simulink library "outp"  (R2021b)
settings: Solver=VariableStepAuto  StartTime=0.0  StopTime=10.0  RelTol=1e-3
undefined symbols (not defined in the file or in its folder): ENUM_PMMMODE_CHARGE, ENUM_PMMMODE_IDLE, ENUM_PMMMODE_INITIALIZE, ENUM_PMMMODE_POWERDOWN, ENUM_PMMMODE_SLEEP, Left, outp, slcm, TRUE
libraries: FVT_lib x1004, hcu_lib x4, simulink x1
(part 2 of 10)

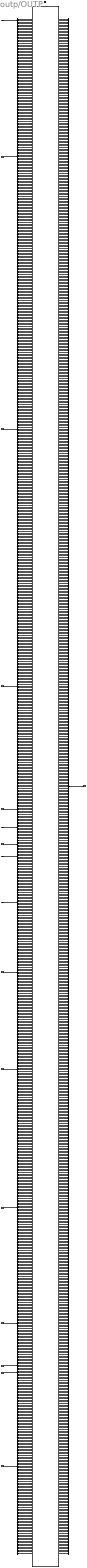
== system outp/OUTP ==
  BACC_outputs : Inport  OutDataTypeStr=Bus: BACC_outputs
  BAPM_outputs : Inport  Port=2  OutDataTypeStr=Bus: BAPM_outputs
  BBCM_outputs : Inport  Port=3  OutDataTypeStr=Bus: BBCM_outputs
  BDDM_outputs : Inport  Port=4  OutDataTypeStr=Bus: BDDM_outputs
  BDHP_outputs : Inport  Port=5  OutDataTypeStr=Bus: BDHP_outputs
  BDKC_outputs : Inport  Port=6  OutDataTypeStr=Bus: BDKC_outputs
  BDSC_outputs : Inport  Port=7  OutDataTypeStr=Bus: BDSC_outputs
  BNMM_outputs : Inport  Port=8  OutDataTypeStr=Bus: BNMM_outputs
  BPMM_outputs : Inport  Port=9  OutDataTypeStr=Bus: BPMM_outputs
  BSYS_outputs : Inport  Port=10  OutDataTypeStr=Bus: BSYS_outputs
  BTHC_outputs : Inport  Port=11  OutDataTypeStr=Bus: BTHC_outputs
  BTPM_outputs : Inport  Port=12  OutDataTypeStr=Bus: BTPM_outputs
  BTQD_outputs : Inport  Port=13  OutDataTypeStr=Bus: BTQD_outputs
  BTQR_outputs : Inport  Port=14  OutDataTypeStr=Bus: BTQR_outputs
  BV2L_outputs : Inport  Port=15  OutDataTypeStr=Bus: BV2L_outputs
  BVMC_outputs : Inport  Port=16  OutDataTypeStr=Bus: BVMC_outputs
  trig_OUTP : TriggerPort  TriggerType=function-call  VariantControl=(inherit)
  bus_creator : BusCreator  Inputs=1004
  bus_selector1 : BusSelector  OutputSignals=VACC_HVTHCMSysAvail_enum,VACC_LVBattVoltSta_enum,VACC_VehHVPwrAvail4THCM_W
  bus_selector10 : BusSelector  OutputSignals=VSYS_HWVer1_cnt,VSYS_HWVer2_cnt,VSYS_HWVer3_cnt,VSYS_CarModel1_cnt,VSYS_CarModel2_cnt,VSYS_CarModel3_cnt,VSYS_ECU1_cnt,VSYS_ECU2_cnt,VSYS_Major1_cnt,VSYS_Major2_cnt,VSYS_Minor1_cnt,VSYS_Minor2_cnt,VSYS_Patch1_cnt,VSYS_Patch2_cnt,VSYS_Country1_cnt,VSYS_Country2_cnt,VSYS_Variation_cnt,VSYS_Dash1_cnt,VSYS_Change1_cnt,VSYS_Change2_cnt,VSYS_Dash2_cnt,VSYS_SHA1_cnt,VSYS_SHA2_cnt,VSYS_SHA3_cnt,VSYS_SHA4_cnt,VSYS_SHA5_cnt,VSYS_SHA6_cnt,VSYS_SHA7_cnt,VSYS_SHA8_cnt,VSYS_NvWriteReqRisingEdge_flg,VSYS_FdcSlpReqRisingEdge_flg,VSYS_FdcSlpTime_sec,VSYS_PmicBootReason_enum,VSYS_WisrBootReason_raw32,VSYS_AcoreRebootCmdACK_flg,VSYS_CurrentNmState_enum,VSYS_ECUGen1_cnt,VSYS_ECUGen2_cnt,VSYS_PmicBootPath_raw32,VSYS_DrivingMode_cnt,VSYS_ModelYear_cnt,VSYS_Var4_cnt,VSYS_Var5_cnt
  bus_selector11 : BusSelector  OutputSignals=VTHC_FDCompCmd_rpm,VTHC_FDSOV1Cmd_flg,VTHC_FDSOV2Cmd_flg,VTHC_FDSOV3Cmd_flg,VTHC_FDEXV1Cmd_step,VTHC_FDEXV2Cmd_step,VTHC_FDSOTXVCmd_flg,VTHC_FDFWVCmd_flg,VTHC_FDTWVCmd_pct,VTHC_FDFrWPTCHeatPwrCmd_W,VTHC_CoolgFanActDuty_pct,VTHC_FDAGSCmd_enum,VTHC_FDEWP1Cmd_enum,VTHC_FDEWP2Cmd_enum,VTHC_FDEWP3Cmd_enum,VTHC_FDFrLeAPTCHeatPwrCmd_W,VTHC_FDFrRiAPTCHeatPwrCmd_W,VTHC_FDRrAPTCHeatPwrCmd_W,VTHC_FDBlowerCmd_pct,VTHC_BatteryMode_enum,VTHC_EDriveMode_enum,VTHC_CabinMode_enum,VTHC_CCUACLampSts_flg,VTHC_CCUAutoLampSts_flg,VTHC_CCUACMaxLampSts_flg,VTHC_CCUSyncLampSts_flg,VTHC_sigAirIntenZon1St_enum,VTHC_sigWindDirZon1St_enum,VTHC_sigRecircSt_flg,VTHC_sigSetTempZon1St_C,VTHC_sigSetTempZon2St_C,VTHC_sigClntTHvBattOut_C,VTHC_sigCbnSolarLeft_W,VTHC_sigClntTHvBattIn_C,VTHC_sigCbnSolarRight_W,VTHC_sigAmbAirT_C,VTHC_sigCbnAirT_C,VTHC_ACSubMode_enum,VTHC_FDRecyAutoCmd_enum,VTHC_ACModeMem_enum,VTHC_Face_flg,VTHC_Foot_flg,VTHC_Frost_flg,VTHC_FaceM_flg,VTHC_FootM_flg,VTHC_CCUSyncSts_flg,VTHC_ACForceOFF_flg,VTHC_RecAutoFlg_flg,VTHC_AirIntenZone1M_enum,VTHC_fdefog_flg,VTHC_sigSetTempZon2StM_C,VTHC_sigDfrstSt_flg,VTHC_FDCTHCAirIntZ3Sta_enum,VTHC_FDCTHCDrEVentModeSta_enum,VTHC_FDCTHCPsEVentModeSta_enum,VTHC_FDCTHCDrEVentZSta_enum,VTHC_FDCTHCCLEVentZSta_enum,VTHC_FDCTHCPsEVentZSta_enum,VTHC_FDCTHCCREVentZSta_enum,VTHC_FDCTHCDrEVentYSta_enum,VTHC_FDCTHCDrVentENSta_flg,VTHC_FDCTHCCLEVentYSta_enum,VTHC_FDCTHCCLVentENSta_flg,VTHC_FDCTHCPsEVentYSta_enum,VTHC_FDCTHCPsVentENSta_flg,VTHC_FDCTHCCREVentYSta_enum,VTHC_FDCTHCCRVentENSta_flg,VTHC_FDCTHCMAPTCForceOFFSta_flg,VTHC_DrVentEN_flg,VTHC_CLVentEN_flg,VTHC_PsVentEN_flg,VTHC_CRVentEN_flg,VTHC_FDCFGSAirIntSta_enum,VTHC_FDCFGSChSta_enum,VTHC_FDCFGSAirIntCmd_enum,VTHC_FDCFGSFuncSta_flg,VTHC_FDCFGSChCmd_enum,VTHC_FDCFGSIONSWSta_flg,VTHC_FDCFGSIONCmd_flg,VTHC_FDCFGSLearnCmd_enum,VTHC_FDCTHCMPreWPTCHeatSta_enum,VTHC_EWPBUflag1_flg,VTHC_EWPBUflag2_flg,VTHC_EWPBUflag3_flg
  bus_selector12 : BusSelector  OutputSignals=VTPM_LFBatWarn_flg,VTPM_RFBatWarn_flg,VTPM_LRBatWarn_flg,VTPM_RRBatWarn_flg,VTPM_LFWheelPress_raw8,VTPM_RFWheelPress_raw8,VTPM_LRWheelPress_raw8,VTPM_RRWheelPress_raw8,VTPM_LFWheelTemp_C,VTPM_RFWheelTemp_C,VTPM_LRWheelTemp_C,VTPM_RRWheelTemp_C,VTPM_LFSensorFail_flg,VTPM_RFSensorFail_flg,VTPM_LRSensorFail_flg,VTPM_RRSensorFail_flg,VTPM_LFWheelDebug_flg,VTPM_LRWheelDebug_flg,VTPM_RFWheelDebug_flg,VTPM_RRWheelDebug_flg,VTPM_TPMSResButtAllow_flg,VTPM_TPMSCaliButtAllow_flg,VTPM_LFPressIndi_enum,VTPM_RFPressIndi_enum,VTPM_LRPressIndi_enum,VTPM_RRPressIndi_enum,VTPM_TPMSWarnIndi_enum,VTPM_LFWheelTmpIndi_flg,VTPM_RFWheelTmpIndi_flg,VTPM_LRWheelTmpIndi_flg,VTPM_RRWheelTmpIndi_flg,VTPM_LFWheelPSW_raw8,VTPM_LRWheelPSW_raw8,VTPM_RFWheelPSW_raw8,VTPM_RRWheelPSW_raw8,VTPM_CWheelTips_enum,VTPM_AutoLTips_enum,VTPM_LFSensorMode_flg,VTPM_RFSensorMode_flg,VTPM_LRSensorMode_flg,VTPM_RRSensorMode_flg,VTPM_S1ID_raw32,VTPM_S2ID_raw32,VTPM_S3ID_raw32,VTPM_S4ID_raw32,VTPM_S1L_enum,VTPM_S2L_enum,VTPM_S3L_enum,VTPM_S4L_enum,VTPM_ALFin_flg,VTPM_LFP20_raw8,VTPM_RFP20_raw8,VTPM_LRP20_raw8,VTPM_RRP20_raw8,VTPM_FAT_flg,VTPM_IDin_raw32,VTPM_S1WheelDebugALTU_pct,VTPM_S2WheelDebugALTU_pct,VTPM_S3WheelDebugALTU_pct,VTPM_S4WheelDebugALTU_pct,VTPM_ID1messageALTU_raw8,VTPM_ID2messageALTU_raw8,VTPM_ID3messageALTU_raw8,VTPM_ID4messageALTU_raw8,VTPM_Chkfin_flg,VTPM_SetIDLoc_flg,VTPM_TPMSStorge_flg,VTPM_ChkStorge_flg,VTPM_TPMSResButt_flg,VTPM_LFPindi_enum,VTPM_RFPind_enum,VTPM_LRPindi_enum,VTPM_RRPindi_enum,VTPM_WriteChkLFID_raw,VTPM_WriteChkRFID_raw,VTPM_WriteChkLRID_raw,VTPM_WriteChkRRID_raw,VTPM_WriteChkfinLFID_raw,VTPM_WriteChkfinRFID_raw,VTPM_WriteChkfinLRID_raw,VTPM_WriteChkfinRRID_raw,VTPM_Flashchkdatavalid_enum,VTPM_Flashdatavalid_enum,VTPM_unlearnSfali_flg,VTPM_unlearnSfailvalid_enum,VTPM_Prepresstempvalid_enum,VTPM_FlashS1ID_raw,VTPM_FlashS2ID_raw,VTPM_FlashS3ID_raw,VTPM_FlashS4ID_raw,VTPM_FlashIDvalid_enum,VTPM_WritingCnt_enum,VTPM_TPMSTLCmd_flg,VTPM_LProgress_enum,VTPM_TPMSSensorIDRegStart_flg,VTPM_ModelVersion_raw,VTPM_ModelVersionChksum_raw
  bus_selector13 : BusSelector  OutputSignals=VTQD_ParkRequest_flg,VTQD_TqSourceFr_enum,VTQD_TqSourceRr_enum,VTQD_FrEDUAvailBrkRgnTq_Nm,VTQD_RrEDUAvailBrkRgnTq_Nm,VTQD_EVDriveMode_enum,VTQD_ShiftGearPosn_enum,VTQD_PButtonSta_enum,VTQD_FrActvDmpDisabReq_flg,VTQD_RrActvDmpDisabReq_flg,VTQD_FrRgnDecrSta_flg,VTQD_RrRgnDecrSta_flg,VTQD_DriverWhlTqDemFr_Nm,VTQD_DriverWhlTqDemRr_Nm,VTQD_FrEDUActTq_Nm,VTQD_RrEDUActTq_Nm,VTQD_FrEDURolRgnTq_Nm,VTQD_RrEDURolRgnTq_Nm,VTQD_FrEDUSpd_rpm,VTQD_RrEDUSpd_rpm,VTQD_FrEDUSpdValid_flg,VTQD_FrEDUAvailBrkRgnTqV_flg,VTQD_RrEDUSpdValid_flg,VTQD_RrEDUAvailBrkRgnTqV_flg,VTQD_RgnAbnorSta_flg,VTQD_PTCSPermSta_flg,VTQD_FrRgnPermSta_flg,VTQD_RrRgnPermSta_flg,VTQD_ExternalTqAllow_flg,VTQD_FrIdcMin_A,VTQD_FrIdcMax_A,VTQD_FrUdcMin_V,VTQD_FrUdcMax_V,VTQD_RrIdcMin_A,VTQD_RrIdcMax_A,VTQD_RrUdcMin_V,VTQD_RrUdcMax_V,VTQD_ReBrakeLPReq_flg,VTQD_ExtShftAllow_flg,VTQD_CreepON_flg,VTQD_EquivAccPedalSWSta_flg,VTQD_DriveProtEn_flg,VTQD_ActParkRequest_flg,VTQD_IVIPwrLockSta_enum,VTQD_ExtDoorAllow_flg,VTQD_OPDHoldLamp_flg,VTQD_SaveRegenMode_enum,VTQD_FDCVCURegenMode_enum,VTQD_SpdCtrlMode_enum,VTQD_SpdCtrlSta_flg,VTQD_SetSpd_kph,VTQD_VehActSpd_kph,VTQD_RegenLimIndSta_flg,VTQD_SetSpdLimWarn_flg
  bus_selector14 : BusSelector  OutputSignals=VTQR_FrTMTqReq_Nm,VTQR_RrTMTqReq_Nm
  bus_selector15 : BusSelector  OutputSignals=VV2L_ReqOBCV2LEna_enum,VV2L_ReqV2LIVIPopup_enum,VV2L_ReqV2LIVIDisChrg_enum,VV2L_ReqOBCExtrV2LEna_enum,VV2L_ReqOBCIntrV2LEna_enum,VV2L_HVPO120VGrpALDSt_enum,VV2L_HVPO120VGrpBLDSt_enum
  bus_selector16 : BusSelector  OutputSignals=VVMC_FeatSetSpdFinal_raw32,VVMC_VehicleSpeed_mph,VVMC_VehicleSpeed_kph,VVMC_MeterIndSpeed_raw32,VVMC_VMCAEBCtrlAvail_flg,VVMC_VMCACCCtrlAvail_flg,VVMC_VMCCCCtrlAvail_flg,VVMC_VMCMSACtrlAvail_flg,VVMC_FeatArbitrSta_enum,VVMC_FeatReqSpd_kph,VVMC_JerkPCT_pct,VVMC_LimitPCT_pct,VVMC_FrontRearSlipRatioCtrl_flg,VVMC_RearWhlSlipRatioCtrl_flg,VVMC_SingleWhlSlipRatioCtrl_flg,VVMC_LatAccCtrl_flg,VVMC_SafetyCtrl_flg,VVMC_SPD2ACCAct_flg,VVMC_AccCalcuPID_mps2,VVMC_ISOAccLimit_mps2,VVMC_ISODecLimit_mps2,VVMC_ISOJerkLimit_mps3,VVMC_ACCRequiredAccel_mps2,VVMC_DISCReqAcc_mps2,VVMC_FeatArbitrFinal_enum,VVMC_ActACCRequiredAccel_mps2,VVMC_LateralCtrl_flg,VVMC_ADASLKASta_enum,VVMC_LKAStrToqReq_Nm,VVMC_LKATOIFault_flg,VVMC_LKATOIAct_enum,VVMC_ADASAEBReq_enum,VVMC_ADASFaultSta_flg,VVMC_AEBVehHoldReq_flg,VVMC_ACCVehHoldReq_flg,VVMC_ADASDBSReq_enum,VVMC_ADASACCSta_enum,VVMC_ACCObjDist_m,VVMC_ACCObjRelSpd_mps,VVMC_TimeGapLevel_enum,VVMC_ACCJerkUpperLimit_mps3,VVMC_ACCComfortBandUpper_mps2,VVMC_ACCJerkLowerLimit_mps3,VVMC_ACCComfortBandLower_mps2,VVMC_ADASVehSpdLim_raw32,VVMC_ADASShftPosnReqA_flg,VVMC_ADASShftPosnReq_enum,VVMC_ADASForceIdle_flg,VVMC_HazardWarningReq_flg,VVMC_RightTurnLightReq_flg,VVMC_LeftTurnLightReq_flg,VVMC_ADASFCWSta_enum,VVMC_ADASLDWSta_enum,VVMC_ADASFltWrnReq_flg,VVMC_ACCObjDstLvl_enum,VVMC_ForceLowBeam_enum,VVMC_ACCTakeoverReq_flg,VVMC_ADASWarningMsg_enum,VVMC_ADASCAMSpdLim_enum,VVMC_TargetType_enum,VVMC_ADASSLIFSpdLim_enum,VVMC_LKAHODDisplayWarning_flg,VVMC_LKAHODSoundWarning_flg,VVMC_ADASLFCSta_enum,VVMC_ADASLaneModeL_enum,VVMC_ADASLaneModeR_enum,VVMC_ADASSLIFSta_enum,VVMC_ADASISASta_enum,VVMC_ADASLDWMute_flg,VVMC_ADASFCWMute_flg,VVMC_ADASLFCHandsOffWarning_enum,VVMC_LVDADisabled_flg,VVMC_LVDAMuteSta_enum,VVMC_LVDAFailinfo_flg,VVMC_LVDAWarning_flg,VVMC_LVDAACCStatusInformation_flg,VVMC_ADASLFCWarnSound_enum,VVMC_FCMACCmode_enum,VVMC_ADASLanetypeR_enum,VVMC_ADASLanetypeL_enum,VVMC_ADASLanecurveL_raw32,VVMC_ADASLanecurveR_raw32,VVMC_ADASAEBSta_enum,VVMC_FCMLDWRequest_enum,VVMC_FCMLDWFault_flg,VVMC_ACCCtrlAvail_flg,VVMC_ACCPedalOvrd_flg,VVMC_TimeGapCalcu_s,VVMC_CCCtrlSta_enum,VVMC_MSACtrlSta_enum,VVMC_APSCtrlAvail_flg,VVMC_APSActive_flg,VVMC_APSStaSys_enum,VVMC_APSDecReqA_flg,VVMC_APSDecReq_mps2,VVMC_APSReq_enum,VVMC_LongAcc_Gps,VVMC_CCMSASpdWar_flg,VVMC_IMUEnaCmd_flg,VVMC_CAASCtrlAvail_flg,VVMC_CAASActive_flg,VVMC_ExtraMSACtrlSta_enum,VVMC_CalibratedAccX_G,VVMC_CalibratedAccY_G,VVMC_CalibratedAccZ_G,VVMC_CalibratedGyroX_Dps,VVMC_CalibratedGyroY_Dps,VVMC_CalibratedGyroZ_Dps,VVMC_FDCVMCAPSVRqEPSCtrl_flg,VVMC_FDCVMCAPSAngleTarget_deg,VVMC_FDCVMCAPSRqEPSCtrl_flg,VVMC_FDCVMCAngCtrlTqWtGn_pct,VVMC_FDCVMCDrInpTqBstAct_flg,VVMC_FDCVMCMaxAngCtrlOutTqLim_Nm,VVMC_FDCVMCDrInpTqBstGn_pct
  bus_selector2 : BusSelector  OutputSignals=VAPM_VehSpeed_kph,VAPM_VehSpeedTimeOut_flg,VAPM_FSOffSw_enum,VAPM_FSOffSwTimeOut_flg,VAPM_ChrgPlugSta_enum,VAPM_PASDRMR_cm,VAPM_PASDRML_cm,VAPM_PASDRCR_cm,VAPM_PASDRCL_cm,VAPM_PASDFMR_cm,VAPM_PASDFML_cm,VAPM_PASDFCR_cm,VAPM_PASDFCL_cm,VAPM_APSDRLR_cm,VAPM_APSDRLL_cm,VAPM_APSDFLR_cm,VAPM_APSDFLL_cm,VAPM_PASAFCL_enum,VAPM_PASARMR_enum,VAPM_PASARML_enum,VAPM_PASARCR_enum,VAPM_PASARCL_enum,VAPM_PASAFMR_enum,VAPM_PASAFML_enum,VAPM_PASAFCR_enum,VAPM_USSStaRMR_flg,VAPM_USSStaRML_flg,VAPM_USSStaRLR_flg,VAPM_USSStaRLL_flg,VAPM_USSStaRCR_flg,VAPM_USSStaRCL_flg,VAPM_USSStaFMR_flg,VAPM_USSStaFML_flg,VAPM_USSStaFLR_flg,VAPM_USSStaFLL_flg,VAPM_USSStaFCR_flg,VAPM_USSStaFCL_flg,VAPM_Chime_enum,VAPM_SNSRLayout_enum,VAPM_StaFSya_flg,VAPM_ModOperation_enum,VAPM_BrkPedalPos_pct,VAPM_BrkPedalPosTimeOut_flg,VAPM_LFRawWhlSpeed_kph,VAPM_LFRawWhlSpeedTimeOut_flg,VAPM_RFRawWhlSpeed_kph,VAPM_RFRawWhlSpeedTimeOut_flg,VAPM_LRRawWhlSpeed_kph,VAPM_LRRawWhlSpeedTimeOut_flg,VAPM_RRRawWhlSpeed_kph,VAPM_RRRawWhlSpeedTimeOut_flg,VAPM_LFRawWhlSpeedV_flg,VAPM_LFRawWhlSpeedVTimeOut_flg,VAPM_RFRawWhlSpeedV_flg,VAPM_RFRawWhlSpeedVTimeOut_flg,VAPM_LRRawWhlSpeedV_flg,VAPM_LRRawWhlSpeedVTimeOut_flg,VAPM_RRRawWhlSpeedV_flg,VAPM_RRRawWhlSpeedVTimeOut_flg,VAPM_LFWhlRotDir_enum,VAPM_LFWhlRotDirTimeOut_flg,VAPM_RFWhlRotDir_enum,VAPM_RFWhlRotDirTimeOut_flg,VAPM_LRWhlRotDir_enum,VAPM_LRWhlRotDirTimeOut_flg,VAPM_RRWhlRotDir_enum,VAPM_RRWhlRotDirTimeOut_flg,VAPM_LFPulseCountV_flg,VAPM_LFPulseCountVTimeOut_flg,VAPM_RFPulseCountV_flg,VAPM_RFPulseCountVTimeOut_flg,VAPM_LRPulseCountV_flg,VAPM_LRPulseCountVTimeOut_flg,VAPM_RRPulseCountV_flg,VAPM_RRPulseCountVTimeOut_flg,VAPM_LFPulseCount_enum,VAPM_LFPulseCountTimeOut_flg,VAPM_RFPulseCount_enum,VAPM_RFPulseCountTimeOut_flg,VAPM_LRPulseCount_enum,VAPM_LRPulseCountTimeOut_flg,VAPM_RRPulseCount_enum,VAPM_RRPulseCountTimeOut_flg,VAPM_ShifterHandleCmd_enum,VAPM_ShifterHandleCmdTimeOut_flg,VAPM_DriIntend_enum,VAPM_DriIntendTimeOut_flg,VAPM_EPSAOIControl_enum,VAPM_EPSAOIControlTimeOut_flg,VAPM_SASAngle_Deg,VAPM_SASAngleTimeOut_flg,VAPM_SASSpeed_degps,VAPM_SASSpeedTimeOut_flg,VAPM_SASSpeedValid_flg,VAPM_SASSpeedValidTimeOut_flg,VAPM_SASCAL_flg,VAPM_SASCALTimeOut_flg,VAPM_SASV_flg,VAPM_SASVTimeOut_flg,VAPM_GRADE_Deg,VAPM_GRADETimeOut_flg,VAPM_YawRate_degps,VAPM_YawRateTimeOut_flg,VAPM_LatAccel_Gps,VAPM_LatAccelTimeOut_flg,VAPM_LongAccel_Gps,VAPM_LongAccelTimeOut_flg,VAPM_MCPressure_bar,VAPM_MCPressureTimeOut_flg,VAPM_YawRateV_flg,VAPM_YawRateVTimeOut_flg,VAPM_LatAccelV_flg,VAPM_LatAccelVTimeOut_flg,VAPM_LongAccelV_flg,VAPM_LongAccelVTimeOut_flg,VAPM_MCPressureV_bar,VAPM_MCPressureVTimeOut_flg,VAPM_BrkSwSta_flg,VAPM_BrkSwStaTimeOut_flg,VAPM_BrkSwV_flg,VAPM_BrkSwVTimeOut_flg,VAPM_ESCStandstill_flg,VAPM_ESCStandstillTimeOut_flg,VAPM_ESCAPSSta_enum,VAPM_ESCAPSStaTimeOut_flg,VAPM_EPBExtReleaseAvail_flg,VAPM_EPBExtReleaseAvailTimeOut_flg,VAPM_EPBExtApplyAvail_flg,VAPM_EPBExtApplyAvailTimeOut_flg,VAPM_EPBErrSta_enum,VAPM_EPBErrStaTimeOut_flg,VAPM_EPBSta_enum,VAPM_EPBStaTimeOut_flg,VAPM_AVMparkingcancel_enum,VAPM_AVMparkingcancelTimeOut_flg,VAPM_AVMparkingexcute_enum,VAPM_AVMparkingexcuteTimeOut_flg,VAPM_AVMParkingmode_enum,VAPM_AVMParkingmodeTimeOut_flg,VAPM_AVMErrSTA_flg,VAPM_AVMErrSTATimeOut_flg,VAPM_IVIStatus_flg,VAPM_IVIStatusTimeOut_flg,VAPM_CAASSw_enum,VAPM_CAASSwTimeOut_flg,VAPM_IVIScreen_enum,VAPM_IVIScreenTimeOut_flg,VAPM_ABSActive_flg,VAPM_ABSActiveTimeOut_flg,VAPM_TCSActive_flg,VAPM_TCSActiveTimeOut_flg,VAPM_DriverSeatBeltCmd_flg,VAPM_DriverSeatBeltCmdTimeOut_flg,VAPM_APSProgressPCT_pct,VAPM_APSRQDisplay_enum,VAPM_APSSWVer_enum,VAPM_APSHWVer_enum,VAPM_APSExitCondition_enum,VAPM_APSAngleTarget_Deg,VAPM_APSVRqEPASCtrl_flg,VAPM_APSRqEPASCtrl_flg,VAPM_CAASSta_enum,VAPM_DKCPDkeyAreaRAPSSta_enum,VAPM_DKCParkingModeCmd_enum,VAPM_PUIDLowPower_flg,VAPM_CAASVMCReqA_flg,VAPM_APSShiftPosnReq_enum,VAPM_APSSpeedCMD_kph,VAPM_APSVMCReqA_flg,VAPM_RAPSBCMLamp_enum,VAPM_RAPSBCMLockReq_flg,VAPM_APSPwrReq_enum,VAPM_RAPSErrWarnSta_enum,VAPM_RAPSErrLv1_flg,VAPM_IVIUserTakeOverAPSSta_flg
  bus_selector3 : BusSelector  OutputSignals=VBCM_AntitheftSta_enum,VBCM_TailgateRemote_enum,VBCM_HornCtrl_flg,VBCM_AllDoorSW_flg,VBCM_BCMDoorLockSta_flg,VBCM_AntitheftSeatFlod_flg,VBCM_HoodSW_flg,VBCM_TailgateSW_flg,VBCM_DrDoorSW_flg,VBCM_PsDoorSW_flg,VBCM_RLDoorSW_flg,VBCM_RRDoorSW_flg,VBCM_LockSetting_flg,VBCM_FrChargingDoorCtrl_enum,VBCM_RrChargingDoorCtrl_enum,VBCM_CrashDetd_flg,VBCM_CTDCtrl_enum,VBCM_DoorLockIND_flg,VBCM_CTDLockSW_flg,VBCM_Dimmer_pct,VBCM_DimmerEN_flg,VBCM_PosLamp_flg,VBCM_LBeam_flg,VBCM_HBeam_flg,VBCM_RrFogLamp_flg,VBCM_BrakeLamp_flg,VBCM_ReverseLamp_flg,VBCM_LDRL_flg,VBCM_RDRL_flg,VBCM_LBSD_flg,VBCM_RBSD_flg,VBCM_HazardSW_flg,VBCM_LTurnLP_flg,VBCM_RTurnLP_flg,VBCM_BCMBuzzerReq_flg,VBCM_MirrorCtrl_enum,VBCM_MirrorDefog_flg,VBCM_RrDefog_flg,VBCM_RoomLampH_flg,VBCM_RoomLampL_flg,VBCM_TrunkRel_flg,VBCM_TailgateHDSW_flg,VBCM_FrWiperL_flg,VBCM_FrWiperH_flg,VBCM_RrWiper_flg,VBCM_WasherCtrl_enum,VBCM_WiperFixMode_flg,VBCM_AmbLightBreath1_enum,VBCM_AmbLightBreath2_enum,VBCM_AmbLightBreath3_enum,VBCM_AmbLightBreath4_enum,VBCM_AmbLightBreath5_enum,VBCM_AmbLightBreath6_enum,VBCM_AmbLightBrightness1_enum,VBCM_AmbLightBrightness2_enum,VBCM_AmbLightBrightness3_enum,VBCM_AmbLightBrightness4_enum,VBCM_AmbLightBrightness5_enum,VBCM_AmbLightBrightness6_enum,VBCM_AmbLightColor1_enum,VBCM_AmbLightColor2_enum,VBCM_AmbLightColor3_enum,VBCM_AmbLightColor4_enum,VBCM_AmbLightColor5_enum,VBCM_AmbLightColor6_enum,VBCM_LampPwr_flg,VBCM_SPTGDet_flg,VBCM_APSOpenPTG_flg,VBCM_FollowMe_flg,VBCM_IVIRST_flg,VBCM_CountAlarm_enum,VBCM_MFSWTri_flg,VBCM_MirrorFlodPos_flg,VBCM_FuelDoorPos_flg,VBCM_MFRDNBrightReq_pct,VBCM_PTGInnerSW2_enum,VBCM_DrvWdwCtrlCmd_pct,VBCM_PasWdwCtrlCmd_pct,VBCM_DrRWdwCtrlCmd_pct,VBCM_PsRWdwCtrlCmd_pct,VBCM_APMDoorControlSta_flg,VBCM_AmbFunEN_flg,VBCM_AmbWelEN_flg,VBCM_AmbDimEN_flg,VBCM_AmbLinkDriSta_flg,VBCM_AmbPwrWarnEN_flg,VBCM_AmbODAEN_flg,VBCM_AmbColorSta_enum,VBCM_AmbBrightSta_enum,VBCM_LockAlarm_enum,VBCM_ATCtrl_enum,VBCM_fUnlockSingle_flg,VBCM_UserNow_enum,VBCM_AmbFunENFlash_enum,VBCM_AmbWelENFlash_enum,VBCM_AmbDimENFlash_enum,VBCM_AmbLinkDriStaFlash_enum,VBCM_AmbPwrWarnENFlash_enum,VBCM_AmbODAENFlash_enum,VBCM_AmbColorSta1_enum,VBCM_AmbColorSta2_enum,VBCM_AmbColorSta3_enum,VBCM_AmbColorSta4_enum,VBCM_AmbColorSta5_enum,VBCM_AmbColorSta7_enum,VBCM_AmbBrightnessSta1_enum,VBCM_AmbBrightnessSta2_enum,VBCM_AmbBrightnessSta3_enum,VBCM_AmbBrightnessSta4_enum,VBCM_AmbBrightnessSta5_enum,VBCM_AmbBrightnessSta7_enum,VBCM_HazardIND_flg,VBCM_DimSwSta_flg,VBCM_PassSWSta_flg,VBCM_FWipSwSta_enum,VBCM_FWasSwSta_enum,VBCM_TurnSwSta_enum,VBCM_TurnSwTSetSta_enum,VBCM_SPTGENFun_flg,VBCM_SPTGENFunMem_enum,VBCM_OutMode_enum,VBCM_TurnSwTimeSetSta123_enum,VBCM_TurnSwTimeSetSta457_enum,VBCM_FDLHandleLampCmd_flg,VBCM_FDRHandleLampCmd_flg,VBCM_FDHandleCmd_enum,VBCM_HBeamADB_flg,VBCM_WalkInUnLkENMem_enum,VBCM_WalkOutLkENMem_enum,VBCM_RmLpModeENMem_enum,VBCM_LockSettingStaMem_enum,VBCM_FollowMeENMem_enum,VBCM_WalkInUnLkENFunSta_flg,VBCM_WalkOutLkENFunSta_flg,VBCM_RmLpModeENFunSta_flg,VBCM_FollowMeENFunSta_flg,VBCM_HoodRelCmd_flg,VBCM_WelcomeLight_enum,VBCM_PTGOpenHeightSta_enum,VBCM_UserHeightSet_cnt,VBCM_PTGUserHeight1_cnt,VBCM_PTGUserHeight2_cnt,VBCM_PTGUserHeight3_cnt,VBCM_PTGUserHeight4_cnt,VBCM_PTGUserHeight5_cnt,VBCM_PTGUserHeight7_cnt,VBCM_PTGOpenHeight12_enum,VBCM_PTGOpenHeight34_enum,VBCM_PTGOpenHeight57_enum,VBCM_SenstivityPosnCmd_enum,VBCM_TimeGapLevelSta_enum,VBCM_ACCLevelMem12_enum,VBCM_ACCLevelMem34_enum,VBCM_ACCLevelMem57_enum,VBCM_LRightStaCmd_flg,VBCM_LLeftStaCmd_flg,VBCM_AutoLockSta_flg,VBCM_AutoLockMem_enum,VBCM_AutoUnlockSta_flg,VBCM_AutoUnlockMem_enum,VBCM_HMIKey1FuncSta_enum,VBCM_HMIKey2FuncSta_enum,VBCM_HMIKey3FuncSta_enum,VBCM_HMIKey4FuncSta_enum,VBCM_HMIKey5FuncSta_enum,VBCM_HMIKey6FuncSta_enum,VBCM_HMIKey7FuncSta_enum,VBCM_HMIKey8FuncSta_enum,VBCM_AutoWipHSpdENSta_flg,VBCM_DrvWdwReqAP_enum,VBCM_PasWdwReqAP_enum,VBCM_DrRWdwReqAP_enum,VBCM_PsRWdwReqAP_enum,VBCM_CLWinLockDrSta_flg,VBCM_CLWinLockDrStaMem_enum,VBCM_WinLFOpenedSta_pct,VBCM_WinRFOpenedSta_pct,VBCM_WinLROpenedSta_pct,VBCM_WinRROpenedSta_pct,VBCM_FoxPiSwitchSta_enum,VBCM_FoxPiLampSta_enum
  bus_selector4 : BusSelector  OutputSignals=VDDM_C3BMS6RCDTC_raw32,VDDM_C3BMS6CSDTC_raw32,VDDM_C3BMS6LCDTC_raw32,VDDM_C3BMS1RCDTC_raw32,VDDM_C3BMS1CSDTC_raw32,VDDM_C3BMS1LCDTC_raw32,VDDM_C3CCU1RCDTC_raw32,VDDM_C3CCU1CSDTC_raw32,VDDM_C3CCU1LCDTC_raw32,VDDM_C3CCU2RCDTC_raw32,VDDM_C3CCU2CSDTC_raw32,VDDM_C3CCU2LCDTC_raw32,VDDM_C1ABM1RCDTC_raw32,VDDM_C1ABM1CSDTC_raw32,VDDM_C1ABM1LCDTC_raw32,VDDM_Lv1ErrDTC_raw32,VDDM_Lv2ErrDTC_raw32,VDDM_Lv3ErrDTC_raw32,VDDM_Lv4ErrDTC_raw32,VDDM_BrkSWErrDTC_raw32,VDDM_BrkSWNoBacDTC_raw32,VDDM_KeyAuthDTC_raw32,VDDM_ONtoRdyDTC_raw32,VDDM_HVB4PreDTC_raw32,VDDM_MCU4PreDTC_raw32,VDDM_DCDC4PreDTC_raw32,VDDM_HVRlyCloDTC_raw32,VDDM_BMSRdyDTC_raw32,VDDM_DCDCEnaDTC_raw32,VDDM_HiLvSaChkDTC_raw32,VDDM_MidLvSaChkDTC_raw32,VDDM_MCUDisDTC_raw32,VDDM_DCDCDisDTC_raw32,VDDM_HVRlyOpDTC_raw32,VDDM_MCUActDTC_raw32,VDDM_OBC4PreDTC_raw32,VDDM_IniLVLoDTC_raw32,VDDM_LVSupLoDTC_raw32,VDDM_LVSupHiDTC_raw32,VDDM_DrStSWDTC_raw32,VDDM_FLDoorSWDTC_raw32,VDDM_RLDoorSWDTC_raw32,VDDM_FRDoorSWDTC_raw32,VDDM_RRDoorSWDTC_raw32,VDDM_HoodSWDTC_raw32,VDDM_TailgaSWDTC_raw32,VDDM_EDriveSysErrVCUErr_flg,VDDM_VehMalfunLevel_enum,VDDM_APS1SigOoRDTC_raw32,VDDM_APS2SigOoRDTC_raw32,VDDM_APSCorrErrDTC_raw32,VDDM_MCUF1NoComDTC_raw32,VDDM_MCUR1NoComDTC_raw32,VDDM_Shifter1NoComDTC_raw32,VDDM_ESC7NoComDTC_raw32,VDDM_ESC1NoComDTC_raw32,VDDM_ESC5NoComDTC_raw32,VDDM_EnterNewOperCyc_flg,VDDM_DiagHCrashDTC_raw32,VDDM_DiagFLTSDTC_raw32,VDDM_DiagFRTSDTC_raw32,VDDM_DiagRLTSDTC_raw32,VDDM_DiagRRTSDTC_raw32,VDDM_FCLUSSDTC_raw32,VDDM_FMLUSSDTC_raw32,VDDM_FMRUSSDTC_raw32,VDDM_FCRUSSDTC_raw32,VDDM_RCLUSSDTC_raw32,VDDM_RMLUSSDTC_raw32,VDDM_RMRUSSDTC_raw32,VDDM_RCRUSSDTC_raw32,VDDM_FLLUSSDTC_raw32,VDDM_FLRUSSDTC_raw32,VDDM_RLLUSSDTC_raw32,VDDM_RLRUSSDTC_raw32,VDDM_FCM2NoComDTC_raw32,VDDM_FCM2RCErrDTC_raw32,VDDM_FCM2CSErrDTC_raw32,VDDM_FCM3NoComDTC_raw32,VDDM_FCM3RCErrDTC_raw32,VDDM_FCM3CSErrDTC_raw32,VDDM_FCM4NoComDTC_raw32,VDDM_FCM4CSErrDTC_raw32,VDDM_FCM5NoComDTC_raw32,VDDM_FCM5CSErrDTC_raw32,VDDM_ZoneSCPNoComDTC_raw32,VDDM_BMSSigErrDetDTC_raw32,VDDM_FCMACCSigErrDetDTC_raw32,VDDM_FrMCUSigErrDetDTC_raw32,VDDM_RrMCUSigErrDetDTC_raw32,VDDM_CCUSigErrDetDTC_raw32,VDDM_ACCAccelCmdErrDetDTC_raw32,VDDM_ACCMalfuncDetDTC_raw32,VDDM_CCMalfuncDetDTC_raw32,VDDM_MSAMalfuncDetDTC_raw32,VDDM_ISAMalfuncDetDTC_raw32,VDDM_MCUF1RCErrDTC_raw32,VDDM_MCUR1RCErrDTC_raw32,VDDM_MCUF1CSErrDTC_raw32,VDDM_MCUR1CSErrDTC_raw32,VDDM_Shifter1RCErrDTC_raw32,VDDM_Shifter1CSErrDTC_raw32,VDDM_ESC7RCErrDTC_raw32,VDDM_ESC7CSErrDTC_raw32,VDDM_ESC1RCErrDTC_raw32,VDDM_ESC1CSErrDTC_raw32,VDDM_ESC5RCErrDTC_raw32,VDDM_ESC5CSErrDTC_raw32,VDDM_FrMCUTqErrDTC_raw32,VDDM_RrMCUTqErrDTC_raw32,VDDM_LFBatwarnDTC_raw32,VDDM_RFBatwarnDTC_raw32,VDDM_LRBatwarnDTC_raw32,VDDM_RRBatwarnDTC_raw32,VDDM_LFPressIndiDTC_raw32,VDDM_RFPressIndiDTC_raw32,VDDM_LRPressIndiDTC_raw32,VDDM_RRPressIndiDTC_raw32,VDDM_LFWheelTmpHighDTC_raw32,VDDM_RFWheelTmpHighDTC_raw32,VDDM_LRWheelTmpHighDTC_raw32,VDDM_RRWheelTmpHighDTC_raw32,VDDM_LFSensorFailDTC_raw32,VDDM_RFSensorFailDTC_raw32,VDDM_LRSensorFailDTC_raw32,VDDM_RRSensorFailDTC_raw32,VDDM_C1EPAS2LCDTC_raw32,VDDM_5vAPS1PwrErrDTC_raw32,VDDM_5vAPS2PwrErrDTC_raw32,VDDM_EPBLockTODTC_raw32,VDDM_EPBUnlockTODTC_raw32,VDDM_LimpHomeActTmp_flg,VDDM_DTCDetect_enum,VDDM_EngagePFail_flg,VDDM_DisengagePFail_flg,VDDM_VCURAPSErrLv2_flg,VDDM_VCURAPSErrLv3_flg,VDDM_EDriveSysErrShifterErr_flg,VDDM_LVSysErrPwrOutErr_flg,VDDM_HVRlyOpFail_flg,VDDM_MCUActDisFail_flg,VDDM_VCUBrkSWSta_enum,VDDM_VCUFLDoorSta_flg,VDDM_VCUFRDoorSta_flg,VDDM_VCURLDoorSta_flg,VDDM_VCURRDoorSta_flg,VDDM_SysAllowReadySta_flg,VDDM_VCUHoodSWSta_flg,VDDM_VCUTailgateSWSta_flg,VDDM_CAN1BusErrorDTC_raw32,VDDM_CAN2BusErrorDTC_raw32,VDDM_CAN3BusErrorDTC_raw32,VDDM_CAN4BusErrorDTC_raw32,VDDM_CAN5BusErrorDTC_raw32,VDDM_CAN6BusErrorDTC_raw32
  bus_selector5 : BusSelector  OutputSignals=VDHP_ActAPSPosn_pct,VDHP_EAPS1MIN_pct,VDHP_EAPS2MIN_pct,VDHP_ResetPedalZeroPosStart_flg,VDHP_EAPS1NRM_pct,VDHP_EAPS2NRM_pct
  bus_selector6 : BusSelector  OutputSignals=VDKC_DKCTimeSN_cnt,VDKC_DKCAuthSta_enum,VDKC_TimeSNDKCFbk_cnt,VDKC_KeyMissSta_flg,VDKC_KeyModeSta_enum,VDKC_DkeyShowIVISta_enum,VDKC_KeyAreaPS_enum,VDKC_KeyAreaLockUnlock_enum,VDKC_PCommandToBCM_enum,VDKC_DKeyWelcomeSta_enum,VDKC_KeyAreaPTG_enum,VDKC_KeyAreaSPTGSta_enum,VDKC_UIDLowPowerSta_enum,VDKC_DkeyAreaRAPSSta_enum,VDKC_ParkingModeCmd_enum,VDKC_KeyNumSta_enum,VDKC_KeyTypeSta_enum,VDKC_FDCDKCAllowSleep_flg
  bus_selector7 : BusSelector  OutputSignals=VDSC_DISCTurn_flg,VDSC_DISCTargetSpd_kph,VDSC_DISCSta_enum,VDSC_DISCButtSta_flg
  bus_selector8 : BusSelector  OutputSignals=VNMM_AllCANTxReq_flg,VNMM_NMmTxReq_flg,VNMM_Awake_enum,VNMM_CSB_flg,VNMM_ErrorState_enum,VNMM_NodeID_enum,VNMM_PNI_flg,VNMM_RptMsgReq_flg,VNMM_WakeUp_enum,VNMM_ActiveWU_flg,VNMM_SysNMmSta_enum,VNMM_NetworkReq_flg
  bus_selector9 : BusSelector  OutputSignals=VPMM_PowerUpState_enum,VPMM_PowerDownState_enum,VPMM_PowerUpFault_enum,VPMM_PowerDownFault_enum,VPMM_ActiveDischargeReq_flg,VPMM_DCDCEnaReq_flg,VPMM_DCDCVoltSetpoint_V,VPMM_HVBatCnctReq_flg,VPMM_HVSysReadyToCharge_enum,VPMM_PowerSta_enum,VPMM_LVPwrSta_flg,VPMM_HVPwrSta_flg,VPMM_SysPowerMode_enum,VPMM_FrMCUEnaReq_flg,VPMM_RrMCUEnaReq_flg,VPMM_DrivetrainSelect_enum,VPMM_DrSeatSta_enum,VPMM_PwrStaSelect_enum,VPMM_PwrStaConstraint_enum,VPMM_TCountSta_enum,VPMM_PwrUpReq_enum,VPMM_PwrDownReq_enum,VPMM_LowSOCWarn_enum,VPMM_ReVehThdChkSta_enum,VPMM_EvccAplusPwrUpReq_flg,VPMM_PwrStaONTOPopReq_flg,VPMM_IVIPwrStaONTOPopT_s,VPMM_LVChrgHoldTtimer_s,VPMM_LVBattChrgTimeCnt_s,VPMM_SilentChkAllowSleep_flg,VPMM_TimerAllowSleep_flg,VPMM_FDADC12VDetAvg_mV,VPMM_PMMAllowECUSleep_flg,VPMM_LVSilentChrgSta_enum,VPMM_LVSilentChrgReq_flg,VPMM_LVSilentChrgLv_enum,VPMM_CtrlFrPwrStbA1P_flg,VPMM_CtrlFrRC1_flg,VPMM_CtrlFrBMSCCUCIR_flg,VPMM_CtrlFrEDUINVERTER_flg,VPMM_HWResetSta_enum,VPMM_CtrlDrPwrStbA2_flg,VPMM_PwrStaTOSta_enum,VPMM_Sched_ChgTOSta_enum,VPMM_PwrReq_OTA_enum,VPMM_OTAPwrReqOFFChkSta_enum,VPMM_OTAPwrReqStdChkSta_enum,VPMM_PwrReqRAPSAvail_flg
  outpmodule : Subsystem
  BOUTP_outputs : Outport  OutDataTypeStr=Bus: BOUTP_outputs
  wires:
  bus_selector9/42 -> outpmodule/596(VPMM_CtrlDrPwrStbA2_flg)  "<VPMM_CtrlDrPwrStbA2_flg>"
  bus_selector9/39 -> outpmodule/593(VPMM_CtrlFrBMSCCUCIR_flg)  "<VPMM_CtrlFrBMSCCUCIR_flg>"
  bus_selector9/36 -> outpmodule/590(VPMM_LVSilentChrgLv_enum)  "<VPMM_LVSilentChrgLv_enum>"
  bus_selector9/35 -> outpmodule/589(VPMM_LVSilentChrgReq_flg)  "<VPMM_LVSilentChrgReq_flg>"
  bus_selector9/29 -> outpmodule/583(VPMM_LVBattChrgTimeCnt_s)  "<VPMM_LVBattChrgTimeCnt_s>"
  bus_selector9/26 -> outpmodule/580(VPMM_PwrStaONTOPopReq_flg)  "<VPMM_PwrStaONTOPopReq_flg>"
  bus_selector9/27 -> outpmodule/581(VPMM_IVIPwrStaONTOPopT_s)  "<VPMM_IVIPwrStaONTOPopT_s>"
  bus_selector9/20 -> outpmodule/574(VPMM_TCountSta_enum)  "<VPMM_TCountSta_enum>"
  bus_selector9/22 -> outpmodule/576(VPMM_PwrDownReq_enum)  "<VPMM_PwrDownReq_enum>"
  bus_selector9/21 -> outpmodule/575(VPMM_PwrUpReq_enum)  "<VPMM_PwrUpReq_enum>"
  bus_selector9/18 -> outpmodule/572(VPMM_PwrStaSelect_enum)  "<VPMM_PwrStaSelect_enum>"
  bus_selector9/17 -> outpmodule/571(VPMM_DrSeatSta_enum)  "<VPMM_DrSeatSta_enum>"
  bus_selector9/13 -> outpmodule/567(VPMM_SysPowerMode_enum)  "<VPMM_SysPowerMode_enum>"
  bus_selector9/10 -> outpmodule/564(VPMM_PowerSta_enum)  "<VPMM_PowerSta_enum>"
  bus_selector9/11 -> outpmodule/565(VPMM_LVPwrSta_flg)  "<VPMM_LVPwrSta_flg>"
  bus_selector9/9 -> outpmodule/563(VPMM_HVSysReadyToCharge_enum)  "<VPMM_HVSysReadyToCharge_enum>"
  bus_selector9/7 -> outpmodule/561(VPMM_DCDCVoltSetpoint_V)  "<VPMM_DCDCVoltSetpoint_V>"
  bus_selector9/8 -> outpmodule/562(VPMM_HVBatCnctReq_flg)  "<VPMM_HVBatCnctReq_flg>"
  BPMM_outputs/1 -> bus_selector9/1
  bus_selector9/6 -> outpmodule/560(VPMM_DCDCEnaReq_flg)  "<VPMM_DCDCEnaReq_flg>"
  bus_selector9/4 -> outpmodule/558(VPMM_PowerDownFault_enum)  "<VPMM_PowerDownFault_enum>"
  bus_selector9/2 -> outpmodule/556(VPMM_PowerDownState_enum)  "<VPMM_PowerDownState_enum>"
  bus_selector9/1 -> outpmodule/555(VPMM_PowerUpState_enum)  "<VPMM_PowerUpState_enum>"
  bus_selector8/7 -> outpmodule/549(VNMM_PNI_flg)  "<VNMM_PNI_flg>"
  bus_selector8/8 -> outpmodule/550(VNMM_RptMsgReq_flg)  "<VNMM_RptMsgReq_flg>"
  bus_selector8/10 -> outpmodule/552(VNMM_ActiveWU_flg)  "<VNMM_ActiveWU_flg>"
  bus_selector16/85 -> outpmodule/974(VVMC_FCMLDWFault_flg)  "<VVMC_FCMLDWFault_flg>"
  bus_selector16/84 -> outpmodule/973(VVMC_FCMLDWRequest_enum)  "<VVMC_FCMLDWRequest_enum>"
  bus_selector16/81 -> outpmodule/970(VVMC_ADASLanecurveL_raw32)  "<VVMC_ADASLanecurveL_raw32>"
  bus_selector16/83 -> outpmodule/972(VVMC_ADASAEBSta_enum)  "<VVMC_ADASAEBSta_enum>"
  bus_selector16/80 -> outpmodule/969(VVMC_ADASLanetypeL_enum)  "<VVMC_ADASLanetypeL_enum>"
  bus_selector16/76 -> outpmodule/965(VVMC_LVDAACCStatusInformation_flg)  "<VVMC_LVDAACCStatusInformation_flg>"
  bus_selector16/77 -> outpmodule/966(VVMC_ADASLFCWarnSound_enum)  "<VVMC_ADASLFCWarnSound_enum>"
  bus_selector16/71 -> outpmodule/960(VVMC_ADASLFCHandsOffWarning_enum)  "<VVMC_ADASLFCHandsOffWarning_enum>"
  bus_selector16/69 -> outpmodule/958(VVMC_ADASLDWMute_flg)  "<VVMC_ADASLDWMute_flg>"
  bus_selector16/65 -> outpmodule/954(VVMC_ADASLaneModeL_enum)  "<VVMC_ADASLaneModeL_enum>"
  bus_selector16/62 -> outpmodule/951(VVMC_LKAHODDisplayWarning_flg)  "<VVMC_LKAHODDisplayWarning_flg>"
  bus_selector16/55 -> outpmodule/944(VVMC_ACCObjDstLvl_enum)  "<VVMC_ACCObjDstLvl_enum>"
  bus_selector16/50 -> outpmodule/939(VVMC_RightTurnLightReq_flg)  "<VVMC_RightTurnLightReq_flg>"
  bus_selector9/43 -> outpmodule/597(VPMM_PwrStaTOSta_enum)  "<VPMM_PwrStaTOSta_enum>"
  bus_selector16/49 -> outpmodule/938(VVMC_HazardWarningReq_flg)  "<VVMC_HazardWarningReq_flg>"
  bus_selector16/47 -> outpmodule/936(VVMC_ADASShftPosnReq_enum)  "<VVMC_ADASShftPosnReq_enum>"
  bus_selector16/45 -> outpmodule/934(VVMC_ADASVehSpdLim_raw32)  "<VVMC_ADASVehSpdLim_raw32>"
  bus_selector16/36 -> outpmodule/925(VVMC_ADASDBSReq_enum)  "<VVMC_ADASDBSReq_enum>"
  bus_selector16/35 -> outpmodule/924(VVMC_ACCVehHoldReq_flg)  "<VVMC_ACCVehHoldReq_flg>"
  bus_selector16/31 -> outpmodule/920(VVMC_LKATOIAct_enum)  "<VVMC_LKATOIAct_enum>"
  bus_selector16/32 -> outpmodule/921(VVMC_ADASAEBReq_enum)  "<VVMC_ADASAEBReq_enum>"
  bus_selector16/28 -> outpmodule/917(VVMC_ADASLKASta_enum)  "<VVMC_ADASLKASta_enum>"
  bus_selector16/26 -> outpmodule/915(VVMC_ActACCRequiredAccel_mps2)  "<VVMC_ActACCRequiredAccel_mps2>"
  bus_selector16/23 -> outpmodule/912(VVMC_ACCRequiredAccel_mps2)  "<VVMC_ACCRequiredAccel_mps2>"
  bus_selector16/19 -> outpmodule/908(VVMC_AccCalcuPID_mps2)  "<VVMC_AccCalcuPID_mps2>"
  bus_selector16/11 -> outpmodule/900(VVMC_JerkPCT_pct)  "<VVMC_JerkPCT_pct>"
  bus_selector16/7 -> outpmodule/896(VVMC_VMCCCCtrlAvail_flg)  "<VVMC_VMCCCCtrlAvail_flg>"
  bus_selector16/9 -> outpmodule/898(VVMC_FeatArbitrSta_enum)  "<VVMC_FeatArbitrSta_enum>"
  bus_selector16/5 -> outpmodule/894(VVMC_VMCAEBCtrlAvail_flg)  "<VVMC_VMCAEBCtrlAvail_flg>"
  bus_selector16/4 -> outpmodule/893(VVMC_MeterIndSpeed_raw32)  "<VVMC_MeterIndSpeed_raw32>"
  bus_selector16/101 -> outpmodule/990(VVMC_CAASActive_flg)  "<VVMC_CAASActive_flg>"
  bus_selector16/99 -> outpmodule/988(VVMC_IMUEnaCmd_flg)  "<VVMC_IMUEnaCmd_flg>"
  bus_selector16/98 -> outpmodule/987(VVMC_CCMSASpdWar_flg)  "<VVMC_CCMSASpdWar_flg>"
  bus_selector16/91 -> outpmodule/980(VVMC_APSCtrlAvail_flg)  "<VVMC_APSCtrlAvail_flg>"
  bus_selector16/90 -> outpmodule/979(VVMC_MSACtrlSta_enum)  "<VVMC_MSACtrlSta_enum>"
  outpmodule/1004(VOUTP_FDCVMCDrInpTqBstGn_pct) -> bus_creator/1004
  outpmodule/998(VOUTP_FDCVMCAPSVRqEPSCtrl_flg) -> bus_creator/998
  outpmodule/997(VOUTP_CalibratedGyroZ_Dps) -> bus_creator/997
  bus_selector8/5 -> outpmodule/547(VNMM_ErrorState_enum)  "<VNMM_ErrorState_enum>"
  outpmodule/992(VOUTP_CalibratedAccX_G) -> bus_creator/992
  outpmodule/989(VOUTP_CAASCtrlAvail_flg) -> bus_creator/989
  bus_selector16/97 -> outpmodule/986(VVMC_LongAcc_Gps)  "<VVMC_LongAcc_Gps>"
  outpmodule/988(VOUTP_IMUEnaCmd_flg) -> bus_creator/988
  outpmodule/982(VOUTP_APSStaSys_enum) -> bus_creator/982
  outpmodule/983(VOUTP_APSDecReqA_flg) -> bus_creator/983
  outpmodule/975(VOUTP_ACCCtrlAvail_flg) -> bus_creator/975
  outpmodule/974(VOUTP_FCMLDWFault_flg) -> bus_creator/974
  bus_selector9/3 -> outpmodule/557(VPMM_PowerUpFault_enum)  "<VPMM_PowerUpFault_enum>"
  outpmodule/969(VOUTP_ADASLanetypeL_enum) -> bus_creator/969
  outpmodule/970(VOUTP_ADASLanecurveL_raw32) -> bus_creator/970
  outpmodule/966(VOUTP_ADASLFCWarnSound_enum) -> bus_creator/966
  outpmodule/968(VOUTP_ADASLanetypeR_enum) -> bus_creator/968
  outpmodule/964(VOUTP_LVDAWarning_flg) -> bus_creator/964
  outpmodule/965(VOUTP_LVDAACCStatusInformation_flg) -> bus_creator/965
  bus_selector4/140 -> outpmodule/499(VDDM_HVRlyOpFail_flg)  "<VDDM_HVRlyOpFail_flg>"
  bus_selector9/46 -> outpmodule/600(VPMM_OTAPwrReqOFFChkSta_enum)  "<VPMM_OTAPwrReqOFFChkSta_enum>"
  outpmodule/285(VOUTP_AmbBrightnessSta2_enum) -> bus_creator/285
  outpmodule/282(VOUTP_AmbColorSta5_enum) -> bus_creator/282
  outpmodule/278(VOUTP_AmbColorSta1_enum) -> bus_creator/278
  outpmodule/276(VOUTP_AmbPwrWarnENFlash_enum) -> bus_creator/276
  outpmodule/274(VOUTP_AmbDimENFlash_enum) -> bus_creator/274
  outpmodule/270(VOUTP_fUnlockSingle_flg) -> bus_creator/270
  bus_selector16/72 -> outpmodule/961(VVMC_LVDADisabled_flg)  "<VVMC_LVDADisabled_flg>"
  outpmodule/272(VOUTP_AmbFunENFlash_enum) -> bus_creator/272
  outpmodule/271(VOUTP_UserNow_enum) -> bus_creator/271
  outpmodule/269(VOUTP_ATCtrl_enum) -> bus_creator/269
  outpmodule/264(VOUTP_AmbPwrWarnEN_flg) -> bus_creator/264
  outpmodule/262(VOUTP_AmbDimEN_flg) -> bus_creator/262
  outpmodule/261(VOUTP_AmbWelEN_flg) -> bus_creator/261
  outpmodule/258(VOUTP_PsRWdwCtrlCmd_pct) -> bus_creator/258
  outpmodule/257(VOUTP_DrRWdwCtrlCmd_pct) -> bus_creator/257
  outpmodule/249(VOUTP_CountAlarm_enum) -> bus_creator/249
  outpmodule/247(VOUTP_FollowMe_flg) -> bus_creator/247
  outpmodule/244(VOUTP_LampPwr_flg) -> bus_creator/244
  outpmodule/1000(VOUTP_FDCVMCAPSRqEPSCtrl_flg) -> bus_creator/1000
  outpmodule/245(VOUTP_SPTGDet_flg) -> bus_creator/245
  outpmodule/243(VOUTP_AmbLightColor6_enum) -> bus_creator/243
  outpmodule/239(VOUTP_AmbLightColor2_enum) -> bus_creator/239
  outpmodule/237(VOUTP_AmbLightBrightness6_enum) -> bus_creator/237
  outpmodule/236(VOUTP_AmbLightBrightness5_enum) -> bus_creator/236
  outpmodule/233(VOUTP_AmbLightBrightness2_enum) -> bus_creator/233
  outpmodule/305(VOUTP_HBeamADB_flg) -> bus_creator/305
  outpmodule/298(VOUTP_SPTGENFunMem_enum) -> bus_creator/298
  outpmodule/296(VOUTP_TurnSwTSetSta_enum) -> bus_creator/296
  outpmodule/297(VOUTP_SPTGENFun_flg) -> bus_creator/297
  outpmodule/295(VOUTP_TurnSwSta_enum) -> bus_creator/295
  outpmodule/288(VOUTP_AmbBrightnessSta5_enum) -> bus_creator/288
  outpmodule/290(VOUTP_HazardIND_flg) -> bus_creator/290
  bus_selector2/93 -> outpmodule/96(VAPM_SASSpeedTimeOut_flg)  "<VAPM_SASSpeedTimeOut_flg>"
  bus_selector2/76 -> outpmodule/79(VAPM_LFPulseCount_enum)  "<VAPM_LFPulseCount_enum>"
  bus_selector2/85 -> outpmodule/88(VAPM_ShifterHandleCmdTimeOut_flg)  "<VAPM_ShifterHandleCmdTimeOut_flg>"
  bus_selector3/180 -> outpmodule/358(VBCM_FoxPiSwitchSta_enum)  "<VBCM_FoxPiSwitchSta_enum>"
  bus_selector3/181 -> outpmodule/359(VBCM_FoxPiLampSta_enum)  "<VBCM_FoxPiLampSta_enum>"
  bus_selector3/178 -> outpmodule/356(VBCM_WinLROpenedSta_pct)  "<VBCM_WinLROpenedSta_pct>"
  bus_selector3/175 -> outpmodule/353(VBCM_CLWinLockDrStaMem_enum)  "<VBCM_CLWinLockDrStaMem_enum>"
  bus_selector3/171 -> outpmodule/349(VBCM_PasWdwReqAP_enum)  "<VBCM_PasWdwReqAP_enum>"
  bus_selector9/23 -> outpmodule/577(VPMM_LowSOCWarn_enum)  "<VPMM_LowSOCWarn_enum>"
  bus_selector3/169 -> outpmodule/347(VBCM_AutoWipHSpdENSta_flg)  "<VBCM_AutoWipHSpdENSta_flg>"
  bus_selector3/170 -> outpmodule/348(VBCM_DrvWdwReqAP_enum)  "<VBCM_DrvWdwReqAP_enum>"
  outpmodule/971(VOUTP_ADASLanecurveR_raw32) -> bus_creator/971
  bus_selector3/168 -> outpmodule/346(VBCM_HMIKey8FuncSta_enum)  "<VBCM_HMIKey8FuncSta_enum>"
  bus_selector3/167 -> outpmodule/345(VBCM_HMIKey7FuncSta_enum)  "<VBCM_HMIKey7FuncSta_enum>"
  bus_selector3/166 -> outpmodule/344(VBCM_HMIKey6FuncSta_enum)  "<VBCM_HMIKey6FuncSta_enum>"
  bus_selector3/165 -> outpmodule/343(VBCM_HMIKey5FuncSta_enum)  "<VBCM_HMIKey5FuncSta_enum>"
  bus_selector3/160 -> outpmodule/338(VBCM_AutoUnlockMem_enum)  "<VBCM_AutoUnlockMem_enum>"
  bus_selector3/158 -> outpmodule/336(VBCM_AutoLockMem_enum)  "<VBCM_AutoLockMem_enum>"
  bus_selector3/157 -> outpmodule/335(VBCM_AutoLockSta_flg)  "<VBCM_AutoLockSta_flg>"
  bus_selector3/159 -> outpmodule/337(VBCM_AutoUnlockSta_flg)  "<VBCM_AutoUnlockSta_flg>"
  bus_selector3/155 -> outpmodule/333(VBCM_LRightStaCmd_flg)  "<VBCM_LRightStaCmd_flg>"
  bus_selector16/86 -> outpmodule/975(VVMC_ACCCtrlAvail_flg)  "<VVMC_ACCCtrlAvail_flg>"
  bus_selector3/150 -> outpmodule/328(VBCM_SenstivityPosnCmd_enum)  "<VBCM_SenstivityPosnCmd_enum>"
  bus_selector3/153 -> outpmodule/331(VBCM_ACCLevelMem34_enum)  "<VBCM_ACCLevelMem34_enum>"
  bus_selector3/152 -> outpmodule/330(VBCM_ACCLevelMem12_enum)  "<VBCM_ACCLevelMem12_enum>"
  bus_selector3/149 -> outpmodule/327(VBCM_PTGOpenHeight57_enum)  "<VBCM_PTGOpenHeight57_enum>"
  bus_selector3/147 -> outpmodule/325(VBCM_PTGOpenHeight12_enum)  "<VBCM_PTGOpenHeight12_enum>"
  bus_selector16/12 -> outpmodule/901(VVMC_LimitPCT_pct)  "<VVMC_LimitPCT_pct>"
  bus_selector3/144 -> outpmodule/322(VBCM_PTGUserHeight4_cnt)  "<VBCM_PTGUserHeight4_cnt>"
  bus_selector3/139 -> outpmodule/317(VBCM_PTGOpenHeightSta_enum)  "<VBCM_PTGOpenHeightSta_enum>"
  bus_selector9/31 -> outpmodule/585(VPMM_TimerAllowSleep_flg)  "<VPMM_TimerAllowSleep_flg>"
  bus_selector3/137 -> outpmodule/315(VBCM_HoodRelCmd_flg)  "<VBCM_HoodRelCmd_flg>"
  bus_selector3/135 -> outpmodule/313(VBCM_RmLpModeENFunSta_flg)  "<VBCM_RmLpModeENFunSta_flg>"
  bus_selector3/134 -> outpmodule/312(VBCM_WalkOutLkENFunSta_flg)  "<VBCM_WalkOutLkENFunSta_flg>"
  bus_selector3/132 -> outpmodule/310(VBCM_FollowMeENMem_enum)  "<VBCM_FollowMeENMem_enum>"
  bus_selector3/133 -> outpmodule/311(VBCM_WalkInUnLkENFunSta_flg)  "<VBCM_WalkInUnLkENFunSta_flg>"
  bus_selector4/153 -> outpmodule/512(VDDM_CAN4BusErrorDTC_raw32)  "<VDDM_CAN4BusErrorDTC_raw32>"
  bus_selector4/149 -> outpmodule/508(VDDM_VCUTailgateSWSta_flg)  "<VDDM_VCUTailgateSWSta_flg>"
  bus_selector4/148 -> outpmodule/507(VDDM_VCUHoodSWSta_flg)  "<VDDM_VCUHoodSWSta_flg>"
  bus_selector4/146 -> outpmodule/505(VDDM_VCURRDoorSta_flg)  "<VDDM_VCURRDoorSta_flg>"
  bus_creator/1 -> BOUTP_outputs/1
  bus_selector16/93 -> outpmodule/982(VVMC_APSStaSys_enum)  "<VVMC_APSStaSys_enum>"
  bus_selector2/129 -> outpmodule/132(VAPM_EPBExtApplyAvailTimeOut_flg)  "<VAPM_EPBExtApplyAvailTimeOut_flg>"
  outpmodule/300(VOUTP_TurnSwTimeSetSta123_enum) -> bus_creator/300
  bus_selector2/95 -> outpmodule/98(VAPM_SASSpeedValidTimeOut_flg)  "<VAPM_SASSpeedValidTimeOut_flg>"
  bus_selector2/86 -> outpmodule/89(VAPM_DriIntend_enum)  "<VAPM_DriIntend_enum>"
  bus_selector2/65 -> outpmodule/68(VAPM_LRWhlRotDirTimeOut_flg)  "<VAPM_LRWhlRotDirTimeOut_flg>"
  bus_selector7/2 -> outpmodule/540(VDSC_DISCTargetSpd_kph)  "<VDSC_DISCTargetSpd_kph>"
  bus_selector6/16 -> outpmodule/536(VDKC_KeyNumSta_enum)  "<VDKC_KeyNumSta_enum>"
  bus_selector6/13 -> outpmodule/533(VDKC_UIDLowPowerSta_enum)  "<VDKC_UIDLowPowerSta_enum>"
  bus_selector6/11 -> outpmodule/531(VDKC_KeyAreaPTG_enum)  "<VDKC_KeyAreaPTG_enum>"
  bus_selector3/129 -> outpmodule/307(VBCM_WalkOutLkENMem_enum)  "<VBCM_WalkOutLkENMem_enum>"
  bus_selector6/6 -> outpmodule/526(VDKC_DkeyShowIVISta_enum)  "<VDKC_DkeyShowIVISta_enum>"
  BDKC_outputs/1 -> bus_selector6/1
  outpmodule/302(VOUTP_FDLHandleLampCmd_flg) -> bus_creator/302
  bus_selector6/10 -> outpmodule/530(VDKC_DKeyWelcomeSta_enum)  "<VDKC_DKeyWelcomeSta_enum>"
  bus_selector3/131 -> outpmodule/309(VBCM_LockSettingStaMem_enum)  "<VBCM_LockSettingStaMem_enum>"
  bus_selector6/9 -> outpmodule/529(VDKC_PCommandToBCM_enum)  "<VDKC_PCommandToBCM_enum>"
  bus_selector6/4 -> outpmodule/524(VDKC_KeyMissSta_flg)  "<VDKC_KeyMissSta_flg>"
  bus_selector6/1 -> outpmodule/521(VDKC_DKCTimeSN_cnt)  "<VDKC_DKCTimeSN_cnt>"
  BDHP_outputs/1 -> bus_selector5/1
  bus_selector5/5 -> outpmodule/519(VDHP_EAPS1NRM_pct)  "<VDHP_EAPS1NRM_pct>"
  bus_selector5/3 -> outpmodule/517(VDHP_EAPS2MIN_pct)  "<VDHP_EAPS2MIN_pct>"
  bus_selector5/2 -> outpmodule/516(VDHP_EAPS1MIN_pct)  "<VDHP_EAPS1MIN_pct>"
  bus_selector8/4 -> outpmodule/546(VNMM_CSB_flg)  "<VNMM_CSB_flg>"
  bus_selector8/1 -> outpmodule/543(VNMM_AllCANTxReq_flg)  "<VNMM_AllCANTxReq_flg>"
  outpmodule/678(VOUTP_sigCbnSolarLeft_W) -> bus_creator/678
  outpmodule/676(VOUTP_sigSetTempZon2St_C) -> bus_creator/676
  bus_selector3/148 -> outpmodule/326(VBCM_PTGOpenHeight34_enum)  "<VBCM_PTGOpenHeight34_enum>"
  outpmodule/672(VOUTP_sigAirIntenZon1St_enum) -> bus_creator/672
  outpmodule/671(VOUTP_CCUSyncLampSts_flg) -> bus_creator/671
  outpmodule/670(VOUTP_CCUACMaxLampSts_flg) -> bus_creator/670
  outpmodule/669(VOUTP_CCUAutoLampSts_flg) -> bus_creator/669
  outpmodule/667(VOUTP_CabinMode_enum) -> bus_creator/667
  outpmodule/666(VOUTP_EDriveMode_enum) -> bus_creator/666
  outpmodule/664(VOUTP_FDBlowerCmd_pct) -> bus_creator/664
  bus_selector3/141 -> outpmodule/319(VBCM_PTGUserHeight1_cnt)  "<VBCM_PTGUserHeight1_cnt>"
  outpmodule/658(VOUTP_FDEWP1Cmd_enum) -> bus_creator/658
  outpmodule/657(VOUTP_FDAGSCmd_enum) -> bus_creator/657
  outpmodule/1001(VOUTP_FDCVMCAngCtrlTqWtGn_pct) -> bus_creator/1001
  outpmodule/651(VOUTP_FDEXV2Cmd_step) -> bus_creator/651
  outpmodule/649(VOUTP_FDSOV3Cmd_flg) -> bus_creator/649
  bus_selector4/147 -> outpmodule/506(VDDM_SysAllowReadySta_flg)  "<VDDM_SysAllowReadySta_flg>"
  outpmodule/650(VOUTP_FDEXV1Cmd_step) -> bus_creator/650
  outpmodule/647(VOUTP_FDSOV1Cmd_flg) -> bus_creator/647
  outpmodule/643(VOUTP_ModelYear_cnt) -> bus_creator/643
  outpmodule/641(VOUTP_PmicBootPath_raw32) -> bus_creator/641
  outpmodule/640(VOUTP_ECUGen2_cnt) -> bus_creator/640
  outpmodule/639(VOUTP_ECUGen1_cnt) -> bus_creator/639
  outpmodule/636(VOUTP_WisrBootReason_raw32) -> bus_creator/636
  outpmodule/638(VOUTP_CurrentNmState_enum) -> bus_creator/638
  outpmodule/634(VOUTP_FdcSlpTime_sec) -> bus_creator/634
  bus_selector16/1 -> outpmodule/890(VVMC_FeatSetSpdFinal_raw32)  "<VVMC_FeatSetSpdFinal_raw32>"
  outpmodule/635(VOUTP_PmicBootReason_enum) -> bus_creator/635
  outpmodule/633(VOUTP_FdcSlpReqRisingEdge_flg) -> bus_creator/633
  outpmodule/626(VOUTP_SHA3_cnt) -> bus_creator/626
  outpmodule/683(VOUTP_ACSubMode_enum) -> bus_creator/683
  outpmodule/287(VOUTP_AmbBrightnessSta4_enum) -> bus_creator/287
  outpmodule/682(VOUTP_sigCbnAirT_C) -> bus_creator/682
  outpmodule/681(VOUTP_sigAmbAirT_C) -> bus_creator/681
  BV2L_outputs/1 -> bus_selector15/1
  bus_selector15/6 -> outpmodule/888(VV2L_HVPO120VGrpALDSt_enum)  "<VV2L_HVPO120VGrpALDSt_enum>"
  bus_selector15/5 -> outpmodule/887(VV2L_ReqOBCIntrV2LEna_enum)  "<VV2L_ReqOBCIntrV2LEna_enum>"
  outpmodule/654(VOUTP_FDTWVCmd_pct) -> bus_creator/654
  bus_selector15/3 -> outpmodule/885(VV2L_ReqV2LIVIDisChrg_enum)  "<VV2L_ReqV2LIVIDisChrg_enum>"
  bus_selector15/1 -> outpmodule/883(VV2L_ReqOBCV2LEna_enum)  "<VV2L_ReqOBCV2LEna_enum>"
  outpmodule/232(VOUTP_AmbLightBrightness1_enum) -> bus_creator/232
  bus_selector14/1 -> outpmodule/881(VTQR_FrTMTqReq_Nm)  "<VTQR_FrTMTqReq_Nm>"
  outpmodule/291(VOUTP_DimSwSta_flg) -> bus_creator/291
  bus_selector14/2 -> outpmodule/882(VTQR_RrTMTqReq_Nm)  "<VTQR_RrTMTqReq_Nm>"
  bus_selector13/52 -> outpmodule/878(VTQD_VehActSpd_kph)  "<VTQD_VehActSpd_kph>"
  bus_selector4/142 -> outpmodule/501(VDDM_VCUBrkSWSta_enum)  "<VDDM_VCUBrkSWSta_enum>"
  bus_selector3/118 -> outpmodule/296(VBCM_TurnSwTSetSta_enum)  "<VBCM_TurnSwTSetSta_enum>"
  bus_selector2/117 -> outpmodule/120(VAPM_MCPressureVTimeOut_flg)  "<VAPM_MCPressureVTimeOut_flg>"
  bus_selector10/38 -> outpmodule/640(VSYS_ECUGen2_cnt)  "<VSYS_ECUGen2_cnt>"
  bus_selector10/35 -> outpmodule/637(VSYS_AcoreRebootCmdACK_flg)  "<VSYS_AcoreRebootCmdACK_flg>"
  bus_selector10/34 -> outpmodule/636(VSYS_WisrBootReason_raw32)  "<VSYS_WisrBootReason_raw32>"
  bus_selector10/31 -> outpmodule/633(VSYS_FdcSlpReqRisingEdge_flg)  "<VSYS_FdcSlpReqRisingEdge_flg>"
  bus_selector10/32 -> outpmodule/634(VSYS_FdcSlpTime_sec)  "<VSYS_FdcSlpTime_sec>"
  bus_selector10/33 -> outpmodule/635(VSYS_PmicBootReason_enum)  "<VSYS_PmicBootReason_enum>"
  bus_selector10/29 -> outpmodule/631(VSYS_SHA8_cnt)  "<VSYS_SHA8_cnt>"
  bus_selector10/27 -> outpmodule/629(VSYS_SHA6_cnt)  "<VSYS_SHA6_cnt>"
  bus_selector10/28 -> outpmodule/630(VSYS_SHA7_cnt)  "<VSYS_SHA7_cnt>"
  bus_selector10/24 -> outpmodule/626(VSYS_SHA3_cnt)  "<VSYS_SHA3_cnt>"
  bus_selector10/26 -> outpmodule/628(VSYS_SHA5_cnt)  "<VSYS_SHA5_cnt>"
  outpmodule/986(VOUTP_LongAcc_Gps) -> bus_creator/986
  bus_selector10/19 -> outpmodule/621(VSYS_Change1_cnt)  "<VSYS_Change1_cnt>"
  bus_selector10/17 -> outpmodule/619(VSYS_Variation_cnt)  "<VSYS_Variation_cnt>"
  bus_selector10/16 -> outpmodule/618(VSYS_Country2_cnt)  "<VSYS_Country2_cnt>"
  bus_selector10/7 -> outpmodule/609(VSYS_ECU1_cnt)  "<VSYS_ECU1_cnt>"
  bus_selector10/3 -> outpmodule/605(VSYS_HWVer3_cnt)  "<VSYS_HWVer3_cnt>"
  outpmodule/253(VOUTP_MFRDNBrightReq_pct) -> bus_creator/253
  bus_selector10/1 -> outpmodule/603(VSYS_HWVer1_cnt)  "<VSYS_HWVer1_cnt>"
  bus_selector11/84 -> outpmodule/729(VTHC_EWPBUflag3_flg)  "<VTHC_EWPBUflag3_flg>"
  bus_selector10/43 -> outpmodule/645(VSYS_Var5_cnt)  "<VSYS_Var5_cnt>"
  outpmodule/656(VOUTP_CoolgFanActDuty_pct) -> bus_creator/656
  bus_selector12/22 -> outpmodule/751(VTPM_TPMSCaliButtAllow_flg)  "<VTPM_TPMSCaliButtAllow_flg>"
  bus_selector12/20 -> outpmodule/749(VTPM_RRWheelDebug_flg)  "<VTPM_RRWheelDebug_flg>"
  bus_selector12/21 -> outpmodule/750(VTPM_TPMSResButtAllow_flg)  "<VTPM_TPMSResButtAllow_flg>"
  bus_selector12/65 -> outpmodule/794(VTPM_Chkfin_flg)  "<VTPM_Chkfin_flg>"
  bus_selector16/14 -> outpmodule/903(VVMC_RearWhlSlipRatioCtrl_flg)  "<VVMC_RearWhlSlipRatioCtrl_flg>"
  bus_selector12/13 -> outpmodule/742(VTPM_LFSensorFail_flg)  "<VTPM_LFSensorFail_flg>"
  bus_selector12/8 -> outpmodule/737(VTPM_RRWheelPress_raw8)  "<VTPM_RRWheelPress_raw8>"
  bus_selector12/10 -> outpmodule/739(VTPM_RFWheelTemp_C)  "<VTPM_RFWheelTemp_C>"
  bus_selector13/47 -> outpmodule/873(VTQD_SaveRegenMode_enum)  "<VTQD_SaveRegenMode_enum>"
  bus_selector3/172 -> outpmodule/350(VBCM_DrRWdwReqAP_enum)  "<VBCM_DrRWdwReqAP_enum>"
  bus_selector12/6 -> outpmodule/735(VTPM_RFWheelPress_raw8)  "<VTPM_RFWheelPress_raw8>"
  bus_selector12/4 -> outpmodule/733(VTPM_RRBatWarn_flg)  "<VTPM_RRBatWarn_flg>"
  bus_selector3/151 -> outpmodule/329(VBCM_TimeGapLevelSta_enum)  "<VBCM_TimeGapLevelSta_enum>"
  bus_selector12/2 -> outpmodule/731(VTPM_RFBatWarn_flg)  "<VTPM_RFBatWarn_flg>"
  bus_selector12/9 -> outpmodule/738(VTPM_LFWheelTemp_C)  "<VTPM_LFWheelTemp_C>"
  bus_selector12/61 -> outpmodule/790(VTPM_ID1messageALTU_raw8)  "<VTPM_ID1messageALTU_raw8>"
  bus_selector12/58 -> outpmodule/787(VTPM_S2WheelDebugALTU_pct)  "<VTPM_S2WheelDebugALTU_pct>"
  outpmodule/655(VOUTP_FDFrWPTCHeatPwrCmd_W) -> bus_creator/655
  bus_selector12/59 -> outpmodule/788(VTPM_S3WheelDebugALTU_pct)  "<VTPM_S3WheelDebugALTU_pct>"
  bus_selector12/55 -> outpmodule/784(VTPM_FAT_flg)  "<VTPM_FAT_flg>"
  bus_selector12/54 -> outpmodule/783(VTPM_RRP20_raw8)  "<VTPM_RRP20_raw8>"
  bus_selector12/56 -> outpmodule/785(VTPM_IDin_raw32)  "<VTPM_IDin_raw32>"
  bus_selector12/52 -> outpmodule/781(VTPM_RFP20_raw8)  "<VTPM_RFP20_raw8>"
  bus_selector12/53 -> outpmodule/782(VTPM_LRP20_raw8)  "<VTPM_LRP20_raw8>"
  bus_selector12/51 -> outpmodule/780(VTPM_LFP20_raw8)  "<VTPM_LFP20_raw8>"
  bus_selector12/16 -> outpmodule/745(VTPM_RRSensorFail_flg)  "<VTPM_RRSensorFail_flg>"
  bus_selector12/48 -> outpmodule/777(VTPM_S3L_enum)  "<VTPM_S3L_enum>"
  bus_selector12/47 -> outpmodule/776(VTPM_S2L_enum)  "<VTPM_S2L_enum>"
  bus_selector12/44 -> outpmodule/773(VTPM_S3ID_raw32)  "<VTPM_S3ID_raw32>"
  bus_selector12/41 -> outpmodule/770(VTPM_RRSensorMode_flg)  "<VTPM_RRSensorMode_flg>"
  bus_selector12/39 -> outpmodule/768(VTPM_RFSensorMode_flg)  "<VTPM_RFSensorMode_flg>"
  bus_selector12/35 -> outpmodule/764(VTPM_RRWheelPSW_raw8)  "<VTPM_RRWheelPSW_raw8>"
  bus_selector12/32 -> outpmodule/761(VTPM_LFWheelPSW_raw8)  "<VTPM_LFWheelPSW_raw8>"
  bus_selector12/30 -> outpmodule/759(VTPM_LRWheelTmpIndi_flg)  "<VTPM_LRWheelTmpIndi_flg>"
  bus_selector12/27 -> outpmodule/756(VTPM_TPMSWarnIndi_enum)  "<VTPM_TPMSWarnIndi_enum>"
  outpmodule/303(VOUTP_FDRHandleLampCmd_flg) -> bus_creator/303
  bus_selector12/26 -> outpmodule/755(VTPM_RRPressIndi_enum)  "<VTPM_RRPressIndi_enum>"
  bus_selector12/24 -> outpmodule/753(VTPM_RFPressIndi_enum)  "<VTPM_RFPressIndi_enum>"
  bus_selector13/1 -> outpmodule/827(VTQD_ParkRequest_flg)  "<VTQD_ParkRequest_flg>"
  bus_selector10/40 -> outpmodule/642(VSYS_DrivingMode_cnt)  "<VSYS_DrivingMode_cnt>"
  BTPM_outputs/1 -> bus_selector12/1
  bus_selector12/97 -> outpmodule/826(VTPM_ModelVersionChksum_raw)  "<VTPM_ModelVersionChksum_raw>"
  bus_selector12/94 -> outpmodule/823(VTPM_LProgress_enum)  "<VTPM_LProgress_enum>"
  bus_selector10/4 -> outpmodule/606(VSYS_CarModel1_cnt)  "<VSYS_CarModel1_cnt>"
  bus_selector12/95 -> outpmodule/824(VTPM_TPMSSensorIDRegStart_flg)  "<VTPM_TPMSSensorIDRegStart_flg>"
  bus_selector12/92 -> outpmodule/821(VTPM_WritingCnt_enum)  "<VTPM_WritingCnt_enum>"
  bus_selector12/89 -> outpmodule/818(VTPM_FlashS3ID_raw)  "<VTPM_FlashS3ID_raw>"
  bus_selector16/44 -> outpmodule/933(VVMC_ACCComfortBandLower_mps2)  "<VVMC_ACCComfortBandLower_mps2>"
  bus_selector12/88 -> outpmodule/817(VTPM_FlashS2ID_raw)  "<VTPM_FlashS2ID_raw>"
  bus_selector12/87 -> outpmodule/816(VTPM_FlashS1ID_raw)  "<VTPM_FlashS1ID_raw>"
  bus_selector12/82 -> outpmodule/811(VTPM_Flashchkdatavalid_enum)  "<VTPM_Flashchkdatavalid_enum>"
  bus_selector12/83 -> outpmodule/812(VTPM_Flashdatavalid_enum)  "<VTPM_Flashdatavalid_enum>"
  bus_selector12/81 -> outpmodule/810(VTPM_WriteChkfinRRID_raw)  "<VTPM_WriteChkfinRRID_raw>"
  bus_selector12/74 -> outpmodule/803(VTPM_WriteChkLFID_raw)  "<VTPM_WriteChkLFID_raw>"
  bus_selector12/76 -> outpmodule/805(VTPM_WriteChkLRID_raw)  "<VTPM_WriteChkLRID_raw>"
  bus_selector12/73 -> outpmodule/802(VTPM_RRPindi_enum)  "<VTPM_RRPindi_enum>"
  bus_selector13/46 -> outpmodule/872(VTQD_OPDHoldLamp_flg)  "<VTQD_OPDHoldLamp_flg>"
  bus_selector12/69 -> outpmodule/798(VTPM_TPMSResButt_flg)  "<VTPM_TPMSResButt_flg>"
  bus_selector12/14 -> outpmodule/743(VTPM_RFSensorFail_flg)  "<VTPM_RFSensorFail_flg>"
  outpmodule/248(VOUTP_IVIRST_flg) -> bus_creator/248
  bus_selector13/30 -> outpmodule/856(VTQD_FrIdcMin_A)  "<VTQD_FrIdcMin_A>"
  bus_selector13/31 -> outpmodule/857(VTQD_FrIdcMax_A)  "<VTQD_FrIdcMax_A>"
  bus_selector13/29 -> outpmodule/855(VTQD_ExternalTqAllow_flg)  "<VTQD_ExternalTqAllow_flg>"
  bus_selector13/27 -> outpmodule/853(VTQD_FrRgnPermSta_flg)  "<VTQD_FrRgnPermSta_flg>"
  bus_selector13/24 -> outpmodule/850(VTQD_RrEDUAvailBrkRgnTqV_flg)  "<VTQD_RrEDUAvailBrkRgnTqV_flg>"
  bus_selector13/22 -> outpmodule/848(VTQD_FrEDUAvailBrkRgnTqV_flg)  "<VTQD_FrEDUAvailBrkRgnTqV_flg>"
  bus_selector10/42 -> outpmodule/644(VSYS_Var4_cnt)  "<VSYS_Var4_cnt>"
  bus_selector13/19 -> outpmodule/845(VTQD_FrEDUSpd_rpm)  "<VTQD_FrEDUSpd_rpm>"
  bus_selector13/18 -> outpmodule/844(VTQD_RrEDURolRgnTq_Nm)  "<VTQD_RrEDURolRgnTq_Nm>"
  bus_selector13/14 -> outpmodule/840(VTQD_DriverWhlTqDemRr_Nm)  "<VTQD_DriverWhlTqDemRr_Nm>"
  bus_selector3/138 -> outpmodule/316(VBCM_WelcomeLight_enum)  "<VBCM_WelcomeLight_enum>"
  bus_selector13/12 -> outpmodule/838(VTQD_RrRgnDecrSta_flg)  "<VTQD_RrRgnDecrSta_flg>"
  bus_selector13/13 -> outpmodule/839(VTQD_DriverWhlTqDemFr_Nm)  "<VTQD_DriverWhlTqDemFr_Nm>"
  bus_selector13/10 -> outpmodule/836(VTQD_RrActvDmpDisabReq_flg)  "<VTQD_RrActvDmpDisabReq_flg>"
  bus_selector13/11 -> outpmodule/837(VTQD_FrRgnDecrSta_flg)  "<VTQD_FrRgnDecrSta_flg>"
  bus_selector13/8 -> outpmodule/834(VTQD_PButtonSta_enum)  "<VTQD_PButtonSta_enum>"
  bus_selector13/9 -> outpmodule/835(VTQD_FrActvDmpDisabReq_flg)  "<VTQD_FrActvDmpDisabReq_flg>"
  bus_selector4/40 -> outpmodule/399(VDDM_DrStSWDTC_raw32)  "<VDDM_DrStSWDTC_raw32>"
  bus_selector4/39 -> outpmodule/398(VDDM_LVSupHiDTC_raw32)  "<VDDM_LVSupHiDTC_raw32>"
  outpmodule/628(VOUTP_SHA5_cnt) -> bus_creator/628
  bus_selector4/38 -> outpmodule/397(VDDM_LVSupLoDTC_raw32)  "<VDDM_LVSupLoDTC_raw32>"
  bus_selector4/37 -> outpmodule/396(VDDM_IniLVLoDTC_raw32)  "<VDDM_IniLVLoDTC_raw32>"
  bus_selector4/62 -> outpmodule/421(VDDM_DiagRLTSDTC_raw32)  "<VDDM_DiagRLTSDTC_raw32>"
  bus_selector4/35 -> outpmodule/394(VDDM_MCUActDTC_raw32)  "<VDDM_MCUActDTC_raw32>"
  bus_selector4/30 -> outpmodule/389(VDDM_HiLvSaChkDTC_raw32)  "<VDDM_HiLvSaChkDTC_raw32>"
  bus_selector4/32 -> outpmodule/391(VDDM_MCUDisDTC_raw32)  "<VDDM_MCUDisDTC_raw32>"
  bus_selector16/88 -> outpmodule/977(VVMC_TimeGapCalcu_s)  "<VVMC_TimeGapCalcu_s>"
  bus_selector4/29 -> outpmodule/388(VDDM_DCDCEnaDTC_raw32)  "<VDDM_DCDCEnaDTC_raw32>"
  bus_selector4/24 -> outpmodule/383(VDDM_HVB4PreDTC_raw32)  "<VDDM_HVB4PreDTC_raw32>"
  bus_selector4/21 -> outpmodule/380(VDDM_BrkSWNoBacDTC_raw32)  "<VDDM_BrkSWNoBacDTC_raw32>"
  bus_selector4/19 -> outpmodule/378(VDDM_Lv4ErrDTC_raw32)  "<VDDM_Lv4ErrDTC_raw32>"
  bus_selector4/60 -> outpmodule/419(VDDM_DiagFLTSDTC_raw32)  "<VDDM_DiagFLTSDTC_raw32>"
  bus_selector4/16 -> outpmodule/375(VDDM_Lv1ErrDTC_raw32)  "<VDDM_Lv1ErrDTC_raw32>"
  bus_selector4/13 -> outpmodule/372(VDDM_C1ABM1RCDTC_raw32)  "<VDDM_C1ABM1RCDTC_raw32>"
  bus_selector4/12 -> outpmodule/371(VDDM_C3CCU2LCDTC_raw32)  "<VDDM_C3CCU2LCDTC_raw32>"
  bus_selector4/8 -> outpmodule/367(VDDM_C3CCU1CSDTC_raw32)  "<VDDM_C3CCU1CSDTC_raw32>"
  bus_selector4/5 -> outpmodule/364(VDDM_C3BMS1CSDTC_raw32)  "<VDDM_C3BMS1CSDTC_raw32>"
  bus_selector4/6 -> outpmodule/365(VDDM_C3BMS1LCDTC_raw32)  "<VDDM_C3BMS1LCDTC_raw32>"
  bus_selector4/4 -> outpmodule/363(VDDM_C3BMS1RCDTC_raw32)  "<VDDM_C3BMS1RCDTC_raw32>"
  bus_selector10/15 -> outpmodule/617(VSYS_Country1_cnt)  "<VSYS_Country1_cnt>"
  bus_selector4/1 -> outpmodule/360(VDDM_C3BMS6RCDTC_raw32)  "<VDDM_C3BMS6RCDTC_raw32>"
  bus_selector4/57 -> outpmodule/416(VDDM_ESC5NoComDTC_raw32)  "<VDDM_ESC5NoComDTC_raw32>"
  bus_selector4/53 -> outpmodule/412(VDDM_MCUR1NoComDTC_raw32)  "<VDDM_MCUR1NoComDTC_raw32>"
  bus_selector4/54 -> outpmodule/413(VDDM_Shifter1NoComDTC_raw32)  "<VDDM_Shifter1NoComDTC_raw32>"
  bus_selector4/51 -> outpmodule/410(VDDM_APSCorrErrDTC_raw32)  "<VDDM_APSCorrErrDTC_raw32>"
  bus_selector4/52 -> outpmodule/411(VDDM_MCUF1NoComDTC_raw32)  "<VDDM_MCUF1NoComDTC_raw32>"
  bus_selector4/49 -> outpmodule/408(VDDM_APS1SigOoRDTC_raw32)  "<VDDM_APS1SigOoRDTC_raw32>"
  bus_selector4/44 -> outpmodule/403(VDDM_RRDoorSWDTC_raw32)  "<VDDM_RRDoorSWDTC_raw32>"
  bus_selector1/3 -> outpmodule/3(VACC_VehHVPwrAvail4THCM_W)  "<VACC_VehHVPwrAvail4THCM_W>"
  bus_selector3/104 -> outpmodule/282(VBCM_AmbColorSta5_enum)  "<VBCM_AmbColorSta5_enum>"
  bus_selector1/1 -> outpmodule/1(VACC_HVTHCMSysAvail_enum)  "<VACC_HVTHCMSysAvail_enum>"
  outpmodule/306(VOUTP_WalkInUnLkENMem_enum) -> bus_creator/306
  bus_selector2/92 -> outpmodule/95(VAPM_SASSpeed_degps)  "<VAPM_SASSpeed_degps>"
  outpmodule/912(VOUTP_ACCRequiredAccel_mps2) -> bus_creator/912
  outpmodule/911(VOUTP_ISOJerkLimit_mps3) -> bus_creator/911
  outpmodule/909(VOUTP_ISOAccLimit_mps2) -> bus_creator/909
  bus_selector3/146 -> outpmodule/324(VBCM_PTGUserHeight7_cnt)  "<VBCM_PTGUserHeight7_cnt>"
  outpmodule/908(VOUTP_AccCalcuPID_mps2) -> bus_creator/908
  outpmodule/910(VOUTP_ISODecLimit_mps2) -> bus_creator/910
  bus_selector10/23 -> outpmodule/625(VSYS_SHA2_cnt)  "<VSYS_SHA2_cnt>"
  bus_selector16/34 -> outpmodule/923(VVMC_AEBVehHoldReq_flg)  "<VVMC_AEBVehHoldReq_flg>"
  outpmodule/905(VOUTP_LatAccCtrl_flg) -> bus_creator/905
  outpmodule/904(VOUTP_SingleWhlSlipRatioCtrl_flg) -> bus_creator/904
  outpmodule/961(VOUTP_LVDADisabled_flg) -> bus_creator/961
  outpmodule/900(VOUTP_JerkPCT_pct) -> bus_creator/900
  outpmodule/901(VOUTP_LimitPCT_pct) -> bus_creator/901
  outpmodule/902(VOUTP_FrontRearSlipRatioCtrl_flg) -> bus_creator/902
  outpmodule/899(VOUTP_FeatReqSpd_kph) -> bus_creator/899
  outpmodule/898(VOUTP_FeatArbitrSta_enum) -> bus_creator/898
  bus_selector13/20 -> outpmodule/846(VTQD_RrEDUSpd_rpm)  "<VTQD_RrEDUSpd_rpm>"
  outpmodule/897(VOUTP_VMCMSACtrlAvail_flg) -> bus_creator/897
  outpmodule/894(VOUTP_VMCAEBCtrlAvail_flg) -> bus_creator/894
  outpmodule/890(VOUTP_FeatSetSpdFinal_raw32) -> bus_creator/890
  outpmodule/957(VOUTP_ADASISASta_enum) -> bus_creator/957
  outpmodule/955(VOUTP_ADASLaneModeR_enum) -> bus_creator/955
  outpmodule/949(VOUTP_TargetType_enum) -> bus_creator/949
  bus_selector4/58 -> outpmodule/417(VDDM_EnterNewOperCyc_flg)  "<VDDM_EnterNewOperCyc_flg>"
  outpmodule/950(VOUTP_ADASSLIFSpdLim_enum) -> bus_creator/950
  outpmodule/948(VOUTP_ADASCAMSpdLim_enum) -> bus_creator/948
  bus_selector2/132 -> outpmodule/135(VAPM_EPBSta_enum)  "<VAPM_EPBSta_enum>"
  outpmodule/946(VOUTP_ACCTakeoverReq_flg) -> bus_creator/946
  outpmodule/942(VOUTP_ADASLDWSta_enum) -> bus_creator/942
  outpmodule/944(VOUTP_ACCObjDstLvl_enum) -> bus_creator/944
  bus_selector4/59 -> outpmodule/418(VDDM_DiagHCrashDTC_raw32)  "<VDDM_DiagHCrashDTC_raw32>"
  outpmodule/940(VOUTP_LeftTurnLightReq_flg) -> bus_creator/940
  bus_selector9/24 -> outpmodule/578(VPMM_ReVehThdChkSta_enum)  "<VPMM_ReVehThdChkSta_enum>"
  outpmodule/941(VOUTP_ADASFCWSta_enum) -> bus_creator/941
  bus_selector13/28 -> outpmodule/854(VTQD_RrRgnPermSta_flg)  "<VTQD_RrRgnPermSta_flg>"
  outpmodule/938(VOUTP_HazardWarningReq_flg) -> bus_creator/938
  outpmodule/937(VOUTP_ADASForceIdle_flg) -> bus_creator/937
  outpmodule/933(VOUTP_ACCComfortBandLower_mps2) -> bus_creator/933
  outpmodule/931(VOUTP_ACCComfortBandUpper_mps2) -> bus_creator/931
  bus_selector12/5 -> outpmodule/734(VTPM_LFWheelPress_raw8)  "<VTPM_LFWheelPress_raw8>"
  outpmodule/928(VOUTP_ACCObjRelSpd_mps) -> bus_creator/928
  outpmodule/930(VOUTP_ACCJerkUpperLimit_mps3) -> bus_creator/930
  outpmodule/929(VOUTP_TimeGapLevel_enum) -> bus_creator/929
  outpmodule/926(VOUTP_ADASACCSta_enum) -> bus_creator/926
  outpmodule/927(VOUTP_ACCObjDist_m) -> bus_creator/927
  bus_selector5/1 -> outpmodule/515(VDHP_ActAPSPosn_pct)  "<VDHP_ActAPSPosn_pct>"
  outpmodule/925(VOUTP_ADASDBSReq_enum) -> bus_creator/925
  outpmodule/924(VOUTP_ACCVehHoldReq_flg) -> bus_creator/924
  outpmodule/923(VOUTP_AEBVehHoldReq_flg) -> bus_creator/923
  bus_selector8/9 -> outpmodule/551(VNMM_WakeUp_enum)  "<VNMM_WakeUp_enum>"
  outpmodule/922(VOUTP_ADASFaultSta_flg) -> bus_creator/922
  bus_selector12/66 -> outpmodule/795(VTPM_SetIDLoc_flg)  "<VTPM_SetIDLoc_flg>"
  bus_selector16/13 -> outpmodule/902(VVMC_FrontRearSlipRatioCtrl_flg)  "<VVMC_FrontRearSlipRatioCtrl_flg>"
  outpmodule/918(VOUTP_LKAStrToqReq_Nm) -> bus_creator/918
  outpmodule/916(VOUTP_LateralCtrl_flg) -> bus_creator/916
  outpmodule/915(VOUTP_ActACCRequiredAccel_mps2) -> bus_creator/915
  outpmodule/913(VOUTP_DISCReqAcc_mps2) -> bus_creator/913
  outpmodule/844(VOUTP_RrEDURolRgnTq_Nm) -> bus_creator/844
  outpmodule/843(VOUTP_FrEDURolRgnTq_Nm) -> bus_creator/843
  outpmodule/840(VOUTP_DriverWhlTqDemRr_Nm) -> bus_creator/840
  outpmodule/629(VOUTP_SHA6_cnt) -> bus_creator/629
  outpmodule/839(VOUTP_DriverWhlTqDemFr_Nm) -> bus_creator/839
  outpmodule/838(VOUTP_RrRgnDecrSta_flg) -> bus_creator/838
  outpmodule/837(VOUTP_FrRgnDecrSta_flg) -> bus_creator/837
  outpmodule/835(VOUTP_FrActvDmpDisabReq_flg) -> bus_creator/835
  outpmodule/834(VOUTP_PButtonSta_enum) -> bus_creator/834
  outpmodule/668(VOUTP_CCUACLampSts_flg) -> bus_creator/668
  outpmodule/829(VOUTP_TqSourceRr_enum) -> bus_creator/829
  outpmodule/825(VOUTP_ModelVersion_raw) -> bus_creator/825
  bus_selector4/42 -> outpmodule/401(VDDM_RLDoorSWDTC_raw32)  "<VDDM_RLDoorSWDTC_raw32>"
  outpmodule/827(VOUTP_ParkRequest_flg) -> bus_creator/827
  outpmodule/824(VOUTP_TPMSSensorIDRegStart_flg) -> bus_creator/824
  bus_selector13/5 -> outpmodule/831(VTQD_RrEDUAvailBrkRgnTq_Nm)  "<VTQD_RrEDUAvailBrkRgnTq_Nm>"
  outpmodule/823(VOUTP_LProgress_enum) -> bus_creator/823
  outpmodule/652(VOUTP_FDSOTXVCmd_flg) -> bus_creator/652
  outpmodule/816(VOUTP_FlashS1ID_raw) -> bus_creator/816
  outpmodule/815(VOUTP_Prepresstempvalid_enum) -> bus_creator/815
  outpmodule/814(VOUTP_unlearnSfailvalid_enum) -> bus_creator/814
  bus_selector12/34 -> outpmodule/763(VTPM_RFWheelPSW_raw8)  "<VTPM_RFWheelPSW_raw8>"
  outpmodule/812(VOUTP_Flashdatavalid_enum) -> bus_creator/812
  outpmodule/881(VOUTP_FrTMTqReq_Nm) -> bus_creator/881
  outpmodule/880(VOUTP_SetSpdLimWarn_flg) -> bus_creator/880
  bus_selector12/67 -> outpmodule/796(VTPM_TPMSStorge_flg)  "<VTPM_TPMSStorge_flg>"
  outpmodule/879(VOUTP_RegenLimIndSta_flg) -> bus_creator/879
  outpmodule/878(VOUTP_VehActSpd_kph) -> bus_creator/878
  outpmodule/886(VOUTP_ReqOBCExtrV2LEna_enum) -> bus_creator/886
  outpmodule/644(VOUTP_Var4_cnt) -> bus_creator/644
  outpmodule/876(VOUTP_SpdCtrlSta_flg) -> bus_creator/876
  outpmodule/875(VOUTP_SpdCtrlMode_enum) -> bus_creator/875
  outpmodule/874(VOUTP_FDCVCURegenMode_enum) -> bus_creator/874
  bus_selector16/54 -> outpmodule/943(VVMC_ADASFltWrnReq_flg)  "<VVMC_ADASFltWrnReq_flg>"
  outpmodule/872(VOUTP_OPDHoldLamp_flg) -> bus_creator/872
  outpmodule/645(VOUTP_Var5_cnt) -> bus_creator/645
  outpmodule/870(VOUTP_IVIPwrLockSta_enum) -> bus_creator/870
  outpmodule/869(VOUTP_ActParkRequest_flg) -> bus_creator/869
  outpmodule/867(VOUTP_EquivAccPedalSWSta_flg) -> bus_creator/867
  outpmodule/866(VOUTP_CreepON_flg) -> bus_creator/866
  bus_selector13/54 -> outpmodule/880(VTQD_SetSpdLimWarn_flg)  "<VTQD_SetSpdLimWarn_flg>"
  outpmodule/864(VOUTP_ReBrakeLPReq_flg) -> bus_creator/864
  outpmodule/885(VOUTP_ReqV2LIVIDisChrg_enum) -> bus_creator/885
  BNMM_outputs/1 -> bus_selector8/1
  outpmodule/862(VOUTP_RrUdcMin_V) -> bus_creator/862
  outpmodule/856(VOUTP_FrIdcMin_A) -> bus_creator/856
  outpmodule/855(VOUTP_ExternalTqAllow_flg) -> bus_creator/855
  outpmodule/854(VOUTP_RrRgnPermSta_flg) -> bus_creator/854
  bus_selector9/25 -> outpmodule/579(VPMM_EvccAplusPwrUpReq_flg)  "<VPMM_EvccAplusPwrUpReq_flg>"
  outpmodule/850(VOUTP_RrEDUAvailBrkRgnTqV_flg) -> bus_creator/850
  bus_selector12/42 -> outpmodule/771(VTPM_S1ID_raw32)  "<VTPM_S1ID_raw32>"
  outpmodule/849(VOUTP_RrEDUSpdValid_flg) -> bus_creator/849
  bus_selector16/61 -> outpmodule/950(VVMC_ADASSLIFSpdLim_enum)  "<VVMC_ADASSLIFSpdLim_enum>"
  outpmodule/884(VOUTP_ReqV2LIVIPopup_enum) -> bus_creator/884
  bus_selector8/3 -> outpmodule/545(VNMM_Awake_enum)  "<VNMM_Awake_enum>"
  outpmodule/845(VOUTP_FrEDUSpd_rpm) -> bus_creator/845
  bus_selector3/86 -> outpmodule/264(VBCM_AmbPwrWarnEN_flg)  "<VBCM_AmbPwrWarnEN_flg>"
  bus_selector3/83 -> outpmodule/261(VBCM_AmbWelEN_flg)  "<VBCM_AmbWelEN_flg>"
  bus_selector12/78 -> outpmodule/807(VTPM_WriteChkfinLFID_raw)  "<VTPM_WriteChkfinLFID_raw>"
  bus_selector3/108 -> outpmodule/286(VBCM_AmbBrightnessSta3_enum)  "<VBCM_AmbBrightnessSta3_enum>"
  bus_selector3/78 -> outpmodule/256(VBCM_PasWdwCtrlCmd_pct)  "<VBCM_PasWdwCtrlCmd_pct>"
  bus_selector3/79 -> outpmodule/257(VBCM_DrRWdwCtrlCmd_pct)  "<VBCM_DrRWdwCtrlCmd_pct>"
  outpmodule/945(VOUTP_ForceLowBeam_enum) -> bus_creator/945
  bus_selector3/77 -> outpmodule/255(VBCM_DrvWdwCtrlCmd_pct)  "<VBCM_DrvWdwCtrlCmd_pct>"
  bus_selector3/76 -> outpmodule/254(VBCM_PTGInnerSW2_enum)  "<VBCM_PTGInnerSW2_enum>"
  outpmodule/920(VOUTP_LKATOIAct_enum) -> bus_creator/920
  bus_selector13/6 -> outpmodule/832(VTQD_EVDriveMode_enum)  "<VTQD_EVDriveMode_enum>"
  bus_selector10/13 -> outpmodule/615(VSYS_Patch1_cnt)  "<VSYS_Patch1_cnt>"
  bus_selector3/102 -> outpmodule/280(VBCM_AmbColorSta3_enum)  "<VBCM_AmbColorSta3_enum>"
  bus_selector3/75 -> outpmodule/253(VBCM_MFRDNBrightReq_pct)  "<VBCM_MFRDNBrightReq_pct>"
  bus_selector3/74 -> outpmodule/252(VBCM_FuelDoorPos_flg)  "<VBCM_FuelDoorPos_flg>"
  bus_selector3/69 -> outpmodule/247(VBCM_FollowMe_flg)  "<VBCM_FollowMe_flg>"
  outpmodule/828(VOUTP_TqSourceFr_enum) -> bus_creator/828
  bus_selector12/17 -> outpmodule/746(VTPM_LFWheelDebug_flg)  "<VTPM_LFWheelDebug_flg>"
  bus_selector3/101 -> outpmodule/279(VBCM_AmbColorSta2_enum)  "<VBCM_AmbColorSta2_enum>"
  outpmodule/817(VOUTP_FlashS2ID_raw) -> bus_creator/817
  bus_selector3/106 -> outpmodule/284(VBCM_AmbBrightnessSta1_enum)  "<VBCM_AmbBrightnessSta1_enum>"
  bus_selector3/60 -> outpmodule/238(VBCM_AmbLightColor1_enum)  "<VBCM_AmbLightColor1_enum>"
  bus_selector3/58 -> outpmodule/236(VBCM_AmbLightBrightness5_enum)  "<VBCM_AmbLightBrightness5_enum>"
  bus_selector3/57 -> outpmodule/235(VBCM_AmbLightBrightness4_enum)  "<VBCM_AmbLightBrightness4_enum>"
  bus_selector3/84 -> outpmodule/262(VBCM_AmbDimEN_flg)  "<VBCM_AmbDimEN_flg>"
  bus_selector3/55 -> outpmodule/233(VBCM_AmbLightBrightness2_enum)  "<VBCM_AmbLightBrightness2_enum>"
  bus_selector3/100 -> outpmodule/278(VBCM_AmbColorSta1_enum)  "<VBCM_AmbColorSta1_enum>"
  bus_selector3/54 -> outpmodule/232(VBCM_AmbLightBrightness1_enum)  "<VBCM_AmbLightBrightness1_enum>"
  bus_selector12/91 -> outpmodule/820(VTPM_FlashIDvalid_enum)  "<VTPM_FlashIDvalid_enum>"
  bus_selector3/51 -> outpmodule/229(VBCM_AmbLightBreath4_enum)  "<VBCM_AmbLightBreath4_enum>"
  bus_selector3/52 -> outpmodule/230(VBCM_AmbLightBreath5_enum)  "<VBCM_AmbLightBreath5_enum>"
  bus_selector3/49 -> outpmodule/227(VBCM_AmbLightBreath2_enum)  "<VBCM_AmbLightBreath2_enum>"
  bus_selector3/47 -> outpmodule/225(VBCM_WiperFixMode_flg)  "<VBCM_WiperFixMode_flg>"
  bus_selector3/43 -> outpmodule/221(VBCM_FrWiperL_flg)  "<VBCM_FrWiperL_flg>"
  bus_selector10/25 -> outpmodule/627(VSYS_SHA4_cnt)  "<VSYS_SHA4_cnt>"
  bus_selector3/40 -> outpmodule/218(VBCM_RoomLampL_flg)  "<VBCM_RoomLampL_flg>"
  bus_selector3/99 -> outpmodule/277(VBCM_AmbODAENFlash_enum)  "<VBCM_AmbODAENFlash_enum>"
  bus_selector3/34 -> outpmodule/212(VBCM_RTurnLP_flg)  "<VBCM_RTurnLP_flg>"
  bus_selector3/35 -> outpmodule/213(VBCM_BCMBuzzerReq_flg)  "<VBCM_BCMBuzzerReq_flg>"
  outpmodule/653(VOUTP_FDFWVCmd_flg) -> bus_creator/653
  bus_selector3/36 -> outpmodule/214(VBCM_MirrorCtrl_enum)  "<VBCM_MirrorCtrl_enum>"
  bus_selector3/33 -> outpmodule/211(VBCM_LTurnLP_flg)  "<VBCM_LTurnLP_flg>"
  bus_selector3/98 -> outpmodule/276(VBCM_AmbPwrWarnENFlash_enum)  "<VBCM_AmbPwrWarnENFlash_enum>"
  outpmodule/822(VOUTP_TPMSTLCmd_flg) -> bus_creator/822
  bus_selector3/32 -> outpmodule/210(VBCM_HazardSW_flg)  "<VBCM_HazardSW_flg>"
  bus_selector3/30 -> outpmodule/208(VBCM_LBSD_flg)  "<VBCM_LBSD_flg>"
  bus_selector12/23 -> outpmodule/752(VTPM_LFPressIndi_enum)  "<VTPM_LFPressIndi_enum>"
  bus_selector3/31 -> outpmodule/209(VBCM_RBSD_flg)  "<VBCM_RBSD_flg>"
  outpmodule/250(VOUTP_MFSWTri_flg) -> bus_creator/250
  bus_selector3/29 -> outpmodule/207(VBCM_RDRL_flg)  "<VBCM_RDRL_flg>"
  bus_selector3/28 -> outpmodule/206(VBCM_LDRL_flg)  "<VBCM_LDRL_flg>"
  BDSC_outputs/1 -> bus_selector7/1
  bus_selector3/97 -> outpmodule/275(VBCM_AmbLinkDriStaFlash_enum)  "<VBCM_AmbLinkDriStaFlash_enum>"
  bus_selector3/27 -> outpmodule/205(VBCM_ReverseLamp_flg)  "<VBCM_ReverseLamp_flg>"
  bus_selector9/38 -> outpmodule/592(VPMM_CtrlFrRC1_flg)  "<VPMM_CtrlFrRC1_flg>"
  bus_selector3/25 -> outpmodule/203(VBCM_RrFogLamp_flg)  "<VBCM_RrFogLamp_flg>"
  bus_selector3/22 -> outpmodule/200(VBCM_PosLamp_flg)  "<VBCM_PosLamp_flg>"
  bus_selector16/74 -> outpmodule/963(VVMC_LVDAFailinfo_flg)  "<VVMC_LVDAFailinfo_flg>"
  bus_selector3/23 -> outpmodule/201(VBCM_LBeam_flg)  "<VBCM_LBeam_flg>"
  bus_selector3/20 -> outpmodule/198(VBCM_Dimmer_pct)  "<VBCM_Dimmer_pct>"
  bus_selector3/96 -> outpmodule/274(VBCM_AmbDimENFlash_enum)  "<VBCM_AmbDimENFlash_enum>"
  outpmodule/883(VOUTP_ReqOBCV2LEna_enum) -> bus_creator/883
  bus_selector12/57 -> outpmodule/786(VTPM_S1WheelDebugALTU_pct)  "<VTPM_S1WheelDebugALTU_pct>"
  bus_selector3/18 -> outpmodule/196(VBCM_DoorLockIND_flg)  "<VBCM_DoorLockIND_flg>"
  bus_selector3/13 -> outpmodule/191(VBCM_LockSetting_flg)  "<VBCM_LockSetting_flg>"
  bus_selector3/14 -> outpmodule/192(VBCM_FrChargingDoorCtrl_enum)  "<VBCM_FrChargingDoorCtrl_enum>"
  outpmodule/268(VOUTP_LockAlarm_enum) -> bus_creator/268
  bus_selector3/11 -> outpmodule/189(VBCM_RLDoorSW_flg)  "<VBCM_RLDoorSW_flg>"
  bus_selector3/9 -> outpmodule/187(VBCM_DrDoorSW_flg)  "<VBCM_DrDoorSW_flg>"
  bus_selector3/10 -> outpmodule/188(VBCM_PsDoorSW_flg)  "<VBCM_PsDoorSW_flg>"
  bus_selector3/109 -> outpmodule/287(VBCM_AmbBrightnessSta4_enum)  "<VBCM_AmbBrightnessSta4_enum>"
  bus_selector3/8 -> outpmodule/186(VBCM_TailgateSW_flg)  "<VBCM_TailgateSW_flg>"
  bus_selector10/10 -> outpmodule/612(VSYS_Major2_cnt)  "<VSYS_Major2_cnt>"
  bus_selector16/24 -> outpmodule/913(VVMC_DISCReqAcc_mps2)  "<VVMC_DISCReqAcc_mps2>"
  bus_selector3/3 -> outpmodule/181(VBCM_HornCtrl_flg)  "<VBCM_HornCtrl_flg>"
  outpmodule/280(VOUTP_AmbColorSta3_enum) -> bus_creator/280
  bus_selector3/7 -> outpmodule/185(VBCM_HoodSW_flg)  "<VBCM_HoodSW_flg>"
  bus_selector3/4 -> outpmodule/182(VBCM_AllDoorSW_flg)  "<VBCM_AllDoorSW_flg>"
  bus_selector3/6 -> outpmodule/184(VBCM_AntitheftSeatFlod_flg)  "<VBCM_AntitheftSeatFlod_flg>"
  bus_selector3/5 -> outpmodule/183(VBCM_BCMDoorLockSta_flg)  "<VBCM_BCMDoorLockSta_flg>"
  bus_selector3/92 -> outpmodule/270(VBCM_fUnlockSingle_flg)  "<VBCM_fUnlockSingle_flg>"
  bus_selector3/72 -> outpmodule/250(VBCM_MFSWTri_flg)  "<VBCM_MFSWTri_flg>"
  bus_selector13/26 -> outpmodule/852(VTQD_PTCSPermSta_flg)  "<VTQD_PTCSPermSta_flg>"
  bus_selector10/14 -> outpmodule/616(VSYS_Patch2_cnt)  "<VSYS_Patch2_cnt>"
  bus_selector3/94 -> outpmodule/272(VBCM_AmbFunENFlash_enum)  "<VBCM_AmbFunENFlash_enum>"
  bus_selector3/62 -> outpmodule/240(VBCM_AmbLightColor3_enum)  "<VBCM_AmbLightColor3_enum>"
  bus_selector3/93 -> outpmodule/271(VBCM_UserNow_enum)  "<VBCM_UserNow_enum>"
  bus_selector3/91 -> outpmodule/269(VBCM_ATCtrl_enum)  "<VBCM_ATCtrl_enum>"
  bus_selector16/60 -> outpmodule/949(VVMC_TargetType_enum)  "<VVMC_TargetType_enum>"
  bus_selector3/90 -> outpmodule/268(VBCM_LockAlarm_enum)  "<VBCM_LockAlarm_enum>"
  bus_selector3/87 -> outpmodule/265(VBCM_AmbODAEN_flg)  "<VBCM_AmbODAEN_flg>"
  outpmodule/159(VOUTP_APSSWVer_enum) -> bus_creator/159
  bus_selector2/64 -> outpmodule/67(VAPM_LRWhlRotDir_enum)  "<VAPM_LRWhlRotDir_enum>"
  outpmodule/157(VOUTP_APSProgressPCT_pct) -> bus_creator/157
  outpmodule/158(VOUTP_APSRQDisplay_enum) -> bus_creator/158
  outpmodule/155(VOUTP_DriverSeatBeltCmd_flg) -> bus_creator/155
  outpmodule/858(VOUTP_FrUdcMin_V) -> bus_creator/858
  outpmodule/154(VOUTP_TCSActiveTimeOut_flg) -> bus_creator/154
  outpmodule/152(VOUTP_ABSActiveTimeOut_flg) -> bus_creator/152
  outpmodule/161(VOUTP_APSExitCondition_enum) -> bus_creator/161
  outpmodule/162(VOUTP_APSAngleTarget_Deg) -> bus_creator/162
  bus_selector10/39 -> outpmodule/641(VSYS_PmicBootPath_raw32)  "<VSYS_PmicBootPath_raw32>"
  outpmodule/160(VOUTP_APSHWVer_enum) -> bus_creator/160
  bus_selector8/11 -> outpmodule/553(VNMM_SysNMmSta_enum)  "<VNMM_SysNMmSta_enum>"
  bus_selector4/111 -> outpmodule/470(VDDM_LFBatwarnDTC_raw32)  "<VDDM_LFBatwarnDTC_raw32>"
  bus_selector4/108 -> outpmodule/467(VDDM_ESC5CSErrDTC_raw32)  "<VDDM_ESC5CSErrDTC_raw32>"
  bus_selector4/107 -> outpmodule/466(VDDM_ESC5RCErrDTC_raw32)  "<VDDM_ESC5RCErrDTC_raw32>"
  bus_selector3/16 -> outpmodule/194(VBCM_CrashDetd_flg)  "<VBCM_CrashDetd_flg>"
  bus_selector4/104 -> outpmodule/463(VDDM_ESC7CSErrDTC_raw32)  "<VDDM_ESC7CSErrDTC_raw32>"
  bus_selector4/106 -> outpmodule/465(VDDM_ESC1CSErrDTC_raw32)  "<VDDM_ESC1CSErrDTC_raw32>"
  bus_selector4/105 -> outpmodule/464(VDDM_ESC1RCErrDTC_raw32)  "<VDDM_ESC1RCErrDTC_raw32>"
  outpmodule/661(VOUTP_FDFrLeAPTCHeatPwrCmd_W) -> bus_creator/661
  bus_selector4/101 -> outpmodule/460(VDDM_Shifter1RCErrDTC_raw32)  "<VDDM_Shifter1RCErrDTC_raw32>"
  bus_selector4/103 -> outpmodule/462(VDDM_ESC7RCErrDTC_raw32)  "<VDDM_ESC7RCErrDTC_raw32>"
  bus_selector4/102 -> outpmodule/461(VDDM_Shifter1CSErrDTC_raw32)  "<VDDM_Shifter1CSErrDTC_raw32>"
  bus_selector2/66 -> outpmodule/69(VAPM_RRWhlRotDir_enum)  "<VAPM_RRWhlRotDir_enum>"
  bus_selector4/100 -> outpmodule/459(VDDM_MCUR1CSErrDTC_raw32)  "<VDDM_MCUR1CSErrDTC_raw32>"
  outpmodule/935(VOUTP_ADASShftPosnReqA_flg) -> bus_creator/935
  bus_selector4/98 -> outpmodule/457(VDDM_MCUR1RCErrDTC_raw32)  "<VDDM_MCUR1RCErrDTC_raw32>"
  bus_selector4/99 -> outpmodule/458(VDDM_MCUF1CSErrDTC_raw32)  "<VDDM_MCUF1CSErrDTC_raw32>"
  bus_selector4/87 -> outpmodule/446(VDDM_BMSSigErrDetDTC_raw32)  "<VDDM_BMSSigErrDetDTC_raw32>"
  bus_selector4/88 -> outpmodule/447(VDDM_FCMACCSigErrDetDTC_raw32)  "<VDDM_FCMACCSigErrDetDTC_raw32>"
  bus_selector8/12 -> outpmodule/554(VNMM_NetworkReq_flg)  "<VNMM_NetworkReq_flg>"
  bus_selector4/84 -> outpmodule/443(VDDM_FCM5NoComDTC_raw32)  "<VDDM_FCM5NoComDTC_raw32>"
  bus_selector4/83 -> outpmodule/442(VDDM_FCM4CSErrDTC_raw32)  "<VDDM_FCM4CSErrDTC_raw32>"
  bus_selector4/77 -> outpmodule/436(VDDM_FCM2RCErrDTC_raw32)  "<VDDM_FCM2RCErrDTC_raw32>"
  outpmodule/939(VOUTP_RightTurnLightReq_flg) -> bus_creator/939
  bus_selector4/71 -> outpmodule/430(VDDM_RCRUSSDTC_raw32)  "<VDDM_RCRUSSDTC_raw32>"
  bus_selector9/15 -> outpmodule/569(VPMM_RrMCUEnaReq_flg)  "<VPMM_RrMCUEnaReq_flg>"
  bus_selector4/68 -> outpmodule/427(VDDM_RCLUSSDTC_raw32)  "<VDDM_RCLUSSDTC_raw32>"
  bus_selector4/65 -> outpmodule/424(VDDM_FMLUSSDTC_raw32)  "<VDDM_FMLUSSDTC_raw32>"
  bus_selector4/137 -> outpmodule/496(VDDM_VCURAPSErrLv3_flg)  "<VDDM_VCURAPSErrLv3_flg>"
  bus_selector4/138 -> outpmodule/497(VDDM_EDriveSysErrShifterErr_flg)  "<VDDM_EDriveSysErrShifterErr_flg>"
  bus_selector4/139 -> outpmodule/498(VDDM_LVSysErrPwrOutErr_flg)  "<VDDM_LVSysErrPwrOutErr_flg>"
  bus_selector4/136 -> outpmodule/495(VDDM_VCURAPSErrLv2_flg)  "<VDDM_VCURAPSErrLv2_flg>"
  bus_selector4/135 -> outpmodule/494(VDDM_DisengagePFail_flg)  "<VDDM_DisengagePFail_flg>"
  bus_selector4/133 -> outpmodule/492(VDDM_DTCDetect_enum)  "<VDDM_DTCDetect_enum>"
  bus_selector9/30 -> outpmodule/584(VPMM_SilentChkAllowSleep_flg)  "<VPMM_SilentChkAllowSleep_flg>"
  bus_selector4/130 -> outpmodule/489(VDDM_EPBLockTODTC_raw32)  "<VDDM_EPBLockTODTC_raw32>"
  bus_selector4/129 -> outpmodule/488(VDDM_5vAPS2PwrErrDTC_raw32)  "<VDDM_5vAPS2PwrErrDTC_raw32>"
  bus_selector4/141 -> outpmodule/500(VDDM_MCUActDisFail_flg)  "<VDDM_MCUActDisFail_flg>"
  bus_selector3/67 -> outpmodule/245(VBCM_SPTGDet_flg)  "<VBCM_SPTGDet_flg>"
  bus_selector12/18 -> outpmodule/747(VTPM_LRWheelDebug_flg)  "<VTPM_LRWheelDebug_flg>"
  bus_selector4/122 -> outpmodule/481(VDDM_RRWheelTmpHighDTC_raw32)  "<VDDM_RRWheelTmpHighDTC_raw32>"
  bus_selector3/53 -> outpmodule/231(VBCM_AmbLightBreath6_enum)  "<VBCM_AmbLightBreath6_enum>"
  bus_selector4/120 -> outpmodule/479(VDDM_RFWheelTmpHighDTC_raw32)  "<VDDM_RFWheelTmpHighDTC_raw32>"
  bus_selector3/19 -> outpmodule/197(VBCM_CTDLockSW_flg)  "<VBCM_CTDLockSW_flg>"
  outpmodule/663(VOUTP_FDRrAPTCHeatPwrCmd_W) -> bus_creator/663
  bus_selector4/117 -> outpmodule/476(VDDM_LRPressIndiDTC_raw32)  "<VDDM_LRPressIndiDTC_raw32>"
  bus_selector4/113 -> outpmodule/472(VDDM_LRBatwarnDTC_raw32)  "<VDDM_LRBatwarnDTC_raw32>"
  bus_selector3/17 -> outpmodule/195(VBCM_CTDCtrl_enum)  "<VBCM_CTDCtrl_enum>"
  bus_selector4/114 -> outpmodule/473(VDDM_RRBatwarnDTC_raw32)  "<VDDM_RRBatwarnDTC_raw32>"
  outpmodule/789(VOUTP_S4WheelDebugALTU_pct) -> bus_creator/789
  outpmodule/788(VOUTP_S3WheelDebugALTU_pct) -> bus_creator/788
  bus_selector10/41 -> outpmodule/643(VSYS_ModelYear_cnt)  "<VSYS_ModelYear_cnt>"
  outpmodule/787(VOUTP_S2WheelDebugALTU_pct) -> bus_creator/787
  bus_selector3/73 -> outpmodule/251(VBCM_MirrorFlodPos_flg)  "<VBCM_MirrorFlodPos_flg>"
  outpmodule/786(VOUTP_S1WheelDebugALTU_pct) -> bus_creator/786
  outpmodule/771(VOUTP_S1ID_raw32) -> bus_creator/771
  outpmodule/811(VOUTP_Flashchkdatavalid_enum) -> bus_creator/811
  bus_selector4/15 -> outpmodule/374(VDDM_C1ABM1LCDTC_raw32)  "<VDDM_C1ABM1LCDTC_raw32>"
  outpmodule/677(VOUTP_sigClntTHvBattOut_C) -> bus_creator/677
  outpmodule/769(VOUTP_LRSensorMode_flg) -> bus_creator/769
  outpmodule/765(VOUTP_CWheelTips_enum) -> bus_creator/765
  outpmodule/764(VOUTP_RRWheelPSW_raw8) -> bus_creator/764
  outpmodule/761(VOUTP_LFWheelPSW_raw8) -> bus_creator/761
  bus_selector9/47 -> outpmodule/601(VPMM_OTAPwrReqStdChkSta_enum)  "<VPMM_OTAPwrReqStdChkSta_enum>"
  outpmodule/760(VOUTP_RRWheelTmpIndi_flg) -> bus_creator/760
  outpmodule/759(VOUTP_LRWheelTmpIndi_flg) -> bus_creator/759
  outpmodule/757(VOUTP_LFWheelTmpIndi_flg) -> bus_creator/757
  outpmodule/756(VOUTP_TPMSWarnIndi_enum) -> bus_creator/756
  bus_selector3/179 -> outpmodule/357(VBCM_WinRROpenedSta_pct)  "<VBCM_WinRROpenedSta_pct>"
  outpmodule/776(VOUTP_S2L_enum) -> bus_creator/776
  outpmodule/753(VOUTP_RFPressIndi_enum) -> bus_creator/753
  bus_selector13/53 -> outpmodule/879(VTQD_RegenLimIndSta_flg)  "<VTQD_RegenLimIndSta_flg>"
  outpmodule/980(VOUTP_APSCtrlAvail_flg) -> bus_creator/980
  outpmodule/752(VOUTP_LFPressIndi_enum) -> bus_creator/752
  outpmodule/808(VOUTP_WriteChkfinRFID_raw) -> bus_creator/808
  outpmodule/809(VOUTP_WriteChkfinLRID_raw) -> bus_creator/809
  outpmodule/807(VOUTP_WriteChkfinLFID_raw) -> bus_creator/807
  bus_selector4/43 -> outpmodule/402(VDDM_FRDoorSWDTC_raw32)  "<VDDM_FRDoorSWDTC_raw32>"
  outpmodule/806(VOUTP_WriteChkRRID_raw) -> bus_creator/806
  outpmodule/804(VOUTP_WriteChkRFID_raw) -> bus_creator/804
  bus_selector4/17 -> outpmodule/376(VDDM_Lv2ErrDTC_raw32)  "<VDDM_Lv2ErrDTC_raw32>"
  bus_selector2/78 -> outpmodule/81(VAPM_RFPulseCount_enum)  "<VAPM_RFPulseCount_enum>"
  outpmodule/802(VOUTP_RRPindi_enum) -> bus_creator/802
  outpmodule/637(VOUTP_AcoreRebootCmdACK_flg) -> bus_creator/637
  outpmodule/238(VOUTP_AmbLightColor1_enum) -> bus_creator/238
  outpmodule/799(VOUTP_LFPindi_enum) -> bus_creator/799
  bus_selector1/2 -> outpmodule/2(VACC_LVBattVoltSta_enum)  "<VACC_LVBattVoltSta_enum>"
  outpmodule/797(VOUTP_ChkStorge_flg) -> bus_creator/797
  outpmodule/798(VOUTP_TPMSResButt_flg) -> bus_creator/798
  outpmodule/795(VOUTP_SetIDLoc_flg) -> bus_creator/795
  outpmodule/793(VOUTP_ID4messageALTU_raw8) -> bus_creator/793
  bus_selector4/145 -> outpmodule/504(VDDM_VCURLDoorSta_flg)  "<VDDM_VCURLDoorSta_flg>"
  outpmodule/794(VOUTP_Chkfin_flg) -> bus_creator/794
  bus_selector3/105 -> outpmodule/283(VBCM_AmbColorSta7_enum)  "<VBCM_AmbColorSta7_enum>"
  bus_selector2/173 -> outpmodule/176(VAPM_RAPSErrWarnSta_enum)  "<VAPM_RAPSErrWarnSta_enum>"
  bus_selector4/25 -> outpmodule/384(VDDM_MCU4PreDTC_raw32)  "<VDDM_MCU4PreDTC_raw32>"
  bus_selector2/172 -> outpmodule/175(VAPM_APSPwrReq_enum)  "<VAPM_APSPwrReq_enum>"
  bus_selector12/46 -> outpmodule/775(VTPM_S1L_enum)  "<VTPM_S1L_enum>"
  outpmodule/763(VOUTP_RFWheelPSW_raw8) -> bus_creator/763
  bus_selector2/170 -> outpmodule/173(VAPM_RAPSBCMLamp_enum)  "<VAPM_RAPSBCMLamp_enum>"
  bus_selector2/168 -> outpmodule/171(VAPM_APSSpeedCMD_kph)  "<VAPM_APSSpeedCMD_kph>"
  outpmodule/842(VOUTP_RrEDUActTq_Nm) -> bus_creator/842
  bus_selector3/110 -> outpmodule/288(VBCM_AmbBrightnessSta5_enum)  "<VBCM_AmbBrightnessSta5_enum>"
  BAPM_outputs/1 -> bus_selector2/1
  bus_selector4/76 -> outpmodule/435(VDDM_FCM2NoComDTC_raw32)  "<VDDM_FCM2NoComDTC_raw32>"
  bus_selector2/88 -> outpmodule/91(VAPM_EPSAOIControl_enum)  "<VAPM_EPSAOIControl_enum>"
  bus_selector4/73 -> outpmodule/432(VDDM_FLRUSSDTC_raw32)  "<VDDM_FLRUSSDTC_raw32>"
  outpmodule/857(VOUTP_FrIdcMax_A) -> bus_creator/857
  bus_selector2/70 -> outpmodule/73(VAPM_RFPulseCountV_flg)  "<VAPM_RFPulseCountV_flg>"
  bus_selector11/49 -> outpmodule/694(VTHC_AirIntenZone1M_enum)  "<VTHC_AirIntenZone1M_enum>"
  outpmodule/877(VOUTP_SetSpd_kph) -> bus_creator/877
  bus_selector11/82 -> outpmodule/727(VTHC_EWPBUflag1_flg)  "<VTHC_EWPBUflag1_flg>"
  bus_selector11/40 -> outpmodule/685(VTHC_ACModeMem_enum)  "<VTHC_ACModeMem_enum>"
  bus_selector4/46 -> outpmodule/405(VDDM_TailgaSWDTC_raw32)  "<VDDM_TailgaSWDTC_raw32>"
  bus_selector11/37 -> outpmodule/682(VTHC_sigCbnAirT_C)  "<VTHC_sigCbnAirT_C>"
  bus_selector16/89 -> outpmodule/978(VVMC_CCCtrlSta_enum)  "<VVMC_CCCtrlSta_enum>"
  bus_selector13/48 -> outpmodule/874(VTQD_FDCVCURegenMode_enum)  "<VTQD_FDCVCURegenMode_enum>"
  outpmodule/852(VOUTP_PTCSPermSta_flg) -> bus_creator/852
  bus_selector11/33 -> outpmodule/678(VTHC_sigCbnSolarLeft_W)  "<VTHC_sigCbnSolarLeft_W>"
  bus_selector13/50 -> outpmodule/876(VTQD_SpdCtrlSta_flg)  "<VTQD_SpdCtrlSta_flg>"
  bus_selector11/32 -> outpmodule/677(VTHC_sigClntTHvBattOut_C)  "<VTHC_sigClntTHvBattOut_C>"
  bus_selector4/128 -> outpmodule/487(VDDM_5vAPS1PwrErrDTC_raw32)  "<VDDM_5vAPS1PwrErrDTC_raw32>"
  bus_selector11/34 -> outpmodule/679(VTHC_sigClntTHvBattIn_C)  "<VTHC_sigClntTHvBattIn_C>"
  bus_selector11/30 -> outpmodule/675(VTHC_sigSetTempZon1St_C)  "<VTHC_sigSetTempZon1St_C>"
  bus_selector11/23 -> outpmodule/668(VTHC_CCUACLampSts_flg)  "<VTHC_CCUACLampSts_flg>"
  bus_selector13/49 -> outpmodule/875(VTQD_SpdCtrlMode_enum)  "<VTQD_SpdCtrlMode_enum>"
  bus_selector2/69 -> outpmodule/72(VAPM_LFPulseCountVTimeOut_flg)  "<VAPM_LFPulseCountVTimeOut_flg>"
  bus_selector11/21 -> outpmodule/666(VTHC_EDriveMode_enum)  "<VTHC_EDriveMode_enum>"
  outpmodule/662(VOUTP_FDFrRiAPTCHeatPwrCmd_W) -> bus_creator/662
  bus_selector11/17 -> outpmodule/662(VTHC_FDFrRiAPTCHeatPwrCmd_W)  "<VTHC_FDFrRiAPTCHeatPwrCmd_W>"
  bus_selector11/19 -> outpmodule/664(VTHC_FDBlowerCmd_pct)  "<VTHC_FDBlowerCmd_pct>"
  bus_selector11/15 -> outpmodule/660(VTHC_FDEWP3Cmd_enum)  "<VTHC_FDEWP3Cmd_enum>"
  bus_selector11/11 -> outpmodule/656(VTHC_CoolgFanActDuty_pct)  "<VTHC_CoolgFanActDuty_pct>"
  bus_selector2/90 -> outpmodule/93(VAPM_SASAngle_Deg)  "<VAPM_SASAngle_Deg>"
  bus_selector16/3 -> outpmodule/892(VVMC_VehicleSpeed_kph)  "<VVMC_VehicleSpeed_kph>"
  bus_selector11/7 -> outpmodule/652(VTHC_FDSOTXVCmd_flg)  "<VTHC_FDSOTXVCmd_flg>"
  outpmodule/836(VOUTP_RrActvDmpDisabReq_flg) -> bus_creator/836
  bus_selector11/80 -> outpmodule/725(VTHC_FDCFGSLearnCmd_enum)  "<VTHC_FDCFGSLearnCmd_enum>"
  bus_selector11/4 -> outpmodule/649(VTHC_FDSOV3Cmd_flg)  "<VTHC_FDSOV3Cmd_flg>"
  bus_selector11/5 -> outpmodule/650(VTHC_FDEXV1Cmd_step)  "<VTHC_FDEXV1Cmd_step>"
  outpmodule/956(VOUTP_ADASSLIFSta_enum) -> bus_creator/956
  bus_selector11/3 -> outpmodule/648(VTHC_FDSOV2Cmd_flg)  "<VTHC_FDSOV2Cmd_flg>"
  outpmodule/830(VOUTP_FrEDUAvailBrkRgnTq_Nm) -> bus_creator/830
  bus_selector16/58 -> outpmodule/947(VVMC_ADASWarningMsg_enum)  "<VVMC_ADASWarningMsg_enum>"
  bus_selector11/1 -> outpmodule/646(VTHC_FDCompCmd_rpm)  "<VTHC_FDCompCmd_rpm>"
  bus_selector4/31 -> outpmodule/390(VDDM_MidLvSaChkDTC_raw32)  "<VDDM_MidLvSaChkDTC_raw32>"
  bus_selector11/77 -> outpmodule/722(VTHC_FDCFGSChCmd_enum)  "<VTHC_FDCFGSChCmd_enum>"
  bus_selector12/72 -> outpmodule/801(VTPM_LRPindi_enum)  "<VTPM_LRPindi_enum>"
  bus_selector11/78 -> outpmodule/723(VTHC_FDCFGSIONSWSta_flg)  "<VTHC_FDCFGSIONSWSta_flg>"
  bus_selector11/74 -> outpmodule/719(VTHC_FDCFGSChSta_enum)  "<VTHC_FDCFGSChSta_enum>"
  outpmodule/648(VOUTP_FDSOV2Cmd_flg) -> bus_creator/648
  bus_selector11/24 -> outpmodule/669(VTHC_CCUAutoLampSts_flg)  "<VTHC_CCUAutoLampSts_flg>"
  outpmodule/848(VOUTP_FrEDUAvailBrkRgnTqV_flg) -> bus_creator/848
  bus_selector11/70 -> outpmodule/715(VTHC_CLVentEN_flg)  "<VTHC_CLVentEN_flg>"
  bus_selector11/68 -> outpmodule/713(VTHC_FDCTHCMAPTCForceOFFSta_flg)  "<VTHC_FDCTHCMAPTCForceOFFSta_flg>"
  outpmodule/240(VOUTP_AmbLightColor3_enum) -> bus_creator/240
  bus_selector11/67 -> outpmodule/712(VTHC_FDCTHCCRVentENSta_flg)  "<VTHC_FDCTHCCRVentENSta_flg>"
  bus_selector4/64 -> outpmodule/423(VDDM_FCLUSSDTC_raw32)  "<VDDM_FCLUSSDTC_raw32>"
  bus_selector2/171 -> outpmodule/174(VAPM_RAPSBCMLockReq_flg)  "<VAPM_RAPSBCMLockReq_flg>"
  bus_selector11/69 -> outpmodule/714(VTHC_DrVentEN_flg)  "<VTHC_DrVentEN_flg>"
  outpmodule/953(VOUTP_ADASLFCSta_enum) -> bus_creator/953
  outpmodule/803(VOUTP_WriteChkLFID_raw) -> bus_creator/803
  bus_selector12/31 -> outpmodule/760(VTPM_RRWheelTmpIndi_flg)  "<VTPM_RRWheelTmpIndi_flg>"
  bus_selector11/65 -> outpmodule/710(VTHC_FDCTHCPsVentENSta_flg)  "<VTHC_FDCTHCPsVentENSta_flg>"
  bus_selector16/51 -> outpmodule/940(VVMC_LeftTurnLightReq_flg)  "<VVMC_LeftTurnLightReq_flg>"
  bus_selector11/62 -> outpmodule/707(VTHC_FDCTHCCLEVentYSta_enum)  "<VTHC_FDCTHCCLEVentYSta_enum>"
  bus_selector11/64 -> outpmodule/709(VTHC_FDCTHCPsEVentYSta_enum)  "<VTHC_FDCTHCPsEVentYSta_enum>"
  bus_selector11/56 -> outpmodule/701(VTHC_FDCTHCDrEVentZSta_enum)  "<VTHC_FDCTHCDrEVentZSta_enum>"
  bus_selector11/83 -> outpmodule/728(VTHC_EWPBUflag2_flg)  "<VTHC_EWPBUflag2_flg>"
  bus_selector16/38 -> outpmodule/927(VVMC_ACCObjDist_m)  "<VVMC_ACCObjDist_m>"
  bus_selector11/54 -> outpmodule/699(VTHC_FDCTHCDrEVentModeSta_enum)  "<VTHC_FDCTHCDrEVentModeSta_enum>"
  BBCM_outputs/1 -> bus_selector3/1
  bus_selector11/51 -> outpmodule/696(VTHC_sigSetTempZon2StM_C)  "<VTHC_sigSetTempZon2StM_C>"
  bus_selector2/48 -> outpmodule/51(VAPM_LRRawWhlSpeed_kph)  "<VAPM_LRRawWhlSpeed_kph>"
  outpmodule/861(VOUTP_RrIdcMax_A) -> bus_creator/861
  bus_selector2/47 -> outpmodule/50(VAPM_RFRawWhlSpeedTimeOut_flg)  "<VAPM_RFRawWhlSpeedTimeOut_flg>"
  bus_selector2/45 -> outpmodule/48(VAPM_LFRawWhlSpeedTimeOut_flg)  "<VAPM_LFRawWhlSpeedTimeOut_flg>"
  bus_selector16/42 -> outpmodule/931(VVMC_ACCComfortBandUpper_mps2)  "<VVMC_ACCComfortBandUpper_mps2>"
  bus_selector2/43 -> outpmodule/46(VAPM_BrkPedalPosTimeOut_flg)  "<VAPM_BrkPedalPosTimeOut_flg>"
  bus_selector2/41 -> outpmodule/44(VAPM_ModOperation_enum)  "<VAPM_ModOperation_enum>"
  bus_selector2/42 -> outpmodule/45(VAPM_BrkPedalPos_pct)  "<VAPM_BrkPedalPos_pct>"
  bus_selector2/39 -> outpmodule/42(VAPM_SNSRLayout_enum)  "<VAPM_SNSRLayout_enum>"
  bus_selector2/33 -> outpmodule/36(VAPM_USSStaFML_flg)  "<VAPM_USSStaFML_flg>"
  bus_selector2/32 -> outpmodule/35(VAPM_USSStaFMR_flg)  "<VAPM_USSStaFMR_flg>"
  bus_selector2/167 -> outpmodule/170(VAPM_APSShiftPosnReq_enum)  "<VAPM_APSShiftPosnReq_enum>"
  bus_selector2/61 -> outpmodule/64(VAPM_LFWhlRotDirTimeOut_flg)  "<VAPM_LFWhlRotDirTimeOut_flg>"
  bus_selector2/100 -> outpmodule/103(VAPM_GRADE_Deg)  "<VAPM_GRADE_Deg>"
  bus_selector2/60 -> outpmodule/63(VAPM_LFWhlRotDir_enum)  "<VAPM_LFWhlRotDir_enum>"
  bus_selector2/58 -> outpmodule/61(VAPM_RRRawWhlSpeedV_flg)  "<VAPM_RRRawWhlSpeedV_flg>"
  bus_selector2/71 -> outpmodule/74(VAPM_RFPulseCountVTimeOut_flg)  "<VAPM_RFPulseCountVTimeOut_flg>"
  bus_selector2/55 -> outpmodule/58(VAPM_RFRawWhlSpeedVTimeOut_flg)  "<VAPM_RFRawWhlSpeedVTimeOut_flg>"
  outpmodule/766(VOUTP_AutoLTips_enum) -> bus_creator/766
  bus_selector2/52 -> outpmodule/55(VAPM_LFRawWhlSpeedV_flg)  "<VAPM_LFRawWhlSpeedV_flg>"
  bus_selector2/118 -> outpmodule/121(VAPM_BrkSwSta_flg)  "<VAPM_BrkSwSta_flg>"
  bus_selector16/46 -> outpmodule/935(VVMC_ADASShftPosnReqA_flg)  "<VVMC_ADASShftPosnReqA_flg>"
  outpmodule/141(VOUTP_AVMParkingmode_enum) -> bus_creator/141
  outpmodule/810(VOUTP_WriteChkfinRRID_raw) -> bus_creator/810
  outpmodule/144(VOUTP_AVMErrSTATimeOut_flg) -> bus_creator/144
  outpmodule/167(VOUTP_DKCParkingModeCmd_enum) -> bus_creator/167
  bus_selector3/24 -> outpmodule/202(VBCM_HBeam_flg)  "<VBCM_HBeam_flg>"
  outpmodule/140(VOUTP_AVMparkingexcuteTimeOut_flg) -> bus_creator/140
  bus_selector6/2 -> outpmodule/522(VDKC_DKCAuthSta_enum)  "<VDKC_DKCAuthSta_enum>"
  bus_selector11/28 -> outpmodule/673(VTHC_sigWindDirZon1St_enum)  "<VTHC_sigWindDirZon1St_enum>"
  outpmodule/138(VOUTP_AVMparkingcancelTimeOut_flg) -> bus_creator/138
  outpmodule/137(VOUTP_AVMparkingcancel_enum) -> bus_creator/137
  outpmodule/865(VOUTP_ExtShftAllow_flg) -> bus_creator/865
  bus_selector13/23 -> outpmodule/849(VTQD_RrEDUSpdValid_flg)  "<VTQD_RrEDUSpdValid_flg>"
  bus_selector2/54 -> outpmodule/57(VAPM_RFRawWhlSpeedV_flg)  "<VAPM_RFRawWhlSpeedV_flg>"
  outpmodule/128(VOUTP_ESCAPSStaTimeOut_flg) -> bus_creator/128
  outpmodule/125(VOUTP_ESCStandstill_flg) -> bus_creator/125
  bus_selector10/11 -> outpmodule/613(VSYS_Minor1_cnt)  "<VSYS_Minor1_cnt>"
  bus_selector16/29 -> outpmodule/918(VVMC_LKAStrToqReq_Nm)  "<VVMC_LKAStrToqReq_Nm>"
  bus_selector11/66 -> outpmodule/711(VTHC_FDCTHCCREVentYSta_enum)  "<VTHC_FDCTHCCREVentYSta_enum>"
  outpmodule/123(VOUTP_BrkSwV_flg) -> bus_creator/123
  outpmodule/859(VOUTP_FrUdcMax_V) -> bus_creator/859
  bus_selector2/133 -> outpmodule/136(VAPM_EPBStaTimeOut_flg)  "<VAPM_EPBStaTimeOut_flg>"
  bus_selector2/161 -> outpmodule/164(VAPM_APSRqEPASCtrl_flg)  "<VAPM_APSRqEPASCtrl_flg>"
  bus_selector2/137 -> outpmodule/140(VAPM_AVMparkingexcuteTimeOut_flg)  "<VAPM_AVMparkingexcuteTimeOut_flg>"
  bus_selector4/63 -> outpmodule/422(VDDM_DiagRRTSDTC_raw32)  "<VDDM_DiagRRTSDTC_raw32>"
  bus_selector2/136 -> outpmodule/139(VAPM_AVMparkingexcute_enum)  "<VAPM_AVMparkingexcute_enum>"
  bus_selector2/165 -> outpmodule/168(VAPM_PUIDLowPower_flg)  "<VAPM_PUIDLowPower_flg>"
  outpmodule/722(VOUTP_FDCFGSChCmd_enum) -> bus_creator/722
  outpmodule/720(VOUTP_FDCFGSAirIntCmd_enum) -> bus_creator/720
  bus_selector11/50 -> outpmodule/695(VTHC_fdefog_flg)  "<VTHC_fdefog_flg>"
  bus_selector2/169 -> outpmodule/172(VAPM_APSVMCReqA_flg)  "<VAPM_APSVMCReqA_flg>"
  outpmodule/768(VOUTP_RFSensorMode_flg) -> bus_creator/768
  outpmodule/714(VOUTP_DrVentEN_flg) -> bus_creator/714
  bus_selector2/99 -> outpmodule/102(VAPM_SASVTimeOut_flg)  "<VAPM_SASVTimeOut_flg>"
  outpmodule/713(VOUTP_FDCTHCMAPTCForceOFFSta_flg) -> bus_creator/713
  outpmodule/708(VOUTP_FDCTHCCLVentENSta_flg) -> bus_creator/708
  outpmodule/709(VOUTP_FDCTHCPsEVentYSta_enum) -> bus_creator/709
  outpmodule/707(VOUTP_FDCTHCCLEVentYSta_enum) -> bus_creator/707
  bus_selector4/10 -> outpmodule/369(VDDM_C3CCU2RCDTC_raw32)  "<VDDM_C3CCU2RCDTC_raw32>"
  outpmodule/778(VOUTP_S4L_enum) -> bus_creator/778
  outpmodule/704(VOUTP_FDCTHCCREVentZSta_enum) -> bus_creator/704
  bus_selector4/109 -> outpmodule/468(VDDM_FrMCUTqErrDTC_raw32)  "<VDDM_FrMCUTqErrDTC_raw32>"
  bus_selector3/44 -> outpmodule/222(VBCM_FrWiperH_flg)  "<VBCM_FrWiperH_flg>"
  outpmodule/705(VOUTP_FDCTHCDrEVentYSta_enum) -> bus_creator/705
  outpmodule/747(VOUTP_LRWheelDebug_flg) -> bus_creator/747
  bus_selector10/37 -> outpmodule/639(VSYS_ECUGen1_cnt)  "<VSYS_ECUGen1_cnt>"
  bus_selector4/67 -> outpmodule/426(VDDM_FCRUSSDTC_raw32)  "<VDDM_FCRUSSDTC_raw32>"
  outpmodule/702(VOUTP_FDCTHCCLEVentZSta_enum) -> bus_creator/702
  outpmodule/703(VOUTP_FDCTHCPsEVentZSta_enum) -> bus_creator/703
  bus_selector12/40 -> outpmodule/769(VTPM_LRSensorMode_flg)  "<VTPM_LRSensorMode_flg>"
  outpmodule/701(VOUTP_FDCTHCDrEVentZSta_enum) -> bus_creator/701
  outpmodule/700(VOUTP_FDCTHCPsEVentModeSta_enum) -> bus_creator/700
  outpmodule/832(VOUTP_EVDriveMode_enum) -> bus_creator/832
  bus_selector10/6 -> outpmodule/608(VSYS_CarModel3_cnt)  "<VSYS_CarModel3_cnt>"
  outpmodule/699(VOUTP_FDCTHCDrEVentModeSta_enum) -> bus_creator/699
  bus_selector12/33 -> outpmodule/762(VTPM_LRWheelPSW_raw8)  "<VTPM_LRWheelPSW_raw8>"
  bus_selector3/145 -> outpmodule/323(VBCM_PTGUserHeight5_cnt)  "<VBCM_PTGUserHeight5_cnt>"
  outpmodule/775(VOUTP_S1L_enum) -> bus_creator/775
  bus_selector6/7 -> outpmodule/527(VDKC_KeyAreaPS_enum)  "<VDKC_KeyAreaPS_enum>"
  bus_selector11/45 -> outpmodule/690(VTHC_FootM_flg)  "<VTHC_FootM_flg>"
  outpmodule/697(VOUTP_sigDfrstSt_flg) -> bus_creator/697
  outpmodule/813(VOUTP_unlearnSfali_flg) -> bus_creator/813
  outpmodule/692(VOUTP_ACForceOFF_flg) -> bus_creator/692
  bus_selector4/90 -> outpmodule/449(VDDM_RrMCUSigErrDetDTC_raw32)  "<VDDM_RrMCUSigErrDetDTC_raw32>"
  outpmodule/693(VOUTP_RecAutoFlg_flg) -> bus_creator/693
  bus_selector7/4 -> outpmodule/542(VDSC_DISCButtSta_flg)  "<VDSC_DISCButtSta_flg>"
  bus_selector16/33 -> outpmodule/922(VVMC_ADASFaultSta_flg)  "<VVMC_ADASFaultSta_flg>"
  outpmodule/694(VOUTP_AirIntenZone1M_enum) -> bus_creator/694
  bus_selector12/70 -> outpmodule/799(VTPM_LFPindi_enum)  "<VTPM_LFPindi_enum>"
  outpmodule/691(VOUTP_CCUSyncSts_flg) -> bus_creator/691
  outpmodule/284(VOUTP_AmbBrightnessSta1_enum) -> bus_creator/284
  outpmodule/721(VOUTP_FDCFGSFuncSta_flg) -> bus_creator/721
  outpmodule/690(VOUTP_FootM_flg) -> bus_creator/690
  outpmodule/689(VOUTP_FaceM_flg) -> bus_creator/689
  outpmodule/781(VOUTP_RFP20_raw8) -> bus_creator/781
  outpmodule/688(VOUTP_Frost_flg) -> bus_creator/688
  outpmodule/889(VOUTP_HVPO120VGrpBLDSt_enum) -> bus_creator/889
  bus_selector11/52 -> outpmodule/697(VTHC_sigDfrstSt_flg)  "<VTHC_sigDfrstSt_flg>"
  outpmodule/687(VOUTP_Foot_flg) -> bus_creator/687
  outpmodule/685(VOUTP_ACModeMem_enum) -> bus_creator/685
  outpmodule/745(VOUTP_RRSensorFail_flg) -> bus_creator/745
  outpmodule/954(VOUTP_ADASLaneModeL_enum) -> bus_creator/954
  outpmodule/286(VOUTP_AmbBrightnessSta3_enum) -> bus_creator/286
  outpmodule/805(VOUTP_WriteChkLRID_raw) -> bus_creator/805
  bus_selector15/2 -> outpmodule/884(VV2L_ReqV2LIVIPopup_enum)  "<VV2L_ReqV2LIVIPopup_enum>"
  outpmodule/744(VOUTP_LRSensorFail_flg) -> bus_creator/744
  bus_selector10/5 -> outpmodule/607(VSYS_CarModel2_cnt)  "<VSYS_CarModel2_cnt>"
  outpmodule/742(VOUTP_LFSensorFail_flg) -> bus_creator/742
  bus_selector3/85 -> outpmodule/263(VBCM_AmbLinkDriSta_flg)  "<VBCM_AmbLinkDriSta_flg>"
  bus_selector12/71 -> outpmodule/800(VTPM_RFPind_enum)  "<VTPM_RFPind_enum>"
  bus_selector4/75 -> outpmodule/434(VDDM_RLRUSSDTC_raw32)  "<VDDM_RLRUSSDTC_raw32>"
  bus_selector4/86 -> outpmodule/445(VDDM_ZoneSCPNoComDTC_raw32)  "<VDDM_ZoneSCPNoComDTC_raw32>"
  bus_selector2/50 -> outpmodule/53(VAPM_RRRawWhlSpeed_kph)  "<VAPM_RRRawWhlSpeed_kph>"
  outpmodule/696(VOUTP_sigSetTempZon2StM_C) -> bus_creator/696
  outpmodule/888(VOUTP_HVPO120VGrpALDSt_enum) -> bus_creator/888
  bus_selector13/44 -> outpmodule/870(VTQD_IVIPwrLockSta_enum)  "<VTQD_IVIPwrLockSta_enum>"
  outpmodule/740(VOUTP_LRWheelTemp_C) -> bus_creator/740
  bus_selector13/3 -> outpmodule/829(VTQD_TqSourceRr_enum)  "<VTQD_TqSourceRr_enum>"
  outpmodule/712(VOUTP_FDCTHCCRVentENSta_flg) -> bus_creator/712
  outpmodule/739(VOUTP_RFWheelTemp_C) -> bus_creator/739
  outpmodule/738(VOUTP_LFWheelTemp_C) -> bus_creator/738
  outpmodule/686(VOUTP_Face_flg) -> bus_creator/686
  outpmodule/737(VOUTP_RRWheelPress_raw8) -> bus_creator/737
  bus_selector2/46 -> outpmodule/49(VAPM_RFRawWhlSpeed_kph)  "<VAPM_RFRawWhlSpeed_kph>"
  outpmodule/736(VOUTP_LRWheelPress_raw8) -> bus_creator/736
  outpmodule/735(VOUTP_RFWheelPress_raw8) -> bus_creator/735
  bus_selector9/19 -> outpmodule/573(VPMM_PwrStaConstraint_enum)  "<VPMM_PwrStaConstraint_enum>"
  bus_selector2/44 -> outpmodule/47(VAPM_LFRawWhlSpeed_kph)  "<VAPM_LFRawWhlSpeed_kph>"
  outpmodule/734(VOUTP_LFWheelPress_raw8) -> bus_creator/734
  bus_selector12/90 -> outpmodule/819(VTPM_FlashS4ID_raw)  "<VTPM_FlashS4ID_raw>"
  bus_selector2/79 -> outpmodule/82(VAPM_RFPulseCountTimeOut_flg)  "<VAPM_RFPulseCountTimeOut_flg>"
  outpmodule/887(VOUTP_ReqOBCIntrV2LEna_enum) -> bus_creator/887
  BTQD_outputs/1 -> bus_selector13/1
  outpmodule/733(VOUTP_RRBatWarn_flg) -> bus_creator/733
  outpmodule/731(VOUTP_RFBatWarn_flg) -> bus_creator/731
  outpmodule/748(VOUTP_RFWheelDebug_flg) -> bus_creator/748
  bus_selector13/33 -> outpmodule/859(VTQD_FrUdcMax_V)  "<VTQD_FrUdcMax_V>"
  outpmodule/730(VOUTP_LFBatWarn_flg) -> bus_creator/730
  bus_selector5/6 -> outpmodule/520(VDHP_EAPS2NRM_pct)  "<VDHP_EAPS2NRM_pct>"
  outpmodule/725(VOUTP_FDCFGSLearnCmd_enum) -> bus_creator/725
  bus_selector12/37 -> outpmodule/766(VTPM_AutoLTips_enum)  "<VTPM_AutoLTips_enum>"
  outpmodule/724(VOUTP_FDCFGSIONCmd_flg) -> bus_creator/724
  outpmodule/256(VOUTP_PasWdwCtrlCmd_pct) -> bus_creator/256
  bus_selector11/12 -> outpmodule/657(VTHC_FDAGSCmd_enum)  "<VTHC_FDAGSCmd_enum>"
  outpmodule/165(VOUTP_CAASSta_enum) -> bus_creator/165
  bus_selector2/147 -> outpmodule/150(VAPM_IVIScreenTimeOut_flg)  "<VAPM_IVIScreenTimeOut_flg>"
  bus_selector2/143 -> outpmodule/146(VAPM_IVIStatusTimeOut_flg)  "<VAPM_IVIStatusTimeOut_flg>"
  outpmodule/680(VOUTP_sigCbnSolarRight_W) -> bus_creator/680
  bus_selector2/146 -> outpmodule/149(VAPM_IVIScreen_enum)  "<VAPM_IVIScreen_enum>"
  bus_selector2/166 -> outpmodule/169(VAPM_CAASVMCReqA_flg)  "<VAPM_CAASVMCReqA_flg>"
  bus_selector13/51 -> outpmodule/877(VTQD_SetSpd_kph)  "<VTQD_SetSpd_kph>"
  outpmodule/758(VOUTP_RFWheelTmpIndi_flg) -> bus_creator/758
  bus_selector2/157 -> outpmodule/160(VAPM_APSHWVer_enum)  "<VAPM_APSHWVer_enum>"
  outpmodule/304(VOUTP_FDHandleCmd_enum) -> bus_creator/304
  bus_selector2/160 -> outpmodule/163(VAPM_APSVRqEPASCtrl_flg)  "<VAPM_APSVRqEPASCtrl_flg>"
  bus_selector2/158 -> outpmodule/161(VAPM_APSExitCondition_enum)  "<VAPM_APSExitCondition_enum>"
  outpmodule/267(VOUTP_AmbBrightSta_enum) -> bus_creator/267
  bus_selector16/79 -> outpmodule/968(VVMC_ADASLanetypeR_enum)  "<VVMC_ADASLanetypeR_enum>"
  bus_selector2/162 -> outpmodule/165(VAPM_CAASSta_enum)  "<VAPM_CAASSta_enum>"
  bus_selector2/152 -> outpmodule/155(VAPM_DriverSeatBeltCmd_flg)  "<VAPM_DriverSeatBeltCmd_flg>"
  outpmodule/259(VOUTP_APMDoorControlSta_flg) -> bus_creator/259
  bus_selector2/149 -> outpmodule/152(VAPM_ABSActiveTimeOut_flg)  "<VAPM_ABSActiveTimeOut_flg>"
  bus_selector12/28 -> outpmodule/757(VTPM_LFWheelTmpIndi_flg)  "<VTPM_LFWheelTmpIndi_flg>"
  bus_selector3/125 -> outpmodule/303(VBCM_FDRHandleLampCmd_flg)  "<VBCM_FDRHandleLampCmd_flg>"
  bus_selector11/20 -> outpmodule/665(VTHC_BatteryMode_enum)  "<VTHC_BatteryMode_enum>"
  outpmodule/153(VOUTP_TCSActive_flg) -> bus_creator/153
  bus_selector16/78 -> outpmodule/967(VVMC_FCMACCmode_enum)  "<VVMC_FCMACCmode_enum>"
  bus_selector3/123 -> outpmodule/301(VBCM_TurnSwTimeSetSta457_enum)  "<VBCM_TurnSwTimeSetSta457_enum>"
  bus_selector3/126 -> outpmodule/304(VBCM_FDHandleCmd_enum)  "<VBCM_FDHandleCmd_enum>"
  outpmodule/394(VOUTP_MCUActDTC_raw32) -> bus_creator/394
  outpmodule/392(VOUTP_DCDCDisDTC_raw32) -> bus_creator/392
  outpmodule/784(VOUTP_FAT_flg) -> bus_creator/784
  outpmodule/393(VOUTP_HVRlyOpDTC_raw32) -> bus_creator/393
  bus_selector13/21 -> outpmodule/847(VTQD_FrEDUSpdValid_flg)  "<VTQD_FrEDUSpdValid_flg>"
  outpmodule/388(VOUTP_DCDCEnaDTC_raw32) -> bus_creator/388
  bus_selector2/82 -> outpmodule/85(VAPM_RRPulseCount_enum)  "<VAPM_RRPulseCount_enum>"
  outpmodule/386(VOUTP_HVRlyCloDTC_raw32) -> bus_creator/386
  outpmodule/385(VOUTP_DCDC4PreDTC_raw32) -> bus_creator/385
  bus_selector4/70 -> outpmodule/429(VDDM_RMRUSSDTC_raw32)  "<VDDM_RMRUSSDTC_raw32>"
  outpmodule/384(VOUTP_MCU4PreDTC_raw32) -> bus_creator/384
  bus_selector16/30 -> outpmodule/919(VVMC_LKATOIFault_flg)  "<VVMC_LKATOIFault_flg>"
  bus_selector3/114 -> outpmodule/292(VBCM_PassSWSta_flg)  "<VBCM_PassSWSta_flg>"
  outpmodule/382(VOUTP_ONtoRdyDTC_raw32) -> bus_creator/382
  outpmodule/381(VOUTP_KeyAuthDTC_raw32) -> bus_creator/381
  outpmodule/868(VOUTP_DriveProtEn_flg) -> bus_creator/868
  outpmodule/379(VOUTP_BrkSWErrDTC_raw32) -> bus_creator/379
  bus_selector16/96 -> outpmodule/985(VVMC_APSReq_enum)  "<VVMC_APSReq_enum>"
  bus_selector9/12 -> outpmodule/566(VPMM_HVPwrSta_flg)  "<VPMM_HVPwrSta_flg>"
  bus_selector11/2 -> outpmodule/647(VTHC_FDSOV1Cmd_flg)  "<VTHC_FDSOV1Cmd_flg>"
  outpmodule/375(VOUTP_Lv1ErrDTC_raw32) -> bus_creator/375
  BDDM_outputs/1 -> bus_selector4/1
  outpmodule/371(VOUTP_C3CCU2LCDTC_raw32) -> bus_creator/371
  outpmodule/943(VOUTP_ADASFltWrnReq_flg) -> bus_creator/943
  bus_selector10/18 -> outpmodule/620(VSYS_Dash1_cnt)  "<VSYS_Dash1_cnt>"
  outpmodule/372(VOUTP_C1ABM1RCDTC_raw32) -> bus_creator/372
  outpmodule/892(VOUTP_VehicleSpeed_kph) -> bus_creator/892
  outpmodule/370(VOUTP_C3CCU2CSDTC_raw32) -> bus_creator/370
  bus_selector11/42 -> outpmodule/687(VTHC_Foot_flg)  "<VTHC_Foot_flg>"
  outpmodule/369(VOUTP_C3CCU2RCDTC_raw32) -> bus_creator/369
  bus_selector3/15 -> outpmodule/193(VBCM_RrChargingDoorCtrl_enum)  "<VBCM_RrChargingDoorCtrl_enum>"
  outpmodule/368(VOUTP_C3CCU1LCDTC_raw32) -> bus_creator/368
  bus_selector4/69 -> outpmodule/428(VDDM_RMLUSSDTC_raw32)  "<VDDM_RMLUSSDTC_raw32>"
  bus_selector2/154 -> outpmodule/157(VAPM_APSProgressPCT_pct)  "<VAPM_APSProgressPCT_pct>"
  outpmodule/431(VOUTP_FLLUSSDTC_raw32) -> bus_creator/431
  outpmodule/429(VOUTP_RMRUSSDTC_raw32) -> bus_creator/429
  bus_selector12/80 -> outpmodule/809(VTPM_WriteChkfinLRID_raw)  "<VTPM_WriteChkfinLRID_raw>"
  outpmodule/430(VOUTP_RCRUSSDTC_raw32) -> bus_creator/430
  bus_selector2/139 -> outpmodule/142(VAPM_AVMParkingmodeTimeOut_flg)  "<VAPM_AVMParkingmodeTimeOut_flg>"
  outpmodule/428(VOUTP_RMLUSSDTC_raw32) -> bus_creator/428
  outpmodule/427(VOUTP_RCLUSSDTC_raw32) -> bus_creator/427
  outpmodule/426(VOUTP_FCRUSSDTC_raw32) -> bus_creator/426
  bus_selector11/6 -> outpmodule/651(VTHC_FDEXV2Cmd_step)  "<VTHC_FDEXV2Cmd_step>"
  bus_selector4/23 -> outpmodule/382(VDDM_ONtoRdyDTC_raw32)  "<VDDM_ONtoRdyDTC_raw32>"
  outpmodule/425(VOUTP_FMRUSSDTC_raw32) -> bus_creator/425
  outpmodule/423(VOUTP_FCLUSSDTC_raw32) -> bus_creator/423
  outpmodule/422(VOUTP_DiagRRTSDTC_raw32) -> bus_creator/422
  bus_selector11/58 -> outpmodule/703(VTHC_FDCTHCPsEVentZSta_enum)  "<VTHC_FDCTHCPsEVentZSta_enum>"
  bus_selector2/156 -> outpmodule/159(VAPM_APSSWVer_enum)  "<VAPM_APSSWVer_enum>"
  outpmodule/424(VOUTP_FMLUSSDTC_raw32) -> bus_creator/424
  bus_selector2/62 -> outpmodule/65(VAPM_RFWhlRotDir_enum)  "<VAPM_RFWhlRotDir_enum>"
  outpmodule/963(VOUTP_LVDAFailinfo_flg) -> bus_creator/963
  bus_selector16/82 -> outpmodule/971(VVMC_ADASLanecurveR_raw32)  "<VVMC_ADASLanecurveR_raw32>"
  outpmodule/420(VOUTP_DiagFRTSDTC_raw32) -> bus_creator/420
  bus_selector2/141 -> outpmodule/144(VAPM_AVMErrSTATimeOut_flg)  "<VAPM_AVMErrSTATimeOut_flg>"
  bus_selector12/25 -> outpmodule/754(VTPM_LRPressIndi_enum)  "<VTPM_LRPressIndi_enum>"
  bus_selector11/76 -> outpmodule/721(VTHC_FDCFGSFuncSta_flg)  "<VTHC_FDCFGSFuncSta_flg>"
  outpmodule/421(VOUTP_DiagRLTSDTC_raw32) -> bus_creator/421
  outpmodule/418(VOUTP_DiagHCrashDTC_raw32) -> bus_creator/418
  outpmodule/292(VOUTP_PassSWSta_flg) -> bus_creator/292
  bus_selector16/67 -> outpmodule/956(VVMC_ADASSLIFSta_enum)  "<VVMC_ADASSLIFSta_enum>"
  outpmodule/417(VOUTP_EnterNewOperCyc_flg) -> bus_creator/417
  outpmodule/416(VOUTP_ESC5NoComDTC_raw32) -> bus_creator/416
  outpmodule/774(VOUTP_S4ID_raw32) -> bus_creator/774
  bus_selector13/15 -> outpmodule/841(VTQD_FrEDUActTq_Nm)  "<VTQD_FrEDUActTq_Nm>"
  outpmodule/413(VOUTP_Shifter1NoComDTC_raw32) -> bus_creator/413
  bus_selector11/29 -> outpmodule/674(VTHC_sigRecircSt_flg)  "<VTHC_sigRecircSt_flg>"
  outpmodule/414(VOUTP_ESC7NoComDTC_raw32) -> bus_creator/414
  bus_selector4/131 -> outpmodule/490(VDDM_EPBUnlockTODTC_raw32)  "<VDDM_EPBUnlockTODTC_raw32>"
  bus_selector11/13 -> outpmodule/658(VTHC_FDEWP1Cmd_enum)  "<VTHC_FDEWP1Cmd_enum>"
  outpmodule/415(VOUTP_ESC1NoComDTC_raw32) -> bus_creator/415
  outpmodule/412(VOUTP_MCUR1NoComDTC_raw32) -> bus_creator/412
  bus_selector12/19 -> outpmodule/748(VTPM_RFWheelDebug_flg)  "<VTPM_RFWheelDebug_flg>"
  bus_selector16/15 -> outpmodule/904(VVMC_SingleWhlSlipRatioCtrl_flg)  "<VVMC_SingleWhlSlipRatioCtrl_flg>"
  bus_selector4/66 -> outpmodule/425(VDDM_FMRUSSDTC_raw32)  "<VDDM_FMRUSSDTC_raw32>"
  outpmodule/410(VOUTP_APSCorrErrDTC_raw32) -> bus_creator/410
  outpmodule/818(VOUTP_FlashS3ID_raw) -> bus_creator/818
  outpmodule/409(VOUTP_APS2SigOoRDTC_raw32) -> bus_creator/409
  outpmodule/408(VOUTP_APS1SigOoRDTC_raw32) -> bus_creator/408
  outpmodule/406(VOUTP_EDriveSysErrVCUErr_flg) -> bus_creator/406
  outpmodule/405(VOUTP_TailgaSWDTC_raw32) -> bus_creator/405
  outpmodule/717(VOUTP_CRVentEN_flg) -> bus_creator/717
  outpmodule/403(VOUTP_RRDoorSWDTC_raw32) -> bus_creator/403
  outpmodule/780(VOUTP_LFP20_raw8) -> bus_creator/780
  outpmodule/402(VOUTP_FRDoorSWDTC_raw32) -> bus_creator/402
  outpmodule/401(VOUTP_RLDoorSWDTC_raw32) -> bus_creator/401
  bus_selector4/94 -> outpmodule/453(VDDM_CCMalfuncDetDTC_raw32)  "<VDDM_CCMalfuncDetDTC_raw32>"
  outpmodule/400(VOUTP_FLDoorSWDTC_raw32) -> bus_creator/400
  bus_selector12/49 -> outpmodule/778(VTPM_S4L_enum)  "<VTPM_S4L_enum>"
  outpmodule/398(VOUTP_LVSupHiDTC_raw32) -> bus_creator/398
  bus_selector12/11 -> outpmodule/740(VTPM_LRWheelTemp_C)  "<VTPM_LRWheelTemp_C>"
  bus_selector11/48 -> outpmodule/693(VTHC_RecAutoFlg_flg)  "<VTHC_RecAutoFlg_flg>"
  bus_selector2/134 -> outpmodule/137(VAPM_AVMparkingcancel_enum)  "<VAPM_AVMparkingcancel_enum>"
  outpmodule/397(VOUTP_LVSupLoDTC_raw32) -> bus_creator/397
  bus_selector4/36 -> outpmodule/395(VDDM_OBC4PreDTC_raw32)  "<VDDM_OBC4PreDTC_raw32>"
  outpmodule/396(VOUTP_IniLVLoDTC_raw32) -> bus_creator/396
  bus_selector2/127 -> outpmodule/130(VAPM_EPBExtReleaseAvailTimeOut_flg)  "<VAPM_EPBExtReleaseAvailTimeOut_flg>"
  bus_selector2/57 -> outpmodule/60(VAPM_LRRawWhlSpeedVTimeOut_flg)  "<VAPM_LRRawWhlSpeedVTimeOut_flg>"
  bus_selector2/128 -> outpmodule/131(VAPM_EPBExtApplyAvail_flg)  "<VAPM_EPBExtApplyAvail_flg>"
  bus_selector4/3 -> outpmodule/362(VDDM_C3BMS6LCDTC_raw32)  "<VDDM_C3BMS6LCDTC_raw32>"
  bus_selector2/49 -> outpmodule/52(VAPM_LRRawWhlSpeedTimeOut_flg)  "<VAPM_LRRawWhlSpeedTimeOut_flg>"
  bus_selector2/115 -> outpmodule/118(VAPM_LongAccelVTimeOut_flg)  "<VAPM_LongAccelVTimeOut_flg>"
  bus_selector4/110 -> outpmodule/469(VDDM_RrMCUTqErrDTC_raw32)  "<VDDM_RrMCUTqErrDTC_raw32>"
  outpmodule/792(VOUTP_ID3messageALTU_raw8) -> bus_creator/792
  bus_selector4/45 -> outpmodule/404(VDDM_HoodSWDTC_raw32)  "<VDDM_HoodSWDTC_raw32>"
  bus_selector2/116 -> outpmodule/119(VAPM_MCPressureV_bar)  "<VAPM_MCPressureV_bar>"
  bus_selector2/114 -> outpmodule/117(VAPM_LongAccelV_flg)  "<VAPM_LongAccelV_flg>"
  outpmodule/831(VOUTP_RrEDUAvailBrkRgnTq_Nm) -> bus_creator/831
  outpmodule/294(VOUTP_FWasSwSta_enum) -> bus_creator/294
  bus_selector16/39 -> outpmodule/928(VVMC_ACCObjRelSpd_mps)  "<VVMC_ACCObjRelSpd_mps>"
  bus_selector2/112 -> outpmodule/115(VAPM_LatAccelV_flg)  "<VAPM_LatAccelV_flg>"
  outpmodule/399(VOUTP_DrStSWDTC_raw32) -> bus_creator/399
  bus_selector6/14 -> outpmodule/534(VDKC_DkeyAreaRAPSSta_enum)  "<VDKC_DkeyAreaRAPSSta_enum>"
  bus_selector2/155 -> outpmodule/158(VAPM_APSRQDisplay_enum)  "<VAPM_APSRQDisplay_enum>"
  outpmodule/299(VOUTP_OutMode_enum) -> bus_creator/299
  outpmodule/715(VOUTP_CLVentEN_flg) -> bus_creator/715
  bus_selector2/111 -> outpmodule/114(VAPM_YawRateVTimeOut_flg)  "<VAPM_YawRateVTimeOut_flg>"
  outpmodule/252(VOUTP_FuelDoorPos_flg) -> bus_creator/252
  bus_selector2/110 -> outpmodule/113(VAPM_YawRateV_flg)  "<VAPM_YawRateV_flg>"
  bus_selector2/108 -> outpmodule/111(VAPM_MCPressure_bar)  "<VAPM_MCPressure_bar>"
  bus_selector2/106 -> outpmodule/109(VAPM_LongAccel_Gps)  "<VAPM_LongAccel_Gps>"
  bus_selector2/102 -> outpmodule/105(VAPM_YawRate_degps)  "<VAPM_YawRate_degps>"
  bus_selector4/9 -> outpmodule/368(VDDM_C3CCU1LCDTC_raw32)  "<VDDM_C3CCU1LCDTC_raw32>"
  outpmodule/407(VOUTP_VehMalfunLevel_enum) -> bus_creator/407
  outpmodule/277(VOUTP_AmbODAENFlash_enum) -> bus_creator/277
  bus_selector2/104 -> outpmodule/107(VAPM_LatAccel_Gps)  "<VAPM_LatAccel_Gps>"
  bus_selector16/57 -> outpmodule/946(VVMC_ACCTakeoverReq_flg)  "<VVMC_ACCTakeoverReq_flg>"
  bus_selector2/103 -> outpmodule/106(VAPM_YawRateTimeOut_flg)  "<VAPM_YawRateTimeOut_flg>"
  outpmodule/746(VOUTP_LFWheelDebug_flg) -> bus_creator/746
  outpmodule/457(VOUTP_MCUR1RCErrDTC_raw32) -> bus_creator/457
  bus_selector5/4 -> outpmodule/518(VDHP_ResetPedalZeroPosStart_flg)  "<VDHP_ResetPedalZeroPosStart_flg>"
  bus_selector16/18 -> outpmodule/907(VVMC_SPD2ACCAct_flg)  "<VVMC_SPD2ACCAct_flg>"
  outpmodule/453(VOUTP_CCMalfuncDetDTC_raw32) -> bus_creator/453
  outpmodule/452(VOUTP_ACCMalfuncDetDTC_raw32) -> bus_creator/452
  outpmodule/450(VOUTP_CCUSigErrDetDTC_raw32) -> bus_creator/450
  outpmodule/451(VOUTP_ACCAccelCmdErrDetDTC_raw32) -> bus_creator/451
  outpmodule/448(VOUTP_FrMCUSigErrDetDTC_raw32) -> bus_creator/448
  outpmodule/447(VOUTP_FCMACCSigErrDetDTC_raw32) -> bus_creator/447
  outpmodule/446(VOUTP_BMSSigErrDetDTC_raw32) -> bus_creator/446
  bus_selector2/135 -> outpmodule/138(VAPM_AVMparkingcancelTimeOut_flg)  "<VAPM_AVMparkingcancelTimeOut_flg>"
  bus_selector16/27 -> outpmodule/916(VVMC_LateralCtrl_flg)  "<VVMC_LateralCtrl_flg>"
  outpmodule/442(VOUTP_FCM4CSErrDTC_raw32) -> bus_creator/442
  outpmodule/777(VOUTP_S3L_enum) -> bus_creator/777
  outpmodule/438(VOUTP_FCM3NoComDTC_raw32) -> bus_creator/438
  outpmodule/500(VOUTP_MCUActDisFail_flg) -> bus_creator/500
  outpmodule/502(VOUTP_VCUFLDoorSta_flg) -> bus_creator/502
  outpmodule/853(VOUTP_FrRgnPermSta_flg) -> bus_creator/853
  outpmodule/497(VOUTP_EDriveSysErrShifterErr_flg) -> bus_creator/497
  outpmodule/493(VOUTP_EngagePFail_flg) -> bus_creator/493
  outpmodule/495(VOUTP_VCURAPSErrLv2_flg) -> bus_creator/495
  outpmodule/492(VOUTP_DTCDetect_enum) -> bus_creator/492
  bus_selector11/47 -> outpmodule/692(VTHC_ACForceOFF_flg)  "<VTHC_ACForceOFF_flg>"
  BACC_outputs/1 -> bus_selector1/1
  outpmodule/490(VOUTP_EPBUnlockTODTC_raw32) -> bus_creator/490
  bus_selector15/7 -> outpmodule/889(VV2L_HVPO120VGrpBLDSt_enum)  "<VV2L_HVPO120VGrpBLDSt_enum>"
  outpmodule/488(VOUTP_5vAPS2PwrErrDTC_raw32) -> bus_creator/488
  outpmodule/485(VOUTP_RRSensorFailDTC_raw32) -> bus_creator/485
  bus_selector12/45 -> outpmodule/774(VTPM_S4ID_raw32)  "<VTPM_S4ID_raw32>"
  outpmodule/779(VOUTP_ALFin_flg) -> bus_creator/779
  outpmodule/481(VOUTP_RRWheelTmpHighDTC_raw32) -> bus_creator/481
  outpmodule/893(VOUTP_MeterIndSpeed_raw32) -> bus_creator/893
  outpmodule/483(VOUTP_RFSensorFailDTC_raw32) -> bus_creator/483
  outpmodule/482(VOUTP_LFSensorFailDTC_raw32) -> bus_creator/482
  outpmodule/480(VOUTP_LRWheelTmpHighDTC_raw32) -> bus_creator/480
  bus_selector3/161 -> outpmodule/339(VBCM_HMIKey1FuncSta_enum)  "<VBCM_HMIKey1FuncSta_enum>"
  outpmodule/478(VOUTP_LFWheelTmpHighDTC_raw32) -> bus_creator/478
  outpmodule/469(VOUTP_RrMCUTqErrDTC_raw32) -> bus_creator/469
  outpmodule/468(VOUTP_FrMCUTqErrDTC_raw32) -> bus_creator/468
  bus_selector11/26 -> outpmodule/671(VTHC_CCUSyncLampSts_flg)  "<VTHC_CCUSyncLampSts_flg>"
  bus_selector3/37 -> outpmodule/215(VBCM_MirrorDefog_flg)  "<VBCM_MirrorDefog_flg>"
  bus_selector2/101 -> outpmodule/104(VAPM_GRADETimeOut_flg)  "<VAPM_GRADETimeOut_flg>"
  outpmodule/466(VOUTP_ESC5RCErrDTC_raw32) -> bus_creator/466
  bus_selector3/177 -> outpmodule/355(VBCM_WinRFOpenedSta_pct)  "<VBCM_WinRFOpenedSta_pct>"
  bus_selector2/36 -> outpmodule/39(VAPM_USSStaFCR_flg)  "<VAPM_USSStaFCR_flg>"
  outpmodule/462(VOUTP_ESC7RCErrDTC_raw32) -> bus_creator/462
  outpmodule/463(VOUTP_ESC7CSErrDTC_raw32) -> bus_creator/463
  bus_selector10/9 -> outpmodule/611(VSYS_Major1_cnt)  "<VSYS_Major1_cnt>"
  outpmodule/225(VOUTP_WiperFixMode_flg) -> bus_creator/225
  bus_selector3/162 -> outpmodule/340(VBCM_HMIKey2FuncSta_enum)  "<VBCM_HMIKey2FuncSta_enum>"
  outpmodule/222(VOUTP_FrWiperH_flg) -> bus_creator/222
  outpmodule/221(VOUTP_FrWiperL_flg) -> bus_creator/221
  outpmodule/216(VOUTP_RrDefog_flg) -> bus_creator/216
  outpmodule/215(VOUTP_MirrorDefog_flg) -> bus_creator/215
  outpmodule/741(VOUTP_RRWheelTemp_C) -> bus_creator/741
  outpmodule/214(VOUTP_MirrorCtrl_enum) -> bus_creator/214
  outpmodule/132(VOUTP_EPBExtApplyAvailTimeOut_flg) -> bus_creator/132
  outpmodule/121(VOUTP_BrkSwSta_flg) -> bus_creator/121
  outpmodule/212(VOUTP_RTurnLP_flg) -> bus_creator/212
  outpmodule/211(VOUTP_LTurnLP_flg) -> bus_creator/211
  outpmodule/460(VOUTP_Shifter1RCErrDTC_raw32) -> bus_creator/460
  bus_selector2/164 -> outpmodule/167(VAPM_DKCParkingModeCmd_enum)  "<VAPM_DKCParkingModeCmd_enum>"
  bus_selector3/136 -> outpmodule/314(VBCM_FollowMeENFunSta_flg)  "<VBCM_FollowMeENFunSta_flg>"
  outpmodule/205(VOUTP_ReverseLamp_flg) -> bus_creator/205
  outpmodule/201(VOUTP_LBeam_flg) -> bus_creator/201
  bus_selector3/61 -> outpmodule/239(VBCM_AmbLightColor2_enum)  "<VBCM_AmbLightColor2_enum>"
  bus_selector13/43 -> outpmodule/869(VTQD_ActParkRequest_flg)  "<VTQD_ActParkRequest_flg>"
  outpmodule/200(VOUTP_PosLamp_flg) -> bus_creator/200
  bus_selector12/3 -> outpmodule/732(VTPM_LRBatWarn_flg)  "<VTPM_LRBatWarn_flg>"
  outpmodule/727(VOUTP_EWPBUflag1_flg) -> bus_creator/727
  bus_selector11/75 -> outpmodule/720(VTHC_FDCFGSAirIntCmd_enum)  "<VTHC_FDCFGSAirIntCmd_enum>"
  bus_selector4/79 -> outpmodule/438(VDDM_FCM3NoComDTC_raw32)  "<VDDM_FCM3NoComDTC_raw32>"
  outpmodule/199(VOUTP_DimmerEN_flg) -> bus_creator/199
  outpmodule/196(VOUTP_DoorLockIND_flg) -> bus_creator/196
  outpmodule/726(VOUTP_FDCTHCMPreWPTCHeatSta_enum) -> bus_creator/726
  outpmodule/266(VOUTP_AmbColorSta_enum) -> bus_creator/266
  outpmodule/197(VOUTP_CTDLockSW_flg) -> bus_creator/197
  bus_selector3/12 -> outpmodule/190(VBCM_RRDoorSW_flg)  "<VBCM_RRDoorSW_flg>"
  bus_selector9/5 -> outpmodule/559(VPMM_ActiveDischargeReq_flg)  "<VPMM_ActiveDischargeReq_flg>"
  outpmodule/194(VOUTP_CrashDetd_flg) -> bus_creator/194
  bus_selector4/112 -> outpmodule/471(VDDM_RFBatwarnDTC_raw32)  "<VDDM_RFBatwarnDTC_raw32>"
  outpmodule/191(VOUTP_LockSetting_flg) -> bus_creator/191
  bus_selector11/55 -> outpmodule/700(VTHC_FDCTHCPsEVentModeSta_enum)  "<VTHC_FDCTHCPsEVentModeSta_enum>"
  outpmodule/192(VOUTP_FrChargingDoorCtrl_enum) -> bus_creator/192
  outpmodule/750(VOUTP_TPMSResButtAllow_flg) -> bus_creator/750
  outpmodule/136(VOUTP_EPBStaTimeOut_flg) -> bus_creator/136
  outpmodule/188(VOUTP_PsDoorSW_flg) -> bus_creator/188
  bus_selector16/94 -> outpmodule/983(VVMC_APSDecReqA_flg)  "<VVMC_APSDecReqA_flg>"
  bus_selector9/34 -> outpmodule/588(VPMM_LVSilentChrgSta_enum)  "<VPMM_LVSilentChrgSta_enum>"
  outpmodule/185(VOUTP_HoodSW_flg) -> bus_creator/185
  bus_selector11/22 -> outpmodule/667(VTHC_CabinMode_enum)  "<VTHC_CabinMode_enum>"
  outpmodule/499(VOUTP_HVRlyOpFail_flg) -> bus_creator/499
  outpmodule/218(VOUTP_RoomLampL_flg) -> bus_creator/218
  outpmodule/183(VOUTP_BCMDoorLockSta_flg) -> bus_creator/183
  outpmodule/178(VOUTP_IVIUserTakeOverAPSSta_flg) -> bus_creator/178
  outpmodule/773(VOUTP_S3ID_raw32) -> bus_creator/773
  bus_selector11/14 -> outpmodule/659(VTHC_FDEWP2Cmd_enum)  "<VTHC_FDEWP2Cmd_enum>"
  outpmodule/179(VOUTP_AntitheftSta_enum) -> bus_creator/179
  outpmodule/220(VOUTP_TailgateHDSW_flg) -> bus_creator/220
  outpmodule/175(VOUTP_APSPwrReq_enum) -> bus_creator/175
  outpmodule/494(VOUTP_DisengagePFail_flg) -> bus_creator/494
  outpmodule/172(VOUTP_APSVMCReqA_flg) -> bus_creator/172
  outpmodule/171(VOUTP_APSSpeedCMD_kph) -> bus_creator/171
  outpmodule/456(VOUTP_MCUF1RCErrDTC_raw32) -> bus_creator/456
  outpmodule/208(VOUTP_LBSD_flg) -> bus_creator/208
  bus_selector4/18 -> outpmodule/377(VDDM_Lv3ErrDTC_raw32)  "<VDDM_Lv3ErrDTC_raw32>"
  outpmodule/231(VOUTP_AmbLightBreath6_enum) -> bus_creator/231
  outpmodule/230(VOUTP_AmbLightBreath5_enum) -> bus_creator/230
  outpmodule/820(VOUTP_FlashIDvalid_enum) -> bus_creator/820
  bus_selector7/1 -> outpmodule/539(VDSC_DISCTurn_flg)  "<VDSC_DISCTurn_flg>"
  outpmodule/743(VOUTP_RFSensorFail_flg) -> bus_creator/743
  outpmodule/229(VOUTP_AmbLightBreath4_enum) -> bus_creator/229
  outpmodule/561(VOUTP_DCDCVoltSetpoint_V) -> bus_creator/561
  bus_selector4/81 -> outpmodule/440(VDDM_FCM3CSErrDTC_raw32)  "<VDDM_FCM3CSErrDTC_raw32>"
  outpmodule/558(VOUTP_PowerDownFault_enum) -> bus_creator/558
  outpmodule/273(VOUTP_AmbWelENFlash_enum) -> bus_creator/273
  outpmodule/217(VOUTP_RoomLampH_flg) -> bus_creator/217
  bus_selector3/70 -> outpmodule/248(VBCM_IVIRST_flg)  "<VBCM_IVIRST_flg>"
  bus_selector11/44 -> outpmodule/689(VTHC_FaceM_flg)  "<VTHC_FaceM_flg>"
  outpmodule/555(VOUTP_PowerUpState_enum) -> bus_creator/555
  outpmodule/275(VOUTP_AmbLinkDriStaFlash_enum) -> bus_creator/275
  outpmodule/553(VOUTP_SysNMmSta_enum) -> bus_creator/553
  bus_selector3/82 -> outpmodule/260(VBCM_AmbFunEN_flg)  "<VBCM_AmbFunEN_flg>"
  outpmodule/281(VOUTP_AmbColorSta4_enum) -> bus_creator/281
  outpmodule/207(VOUTP_RDRL_flg) -> bus_creator/207
  outpmodule/554(VOUTP_NetworkReq_flg) -> bus_creator/554
  bus_selector12/63 -> outpmodule/792(VTPM_ID3messageALTU_raw8)  "<VTPM_ID3messageALTU_raw8>"
  outpmodule/548(VOUTP_NodeID_enum) -> bus_creator/548
  bus_selector3/88 -> outpmodule/266(VBCM_AmbColorSta_enum)  "<VBCM_AmbColorSta_enum>"
  outpmodule/546(VOUTP_CSB_flg) -> bus_creator/546
  bus_selector4/20 -> outpmodule/379(VDDM_BrkSWErrDTC_raw32)  "<VDDM_BrkSWErrDTC_raw32>"
  bus_selector16/43 -> outpmodule/932(VVMC_ACCJerkLowerLimit_mps3)  "<VVMC_ACCJerkLowerLimit_mps3>"
  outpmodule/545(VOUTP_Awake_enum) -> bus_creator/545
  outpmodule/544(VOUTP_NMmTxReq_flg) -> bus_creator/544
  bus_selector4/14 -> outpmodule/373(VDDM_C1ABM1CSDTC_raw32)  "<VDDM_C1ABM1CSDTC_raw32>"
  outpmodule/977(VOUTP_TimeGapCalcu_s) -> bus_creator/977
  bus_selector2/105 -> outpmodule/108(VAPM_LatAccelTimeOut_flg)  "<VAPM_LatAccelTimeOut_flg>"
  outpmodule/254(VOUTP_PTGInnerSW2_enum) -> bus_creator/254
  outpmodule/126(VOUTP_ESCStandstillTimeOut_flg) -> bus_creator/126
  outpmodule/541(VOUTP_DISCSta_enum) -> bus_creator/541
  bus_selector4/47 -> outpmodule/406(VDDM_EDriveSysErrVCUErr_flg)  "<VDDM_EDriveSysErrVCUErr_flg>"
  outpmodule/537(VOUTP_KeyTypeSta_enum) -> bus_creator/537
  outpmodule/841(VOUTP_FrEDUActTq_Nm) -> bus_creator/841
  outpmodule/536(VOUTP_KeyNumSta_enum) -> bus_creator/536
  outpmodule/531(VOUTP_KeyAreaPTG_enum) -> bus_creator/531
  outpmodule/177(VOUTP_RAPSErrLv1_flg) -> bus_creator/177
  bus_selector4/72 -> outpmodule/431(VDDM_FLLUSSDTC_raw32)  "<VDDM_FLLUSSDTC_raw32>"
  outpmodule/235(VOUTP_AmbLightBrightness4_enum) -> bus_creator/235
  outpmodule/529(VOUTP_PCommandToBCM_enum) -> bus_creator/529
  outpmodule/283(VOUTP_AmbColorSta7_enum) -> bus_creator/283
  outpmodule/523(VOUTP_TimeSNDKCFbk_cnt) -> bus_creator/523
  bus_selector4/74 -> outpmodule/433(VDDM_RLLUSSDTC_raw32)  "<VDDM_RLLUSSDTC_raw32>"
  outpmodule/521(VOUTP_DKCTimeSN_cnt) -> bus_creator/521
  outpmodule/293(VOUTP_FWipSwSta_enum) -> bus_creator/293
  outpmodule/519(VOUTP_EAPS1NRM_pct) -> bus_creator/519
  bus_selector9/40 -> outpmodule/594(VPMM_CtrlFrEDUINVERTER_flg)  "<VPMM_CtrlFrEDUINVERTER_flg>"
  outpmodule/518(VOUTP_ResetPedalZeroPosStart_flg) -> bus_creator/518
  bus_selector4/150 -> outpmodule/509(VDDM_CAN1BusErrorDTC_raw32)  "<VDDM_CAN1BusErrorDTC_raw32>"
  outpmodule/517(VOUTP_EAPS2MIN_pct) -> bus_creator/517
  outpmodule/513(VOUTP_CAN5BusErrorDTC_raw32) -> bus_creator/513
  bus_selector12/68 -> outpmodule/797(VTPM_ChkStorge_flg)  "<VTPM_ChkStorge_flg>"
  outpmodule/189(VOUTP_RLDoorSW_flg) -> bus_creator/189
  bus_selector3/63 -> outpmodule/241(VBCM_AmbLightColor4_enum)  "<VBCM_AmbLightColor4_enum>"
  outpmodule/973(VOUTP_FCMLDWRequest_enum) -> bus_creator/973
  bus_selector3/124 -> outpmodule/302(VBCM_FDLHandleLampCmd_flg)  "<VBCM_FDLHandleLampCmd_flg>"
  outpmodule/515(VOUTP_ActAPSPosn_pct) -> bus_creator/515
  outpmodule/514(VOUTP_CAN6BusErrorDTC_raw32) -> bus_creator/514
  bus_selector2/77 -> outpmodule/80(VAPM_LFPulseCountTimeOut_flg)  "<VAPM_LFPulseCountTimeOut_flg>"
  bus_selector2/40 -> outpmodule/43(VAPM_StaFSya_flg)  "<VAPM_StaFSya_flg>"
  bus_selector4/26 -> outpmodule/385(VDDM_DCDC4PreDTC_raw32)  "<VDDM_DCDC4PreDTC_raw32>"
  outpmodule/785(VOUTP_IDin_raw32) -> bus_creator/785
  outpmodule/512(VOUTP_CAN4BusErrorDTC_raw32) -> bus_creator/512
  outpmodule/510(VOUTP_CAN2BusErrorDTC_raw32) -> bus_creator/510
  BTQR_outputs/1 -> bus_selector14/1
  outpmodule/508(VOUTP_VCUTailgateSWSta_flg) -> bus_creator/508
  outpmodule/507(VOUTP_VCUHoodSWSta_flg) -> bus_creator/507
  bus_selector3/42 -> outpmodule/220(VBCM_TailgateHDSW_flg)  "<VBCM_TailgateHDSW_flg>"
  bus_selector7/3 -> outpmodule/541(VDSC_DISCSta_enum)  "<VDSC_DISCSta_enum>"
  bus_selector3/154 -> outpmodule/332(VBCM_ACCLevelMem57_enum)  "<VBCM_ACCLevelMem57_enum>"
  outpmodule/505(VOUTP_VCURRDoorSta_flg) -> bus_creator/505
  outpmodule/506(VOUTP_SysAllowReadySta_flg) -> bus_creator/506
  bus_selector3/173 -> outpmodule/351(VBCM_PsRWdwReqAP_enum)  "<VBCM_PsRWdwReqAP_enum>"
  outpmodule/574(VOUTP_TCountSta_enum) -> bus_creator/574
  outpmodule/504(VOUTP_VCURLDoorSta_flg) -> bus_creator/504
  outpmodule/503(VOUTP_VCUFRDoorSta_flg) -> bus_creator/503
  outpmodule/210(VOUTP_HazardSW_flg) -> bus_creator/210
  bus_selector6/18 -> outpmodule/538(VDKC_FDCDKCAllowSleep_flg)  "<VDKC_FDCDKCAllowSleep_flg>"
  bus_selector11/61 -> outpmodule/706(VTHC_FDCTHCDrVentENSta_flg)  "<VTHC_FDCTHCDrVentENSta_flg>"
  outpmodule/573(VOUTP_PwrStaConstraint_enum) -> bus_creator/573
  outpmodule/826(VOUTP_ModelVersionChksum_raw) -> bus_creator/826
  outpmodule/571(VOUTP_DrSeatSta_enum) -> bus_creator/571
  bus_selector10/12 -> outpmodule/614(VSYS_Minor2_cnt)  "<VSYS_Minor2_cnt>"
  outpmodule/568(VOUTP_FrMCUEnaReq_flg) -> bus_creator/568
  outpmodule/489(VOUTP_EPBLockTODTC_raw32) -> bus_creator/489
  outpmodule/570(VOUTP_DrivetrainSelect_enum) -> bus_creator/570
  outpmodule/184(VOUTP_AntitheftSeatFlod_flg) -> bus_creator/184
  outpmodule/566(VOUTP_HVPwrSta_flg) -> bus_creator/566
  outpmodule/567(VOUTP_SysPowerMode_enum) -> bus_creator/567
  bus_selector3/103 -> outpmodule/281(VBCM_AmbColorSta4_enum)  "<VBCM_AmbColorSta4_enum>"
  outpmodule/565(VOUTP_LVPwrSta_flg) -> bus_creator/565
  bus_selector9/48 -> outpmodule/602(VPMM_PwrReqRAPSAvail_flg)  "<VPMM_PwrReqRAPSAvail_flg>"
  outpmodule/562(VOUTP_HVBatCnctReq_flg) -> bus_creator/562
  bus_selector6/8 -> outpmodule/528(VDKC_KeyAreaLockUnlock_enum)  "<VDKC_KeyAreaLockUnlock_enum>"
  outpmodule/2(VOUTP_LVBattVoltSta_enum) -> bus_creator/2
  outpmodule/119(VOUTP_MCPressureV_bar) -> bus_creator/119
  outpmodule/206(VOUTP_LDRL_flg) -> bus_creator/206
  outpmodule/60(VOUTP_LRRawWhlSpeedVTimeOut_flg) -> bus_creator/60
  outpmodule/59(VOUTP_LRRawWhlSpeedV_flg) -> bus_creator/59
  outpmodule/439(VOUTP_FCM3RCErrDTC_raw32) -> bus_creator/439
  bus_selector16/16 -> outpmodule/905(VVMC_LatAccCtrl_flg)  "<VVMC_LatAccCtrl_flg>"
  outpmodule/54(VOUTP_RRRawWhlSpeedTimeOut_flg) -> bus_creator/54
  bus_selector4/85 -> outpmodule/444(VDDM_FCM5CSErrDTC_raw32)  "<VDDM_FCM5CSErrDTC_raw32>"
  outpmodule/52(VOUTP_LRRawWhlSpeedTimeOut_flg) -> bus_creator/52
  outpmodule/465(VOUTP_ESC1CSErrDTC_raw32) -> bus_creator/465
  outpmodule/53(VOUTP_RRRawWhlSpeed_kph) -> bus_creator/53
  outpmodule/659(VOUTP_FDEWP2Cmd_enum) -> bus_creator/659
  bus_selector11/43 -> outpmodule/688(VTHC_Frost_flg)  "<VTHC_Frost_flg>"
  outpmodule/51(VOUTP_LRRawWhlSpeed_kph) -> bus_creator/51
  outpmodule/550(VOUTP_RptMsgReq_flg) -> bus_creator/550
  bus_selector9/28 -> outpmodule/582(VPMM_LVChrgHoldTtimer_s)  "<VPMM_LVChrgHoldTtimer_s>"
  bus_selector11/25 -> outpmodule/670(VTHC_CCUACMaxLampSts_flg)  "<VTHC_CCUACMaxLampSts_flg>"
  outpmodule/228(VOUTP_AmbLightBreath3_enum) -> bus_creator/228
  outpmodule/48(VOUTP_LFRawWhlSpeedTimeOut_flg) -> bus_creator/48
  outpmodule/473(VOUTP_RRBatwarnDTC_raw32) -> bus_creator/473
  bus_selector4/34 -> outpmodule/393(VDDM_HVRlyOpDTC_raw32)  "<VDDM_HVRlyOpDTC_raw32>"
  bus_selector15/4 -> outpmodule/886(VV2L_ReqOBCExtrV2LEna_enum)  "<VV2L_ReqOBCExtrV2LEna_enum>"
  bus_selector2/109 -> outpmodule/112(VAPM_MCPressureTimeOut_flg)  "<VAPM_MCPressureTimeOut_flg>"
  outpmodule/242(VOUTP_AmbLightColor5_enum) -> bus_creator/242
  outpmodule/770(VOUTP_RRSensorMode_flg) -> bus_creator/770
  outpmodule/728(VOUTP_EWPBUflag2_flg) -> bus_creator/728
  outpmodule/47(VOUTP_LFRawWhlSpeed_kph) -> bus_creator/47
  outpmodule/45(VOUTP_BrkPedalPos_pct) -> bus_creator/45
  bus_selector16/75 -> outpmodule/964(VVMC_LVDAWarning_flg)  "<VVMC_LVDAWarning_flg>"
  outpmodule/46(VOUTP_BrkPedalPosTimeOut_flg) -> bus_creator/46
  bus_selector3/156 -> outpmodule/334(VBCM_LLeftStaCmd_flg)  "<VBCM_LLeftStaCmd_flg>"
  outpmodule/477(VOUTP_RRPressIndiDTC_raw32) -> bus_creator/477
  bus_selector16/2 -> outpmodule/891(VVMC_VehicleSpeed_mph)  "<VVMC_VehicleSpeed_mph>"
  outpmodule/44(VOUTP_ModOperation_enum) -> bus_creator/44
  bus_selector4/125 -> outpmodule/484(VDDM_LRSensorFailDTC_raw32)  "<VDDM_LRSensorFailDTC_raw32>"
  outpmodule/41(VOUTP_Chime_enum) -> bus_creator/41
  outpmodule/42(VOUTP_SNSRLayout_enum) -> bus_creator/42
  outpmodule/433(VOUTP_RLLUSSDTC_raw32) -> bus_creator/433
  outpmodule/38(VOUTP_USSStaFLL_flg) -> bus_creator/38
  bus_selector3/71 -> outpmodule/249(VBCM_CountAlarm_enum)  "<VBCM_CountAlarm_enum>"
  bus_selector16/22 -> outpmodule/911(VVMC_ISOJerkLimit_mps3)  "<VVMC_ISOJerkLimit_mps3>"
  outpmodule/684(VOUTP_FDRecyAutoCmd_enum) -> bus_creator/684
  outpmodule/37(VOUTP_USSStaFLR_flg) -> bus_creator/37
  bus_selector12/62 -> outpmodule/791(VTPM_ID2messageALTU_raw8)  "<VTPM_ID2messageALTU_raw8>"
  bus_selector12/7 -> outpmodule/736(VTPM_LRWheelPress_raw8)  "<VTPM_LRWheelPress_raw8>"
  bus_selector16/63 -> outpmodule/952(VVMC_LKAHODSoundWarning_flg)  "<VVMC_LKAHODSoundWarning_flg>"
  outpmodule/36(VOUTP_USSStaFML_flg) -> bus_creator/36
  bus_selector16/70 -> outpmodule/959(VVMC_ADASFCWMute_flg)  "<VVMC_ADASFCWMute_flg>"
  outpmodule/404(VOUTP_HoodSWDTC_raw32) -> bus_creator/404
  outpmodule/35(VOUTP_USSStaFMR_flg) -> bus_creator/35
  outpmodule/860(VOUTP_RrIdcMin_A) -> bus_creator/860
  outpmodule/33(VOUTP_USSStaRCR_flg) -> bus_creator/33
  outpmodule/31(VOUTP_USSStaRLR_flg) -> bus_creator/31
  bus_selector10/8 -> outpmodule/610(VSYS_ECU2_cnt)  "<VSYS_ECU2_cnt>"
  outpmodule/30(VOUTP_USSStaRML_flg) -> bus_creator/30
  outpmodule/29(VOUTP_USSStaRMR_flg) -> bus_creator/29
  outpmodule/223(VOUTP_RrWiper_flg) -> bus_creator/223
  bus_selector2/63 -> outpmodule/66(VAPM_RFWhlRotDirTimeOut_flg)  "<VAPM_RFWhlRotDirTimeOut_flg>"
  bus_selector16/52 -> outpmodule/941(VVMC_ADASFCWSta_enum)  "<VVMC_ADASFCWSta_enum>"
  bus_selector2/148 -> outpmodule/151(VAPM_ABSActive_flg)  "<VAPM_ABSActive_flg>"
  outpmodule/26(VOUTP_PASAFMR_enum) -> bus_creator/26
  outpmodule/436(VOUTP_FCM2RCErrDTC_raw32) -> bus_creator/436
  outpmodule/27(VOUTP_PASAFML_enum) -> bus_creator/27
  outpmodule/24(VOUTP_PASARCR_enum) -> bus_creator/24
  outpmodule/21(VOUTP_PASAFCL_enum) -> bus_creator/21
  outpmodule/28(VOUTP_PASAFCR_enum) -> bus_creator/28
  outpmodule/22(VOUTP_PASARMR_enum) -> bus_creator/22
  outpmodule/995(VOUTP_CalibratedGyroX_Dps) -> bus_creator/995
  outpmodule/419(VOUTP_DiagFLTSDTC_raw32) -> bus_creator/419
  outpmodule/57(VOUTP_RFRawWhlSpeedV_flg) -> bus_creator/57
  bus_selector10/20 -> outpmodule/622(VSYS_Change2_cnt)  "<VSYS_Change2_cnt>"
  outpmodule/18(VOUTP_APSDRLL_cm) -> bus_creator/18
  bus_selector4/154 -> outpmodule/513(VDDM_CAN5BusErrorDTC_raw32)  "<VDDM_CAN5BusErrorDTC_raw32>"
  outpmodule/19(VOUTP_APSDFLR_cm) -> bus_creator/19
  bus_selector4/95 -> outpmodule/454(VDDM_MSAMalfuncDetDTC_raw32)  "<VDDM_MSAMalfuncDetDTC_raw32>"
  bus_selector2/80 -> outpmodule/83(VAPM_LRPulseCount_enum)  "<VAPM_LRPulseCount_enum>"
  outpmodule/50(VOUTP_RFRawWhlSpeedTimeOut_flg) -> bus_creator/50
  bus_selector4/80 -> outpmodule/439(VDDM_FCM3RCErrDTC_raw32)  "<VDDM_FCM3RCErrDTC_raw32>"
  outpmodule/445(VOUTP_ZoneSCPNoComDTC_raw32) -> bus_creator/445
  outpmodule/16(VOUTP_PASDFCL_cm) -> bus_creator/16
  outpmodule/936(VOUTP_ADASShftPosnReq_enum) -> bus_creator/936
  outpmodule/17(VOUTP_APSDRLR_cm) -> bus_creator/17
  outpmodule/540(VOUTP_DISCTargetSpd_kph) -> bus_creator/540
  outpmodule/14(VOUTP_PASDFML_cm) -> bus_creator/14
  outpmodule/12(VOUTP_PASDRCL_cm) -> bus_creator/12
  bus_selector9/44 -> outpmodule/598(VPMM_Sched_ChgTOSta_enum)  "<VPMM_Sched_ChgTOSta_enum>"
  outpmodule/135(VOUTP_EPBSta_enum) -> bus_creator/135
  outpmodule/124(VOUTP_BrkSwVTimeOut_flg) -> bus_creator/124
  outpmodule/13(VOUTP_PASDFMR_cm) -> bus_creator/13
  outpmodule/122(VOUTP_BrkSwStaTimeOut_flg) -> bus_creator/122
  outpmodule/11(VOUTP_PASDRCR_cm) -> bus_creator/11
  outpmodule/260(VOUTP_AmbFunEN_flg) -> bus_creator/260
  outpmodule/10(VOUTP_PASDRML_cm) -> bus_creator/10
  bus_selector11/10 -> outpmodule/655(VTHC_FDFrWPTCHeatPwrCmd_W)  "<VTHC_FDFrWPTCHeatPwrCmd_W>"
  outpmodule/134(VOUTP_EPBErrStaTimeOut_flg) -> bus_creator/134
  outpmodule/9(VOUTP_PASDRMR_cm) -> bus_creator/9
  outpmodule/7(VOUTP_FSOffSwTimeOut_flg) -> bus_creator/7
  outpmodule/673(VOUTP_sigWindDirZon1St_enum) -> bus_creator/673
  outpmodule/979(VOUTP_MSACtrlSta_enum) -> bus_creator/979
  outpmodule/526(VOUTP_DkeyShowIVISta_enum) -> bus_creator/526
  bus_selector2/140 -> outpmodule/143(VAPM_AVMErrSTA_flg)  "<VAPM_AVMErrSTA_flg>"
  outpmodule/6(VOUTP_FSOffSw_enum) -> bus_creator/6
  bus_selector4/41 -> outpmodule/400(VDDM_FLDoorSWDTC_raw32)  "<VDDM_FLDoorSWDTC_raw32>"
  outpmodule/5(VOUTP_VehSpeedTimeOut_flg) -> bus_creator/5
  outpmodule/4(VOUTP_VehSpeed_kph) -> bus_creator/4
  bus_selector3/46 -> outpmodule/224(VBCM_WasherCtrl_enum)  "<VBCM_WasherCtrl_enum>"
  outpmodule/716(VOUTP_PsVentEN_flg) -> bus_creator/716
  outpmodule/170(VOUTP_APSShiftPosnReq_enum) -> bus_creator/170
  outpmodule/755(VOUTP_RRPressIndi_enum) -> bus_creator/755
  outpmodule/3(VOUTP_VehHVPwrAvail4THCM_W) -> bus_creator/3
  bus_selector2/123 -> outpmodule/126(VAPM_ESCStandstillTimeOut_flg)  "<VAPM_ESCStandstillTimeOut_flg>"
  outpmodule/58(VOUTP_RFRawWhlSpeedVTimeOut_flg) -> bus_creator/58
  bus_selector4/2 -> outpmodule/361(VDDM_C3BMS6CSDTC_raw32)  "<VDDM_C3BMS6CSDTC_raw32>"
  outpmodule/710(VOUTP_FDCTHCPsVentENSta_flg) -> bus_creator/710
  bus_selector2/122 -> outpmodule/125(VAPM_ESCStandstill_flg)  "<VAPM_ESCStandstill_flg>"
  outpmodule/564(VOUTP_PowerSta_enum) -> bus_creator/564
  bus_selector2/121 -> outpmodule/124(VAPM_BrkSwVTimeOut_flg)  "<VAPM_BrkSwVTimeOut_flg>"
  outpmodule/516(VOUTP_EAPS1MIN_pct) -> bus_creator/516
  bus_selector12/85 -> outpmodule/814(VTPM_unlearnSfailvalid_enum)  "<VTPM_unlearnSfailvalid_enum>"
  bus_selector3/128 -> outpmodule/306(VBCM_WalkInUnLkENMem_enum)  "<VBCM_WalkInUnLkENMem_enum>"
  outpmodule/630(VOUTP_SHA7_cnt) -> bus_creator/630
  outpmodule/994(VOUTP_CalibratedAccZ_G) -> bus_creator/994
  bus_selector2/130 -> outpmodule/133(VAPM_EPBErrSta_enum)  "<VAPM_EPBErrSta_enum>"
  outpmodule/289(VOUTP_AmbBrightnessSta7_enum) -> bus_creator/289
  outpmodule/15(VOUTP_PASDFCR_cm) -> bus_creator/15
  outpmodule/23(VOUTP_PASARML_enum) -> bus_creator/23
  outpmodule/25(VOUTP_PASARCL_enum) -> bus_creator/25
  outpmodule/441(VOUTP_FCM4NoComDTC_raw32) -> bus_creator/441
  bus_selector2/98 -> outpmodule/101(VAPM_SASV_flg)  "<VAPM_SASV_flg>"
  bus_selector2/53 -> outpmodule/56(VAPM_LFRawWhlSpeedVTimeOut_flg)  "<VAPM_LFRawWhlSpeedVTimeOut_flg>"
  outpmodule/348(VOUTP_DrvWdwReqAP_enum) -> bus_creator/348
  outpmodule/498(VOUTP_LVSysErrPwrOutErr_flg) -> bus_creator/498
  outpmodule/906(VOUTP_SafetyCtrl_flg) -> bus_creator/906
  outpmodule/343(VOUTP_HMIKey5FuncSta_enum) -> bus_creator/343
  outpmodule/344(VOUTP_HMIKey6FuncSta_enum) -> bus_creator/344
  outpmodule/631(VOUTP_SHA8_cnt) -> bus_creator/631
  outpmodule/342(VOUTP_HMIKey4FuncSta_enum) -> bus_creator/342
  outpmodule/632(VOUTP_NvWriteReqRisingEdge_flg) -> bus_creator/632
  outpmodule/341(VOUTP_HMIKey3FuncSta_enum) -> bus_creator/341
  bus_selector2/94 -> outpmodule/97(VAPM_SASSpeedValid_flg)  "<VAPM_SASSpeedValid_flg>"
  outpmodule/340(VOUTP_HMIKey2FuncSta_enum) -> bus_creator/340
  outpmodule/991(VOUTP_ExtraMSACtrlSta_enum) -> bus_creator/991
  outpmodule/339(VOUTP_HMIKey1FuncSta_enum) -> bus_creator/339
  bus_selector3/142 -> outpmodule/320(VBCM_PTGUserHeight2_cnt)  "<VBCM_PTGUserHeight2_cnt>"
  outpmodule/1(VOUTP_HVTHCMSysAvail_enum) -> bus_creator/1
  outpmodule/338(VOUTP_AutoUnlockMem_enum) -> bus_creator/338
  outpmodule/790(VOUTP_ID1messageALTU_raw8) -> bus_creator/790
  outpmodule/551(VOUTP_WakeUp_enum) -> bus_creator/551
  bus_selector9/45 -> outpmodule/599(VPMM_PwrReq_OTA_enum)  "<VPMM_PwrReq_OTA_enum>"
  outpmodule/336(VOUTP_AutoLockMem_enum) -> bus_creator/336
  outpmodule/627(VOUTP_SHA4_cnt) -> bus_creator/627
  bus_selector2/138 -> outpmodule/141(VAPM_AVMParkingmode_enum)  "<VAPM_AVMParkingmode_enum>"
  bus_selector4/33 -> outpmodule/392(VDDM_DCDCDisDTC_raw32)  "<VDDM_DCDCDisDTC_raw32>"
  outpmodule/334(VOUTP_LLeftStaCmd_flg) -> bus_creator/334
  outpmodule/996(VOUTP_CalibratedGyroY_Dps) -> bus_creator/996
  bus_selector2/144 -> outpmodule/147(VAPM_CAASSw_enum)  "<VAPM_CAASSw_enum>"
  bus_selector4/50 -> outpmodule/409(VDDM_APS2SigOoRDTC_raw32)  "<VDDM_APS2SigOoRDTC_raw32>"
  outpmodule/366(VOUTP_C3CCU1RCDTC_raw32) -> bus_creator/366
  outpmodule/43(VOUTP_StaFSya_flg) -> bus_creator/43
  outpmodule/847(VOUTP_FrEDUSpdValid_flg) -> bus_creator/847
  bus_selector8/2 -> outpmodule/544(VNMM_NMmTxReq_flg)  "<VNMM_NMmTxReq_flg>"
  outpmodule/332(VOUTP_ACCLevelMem57_enum) -> bus_creator/332
  outpmodule/914(VOUTP_FeatArbitrFinal_enum) -> bus_creator/914
  bus_selector13/25 -> outpmodule/851(VTQD_RgnAbnorSta_flg)  "<VTQD_RgnAbnorSta_flg>"
  outpmodule/328(VOUTP_SenstivityPosnCmd_enum) -> bus_creator/328
  outpmodule/325(VOUTP_PTGOpenHeight12_enum) -> bus_creator/325
  outpmodule/34(VOUTP_USSStaRCL_flg) -> bus_creator/34
  bus_selector13/17 -> outpmodule/843(VTQD_FrEDURolRgnTq_Nm)  "<VTQD_FrEDURolRgnTq_Nm>"
  outpmodule/475(VOUTP_RFPressIndiDTC_raw32) -> bus_creator/475
  bus_selector3/45 -> outpmodule/223(VBCM_RrWiper_flg)  "<VBCM_RrWiper_flg>"
  outpmodule/326(VOUTP_PTGOpenHeight34_enum) -> bus_creator/326
  bus_selector2/107 -> outpmodule/110(VAPM_LongAccelTimeOut_flg)  "<VAPM_LongAccelTimeOut_flg>"
  outpmodule/255(VOUTP_DrvWdwCtrlCmd_pct) -> bus_creator/255
  bus_selector16/40 -> outpmodule/929(VVMC_TimeGapLevel_enum)  "<VVMC_TimeGapLevel_enum>"
  bus_selector2/145 -> outpmodule/148(VAPM_CAASSwTimeOut_flg)  "<VAPM_CAASSwTimeOut_flg>"
  outpmodule/319(VOUTP_PTGUserHeight1_cnt) -> bus_creator/319
  outpmodule/317(VOUTP_PTGOpenHeightSta_enum) -> bus_creator/317
  bus_selector10/2 -> outpmodule/604(VSYS_HWVer2_cnt)  "<VSYS_HWVer2_cnt>"
  outpmodule/315(VOUTP_HoodRelCmd_flg) -> bus_creator/315
  bus_selector12/1 -> outpmodule/730(VTPM_LFBatWarn_flg)  "<VTPM_LFBatWarn_flg>"
  outpmodule/316(VOUTP_WelcomeLight_enum) -> bus_creator/316
  bus_selector16/73 -> outpmodule/962(VVMC_LVDAMuteSta_enum)  "<VVMC_LVDAMuteSta_enum>"
  outpmodule/314(VOUTP_FollowMeENFunSta_flg) -> bus_creator/314
  bus_selector12/38 -> outpmodule/767(VTPM_LFSensorMode_flg)  "<VTPM_LFSensorMode_flg>"
  outpmodule/130(VOUTP_EPBExtReleaseAvailTimeOut_flg) -> bus_creator/130
  bus_selector11/8 -> outpmodule/653(VTHC_FDFWVCmd_flg)  "<VTHC_FDFWVCmd_flg>"
  outpmodule/313(VOUTP_RmLpModeENFunSta_flg) -> bus_creator/313
  outpmodule/533(VOUTP_UIDLowPowerSta_enum) -> bus_creator/533
  bus_selector4/118 -> outpmodule/477(VDDM_RRPressIndiDTC_raw32)  "<VDDM_RRPressIndiDTC_raw32>"
  bus_selector3/65 -> outpmodule/243(VBCM_AmbLightColor6_enum)  "<VBCM_AmbLightColor6_enum>"
  outpmodule/310(VOUTP_FollowMeENMem_enum) -> bus_creator/310
  bus_selector11/35 -> outpmodule/680(VTHC_sigCbnSolarRight_W)  "<VTHC_sigCbnSolarRight_W>"
  bus_selector12/77 -> outpmodule/806(VTPM_WriteChkRRID_raw)  "<VTPM_WriteChkRRID_raw>"
  bus_selector16/92 -> outpmodule/981(VVMC_APSActive_flg)  "<VVMC_APSActive_flg>"
  outpmodule/309(VOUTP_LockSettingStaMem_enum) -> bus_creator/309
  bus_selector3/81 -> outpmodule/259(VBCM_APMDoorControlSta_flg)  "<VBCM_APMDoorControlSta_flg>"
  bus_selector2/142 -> outpmodule/145(VAPM_IVIStatus_flg)  "<VAPM_IVIStatus_flg>"
  outpmodule/732(VOUTP_LRBatWarn_flg) -> bus_creator/732
  outpmodule/308(VOUTP_RmLpModeENMem_enum) -> bus_creator/308
  outpmodule/307(VOUTP_WalkOutLkENMem_enum) -> bus_creator/307
  outpmodule/525(VOUTP_KeyModeSta_enum) -> bus_creator/525
  outpmodule/127(VOUTP_ESCAPSSta_enum) -> bus_creator/127
  outpmodule/363(VOUTP_C3BMS1RCDTC_raw32) -> bus_creator/363
  bus_selector3/80 -> outpmodule/258(VBCM_PsRWdwCtrlCmd_pct)  "<VBCM_PsRWdwCtrlCmd_pct>"
  bus_selector16/95 -> outpmodule/984(VVMC_APSDecReq_mps2)  "<VVMC_APSDecReq_mps2>"
  outpmodule/365(VOUTP_C3BMS1LCDTC_raw32) -> bus_creator/365
  outpmodule/559(VOUTP_ActiveDischargeReq_flg) -> bus_creator/559
  outpmodule/921(VOUTP_ADASAEBReq_enum) -> bus_creator/921
  bus_selector12/50 -> outpmodule/779(VTPM_ALFin_flg)  "<VTPM_ALFin_flg>"
  bus_selector2/126 -> outpmodule/129(VAPM_EPBExtReleaseAvail_flg)  "<VAPM_EPBExtReleaseAvail_flg>"
  bus_selector4/89 -> outpmodule/448(VDDM_FrMCUSigErrDetDTC_raw32)  "<VDDM_FrMCUSigErrDetDTC_raw32>"
  outpmodule/362(VOUTP_C3BMS6LCDTC_raw32) -> bus_creator/362
  bus_selector3/48 -> outpmodule/226(VBCM_AmbLightBreath1_enum)  "<VBCM_AmbLightBreath1_enum>"
  bus_selector11/59 -> outpmodule/704(VTHC_FDCTHCCREVentZSta_enum)  "<VTHC_FDCTHCCREVentZSta_enum>"
  outpmodule/532(VOUTP_KeyAreaSPTGSta_enum) -> bus_creator/532
  outpmodule/359(VOUTP_FoxPiLampSta_enum) -> bus_creator/359
  outpmodule/411(VOUTP_MCUF1NoComDTC_raw32) -> bus_creator/411
  bus_selector12/29 -> outpmodule/758(VTPM_RFWheelTmpIndi_flg)  "<VTPM_RFWheelTmpIndi_flg>"
  bus_selector3/176 -> outpmodule/354(VBCM_WinLFOpenedSta_pct)  "<VBCM_WinLFOpenedSta_pct>"
  outpmodule/39(VOUTP_USSStaFCR_flg) -> bus_creator/39
  bus_selector2/175 -> outpmodule/178(VAPM_IVIUserTakeOverAPSSta_flg)  "<VAPM_IVIUserTakeOverAPSSta_flg>"
  outpmodule/360(VOUTP_C3BMS6RCDTC_raw32) -> bus_creator/360
  bus_selector4/124 -> outpmodule/483(VDDM_RFSensorFailDTC_raw32)  "<VDDM_RFSensorFailDTC_raw32>"
  outpmodule/174(VOUTP_RAPSBCMLockReq_flg) -> bus_creator/174
  outpmodule/358(VOUTP_FoxPiSwitchSta_enum) -> bus_creator/358
  outpmodule/479(VOUTP_RFWheelTmpHighDTC_raw32) -> bus_creator/479
  outpmodule/846(VOUTP_RrEDUSpd_rpm) -> bus_creator/846
  bus_selector3/174 -> outpmodule/352(VBCM_CLWinLockDrSta_flg)  "<VBCM_CLWinLockDrSta_flg>"
  outpmodule/357(VOUTP_WinRROpenedSta_pct) -> bus_creator/357
  bus_selector11/41 -> outpmodule/686(VTHC_Face_flg)  "<VTHC_Face_flg>"
  outpmodule/55(VOUTP_LFRawWhlSpeedV_flg) -> bus_creator/55
  outpmodule/40(VOUTP_USSStaFCL_flg) -> bus_creator/40
  outpmodule/355(VOUTP_WinRFOpenedSta_pct) -> bus_creator/355
  bus_selector2/113 -> outpmodule/116(VAPM_LatAccelVTimeOut_flg)  "<VAPM_LatAccelVTimeOut_flg>"
  outpmodule/353(VOUTP_CLWinLockDrStaMem_enum) -> bus_creator/353
  bus_selector4/93 -> outpmodule/452(VDDM_ACCMalfuncDetDTC_raw32)  "<VDDM_ACCMalfuncDetDTC_raw32>"
  bus_selector11/27 -> outpmodule/672(VTHC_sigAirIntenZon1St_enum)  "<VTHC_sigAirIntenZon1St_enum>"
  bus_selector11/73 -> outpmodule/718(VTHC_FDCFGSAirIntSta_enum)  "<VTHC_FDCFGSAirIntSta_enum>"
  outpmodule/350(VOUTP_DrRWdwReqAP_enum) -> bus_creator/350
  outpmodule/56(VOUTP_LFRawWhlSpeedVTimeOut_flg) -> bus_creator/56
  outpmodule/202(VOUTP_HBeam_flg) -> bus_creator/202
  outpmodule/592(VOUTP_CtrlFrRC1_flg) -> bus_creator/592
  outpmodule/891(VOUTP_VehicleSpeed_mph) -> bus_creator/891
  outpmodule/486(VOUTP_C1EPAS2LCDTC_raw32) -> bus_creator/486
  outpmodule/590(VOUTP_LVSilentChrgLv_enum) -> bus_creator/590
  outpmodule/323(VOUTP_PTGUserHeight5_cnt) -> bus_creator/323
  outpmodule/588(VOUTP_LVSilentChrgSta_enum) -> bus_creator/588
  outpmodule/800(VOUTP_RFPind_enum) -> bus_creator/800
  outpmodule/376(VOUTP_Lv2ErrDTC_raw32) -> bus_creator/376
  outpmodule/589(VOUTP_LVSilentChrgReq_flg) -> bus_creator/589
  bus_selector2/174 -> outpmodule/177(VAPM_RAPSErrLv1_flg)  "<VAPM_RAPSErrLv1_flg>"
  outpmodule/584(VOUTP_SilentChkAllowSleep_flg) -> bus_creator/584
  outpmodule/585(VOUTP_TimerAllowSleep_flg) -> bus_creator/585
  outpmodule/198(VOUTP_Dimmer_pct) -> bus_creator/198
  outpmodule/719(VOUTP_FDCFGSChSta_enum) -> bus_creator/719
  outpmodule/581(VOUTP_IVIPwrStaONTOPopT_s) -> bus_creator/581
  bus_selector11/81 -> outpmodule/726(VTHC_FDCTHCMPreWPTCHeatSta_enum)  "<VTHC_FDCTHCMPreWPTCHeatSta_enum>"
  outpmodule/582(VOUTP_LVChrgHoldTtimer_s) -> bus_creator/582
  outpmodule/821(VOUTP_WritingCnt_enum) -> bus_creator/821
  outpmodule/391(VOUTP_MCUDisDTC_raw32) -> bus_creator/391
  outpmodule/347(VOUTP_AutoWipHSpdENSta_flg) -> bus_creator/347
  bus_selector16/59 -> outpmodule/948(VVMC_ADASCAMSpdLim_enum)  "<VVMC_ADASCAMSpdLim_enum>"
  bus_selector9/41 -> outpmodule/595(VPMM_HWResetSta_enum)  "<VPMM_HWResetSta_enum>"
  outpmodule/583(VOUTP_LVBattChrgTimeCnt_s) -> bus_creator/583
  outpmodule/474(VOUTP_LFPressIndiDTC_raw32) -> bus_creator/474
  bus_selector4/151 -> outpmodule/510(VDDM_CAN2BusErrorDTC_raw32)  "<VDDM_CAN2BusErrorDTC_raw32>"
  outpmodule/580(VOUTP_PwrStaONTOPopReq_flg) -> bus_creator/580
  outpmodule/579(VOUTP_EvccAplusPwrUpReq_flg) -> bus_creator/579
  bus_selector2/119 -> outpmodule/122(VAPM_BrkSwStaTimeOut_flg)  "<VAPM_BrkSwStaTimeOut_flg>"
  outpmodule/186(VOUTP_TailgateSW_flg) -> bus_creator/186
  outpmodule/543(VOUTP_AllCANTxReq_flg) -> bus_creator/543
  outpmodule/578(VOUTP_ReVehThdChkSta_enum) -> bus_creator/578
  outpmodule/907(VOUTP_SPD2ACCAct_flg) -> bus_creator/907
  bus_selector12/84 -> outpmodule/813(VTPM_unlearnSfali_flg)  "<VTPM_unlearnSfali_flg>"
  outpmodule/575(VOUTP_PwrUpReq_enum) -> bus_creator/575
